simulink model "SIM_EXO_DAL_MN"  (R2021b)
settings: Solver=VariableStepAuto  StartTime=0.0  StopTime=60  FixedStep=0.0001  RelTol=1e-4
undefined symbols (not defined in the file): b, dq, q, X, Y, Z
libraries: sm_lib x47, nesl_utility x7
(part 8 of 24)

== matlab function SIM_EXO_DAL_MN/Exoesqueleto/Dinámica Directa/Cdq ==
  data: dq input; C_dq output; q input
function C_dq = Cdq(dq,q)
%#codegen
dq1 = dq(1);
dq2 = dq(2);
dq3 = dq(3);
dq4 = dq(4);
dq5 = dq(5);
dq6 = dq(6);

q1 = q(1);
q2 = q(2);
q3 = q(3);
q4 = q(4);
q5 = q(5);
q6 = q(6);
%    This function was generated by the Symbolic Math Toolbox version 9.0.
%    02-Dec-2021 21:04:08

t2 = cos(q2);
t3 = cos(q4);
t4 = cos(q5);
t5 = cos(q6);
t6 = sin(q2);
t7 = sin(q4);
t8 = sin(q5);
t9 = sin(q6);
t10 = q1+q2;
t11 = q4.*2.0;
t12 = q5.*2.0;
t13 = q6.*2.0;
t34 = 9.007199254740992e+15;
t14 = cos(t11);
t15 = cos(t12);
t16 = cos(t13);
t17 = t3.^2;
t18 = t4.^2;
t19 = t5.^2;
t20 = sin(t12);
t21 = sin(t13);
t22 = t7.^2;
t23 = t8.^2;
t24 = t9.^2;
t25 = cos(t10);
t26 = sin(t10);
t32 = t4.*5.110348748545983e-1;
t33 = t8.*5.110348748545983e-1;
t39 = t4.*t7.*8.595599785252598e-1;
t40 = t3.*t9.*8.595599785252598e-1;
t41 = t5.*t7.*8.595599785252598e-1;
t42 = t7.*t8.*8.595599785252598e-1;
t43 = t7.*t9.*8.595599785252598e-1;
t44 = t4.*1.33637579258949e-4;
t45 = t5.*1.33637579258949e-4;
t46 = t8.*1.33637579258949e-4;
t47 = t9.*1.33637579258949e-4;
t48 = t4.*t5.*(-5.110348748545983e-1);
t49 = t3.*t5.*8.595599785252598e-1;
t50 = t8.*6.185538795558e-5;
t53 = t4.*1.35652529206996e-4;
t54 = t8.*1.35652529206996e-4;
t55 = t4.*6.185538795558e-5;
t57 = t4.*7.26350610236655e-5;
t58 = t5.*7.26350610236655e-5;
t59 = t8.*7.26350610236655e-5;
t60 = t9.*7.26350610236655e-5;
t70 = t8.*2.257319918256733e-6;
t71 = t5.*1.744166498897461e-6;
t72 = t9.*4.00912737776847e-7;
t73 = t9.*8.01825475553694e-7;
t74 = t9.*1.744166498897461e-6;
t75 = t5.*1.246862701090643e-6;
t76 = t9.*1.246862701090643e-6;
t77 = t4.*4.20092050615074e-6;
t78 = t4.*5.878412210495409e-7;
t79 = t4.*t9.*(-1.33637579258949e-4);
t80 = t8.*4.20092050615074e-6;
t81 = t8.*5.878412210495409e-7;
t82 = t8.*t9.*(-1.33637579258949e-4);
t83 = t5.*3.383302988283333e-6;
t84 = t9.*3.383302988283333e-6;
t85 = t3.*t5.*t8.*(-8.595599785252598e-1);
t86 = t4.*7.291452964015446e-7;
t87 = t4.*2.257319918256733e-6;
t88 = t7.*t8.*t9.*(-8.595599785252598e-1);
t89 = t8.*7.291452964015446e-7;
t104 = t4.*t5.*4.36041e-5;
t106 = t4.*t9.*4.36041e-5;
t107 = t5.*t8.*4.36041e-5;
t109 = t8.*t9.*4.36041e-5;
t111 = t4.*1.758766830582798e-8;
t112 = t5.*2.179051830709965e-7;
t113 = t5.*4.35810366141993e-7;
t114 = t8.*1.758766830582798e-8;
t115 = t4.*t5.*4.00912737776847e-7;
t116 = t4.*t5.*8.01825475553694e-7;
t118 = t5.*t8.*8.01825475553694e-7;
t122 = t4.*t5.*(-1.246862701090643e-6);
t123 = t4.*t9.*(-1.246862701090643e-6);
t124 = t8.*t9.*(-3.383302988283333e-6);
t126 = t4.*2.524706033578261e-9;
t128 = t8.*2.524706033578261e-9;
t129 = t5.*t8.*(-1.744166498897461e-6);
t130 = t8.*t9.*(-8.01825475553694e-7);
t132 = t4.*t9.*2.179051830709965e-7;
t133 = t4.*t9.*4.35810366141993e-7;
t135 = t8.*t9.*4.35810366141993e-7;
t136 = t4.*t5.*t8.*1.603650951107388e-6;
t139 = t4.*3.146556677756745e-13;
t140 = t5.*3.146556677756745e-13;
t141 = t8.*3.146556677756745e-13;
t142 = t9.*3.146556677756745e-13;
t145 = t4.*t8.*t9.*8.71620732283986e-7;
t147 = t4.*t5.*t8.*t9.*2.493725402181286e-6;
t150 = t4.*4.126305279697715e-13;
t151 = t5.*4.126305279697715e-13;
t153 = t8.*4.126305279697715e-13;
t154 = t9.*4.126305279697715e-13;
t159 = t4.*t5.*1.40259855e-11;
t160 = t4.*t9.*1.40259855e-11;
t161 = t5.*t8.*1.40259855e-11;
t162 = t4.*t8.*5.902365793397849e-7;
t163 = t8.*t9.*1.40259855e-11;
t165 = t8.*t9.*(-3.146556677756745e-13);
t176 = t4.*t9.*(-4.126305279697715e-13);
t177 = t5.*t8.*(-4.126305279697715e-13);
t179 = t4.*t5.*8.4155913e-14;
t180 = t4.*t9.*8.4155913e-14;
t181 = t5.*t8.*8.4155913e-14;
t182 = t8.*t9.*8.4155913e-14;
t187 = (q3.*t34)./4.503599627370496e+15;
t189 = (q3.*t34)./9.007199254740992e+15;
t206 = t8.*6.829346359246847e-5;
t207 = t4.*6.829346359246847e-5;
t215 = t3.*5.316841594276996e-5;
t216 = t7.*5.316841594276996e-5;
t218 = t4.*6.932317328700695e-5;
t219 = t3.*1.166014850920627e-4;
t220 = t8.*6.932317328700695e-5;
t221 = t7.*1.166014850920627e-4;
t222 = t4.*3.161026044296245e-5;
t224 = t3.*t4.*1.148695147579899e-4;
t225 = t3.*t5.*1.148695147579899e-4;
t226 = t8.*3.161026044296245e-5;
t228 = t4.*t7.*1.148695147579899e-4;
t229 = t3.*t9.*1.148695147579899e-4;
t230 = t5.*t7.*1.148695147579899e-4;
t231 = t4.*3.711904932028501e-5;
t233 = t7.*t8.*1.148695147579899e-4;
t234 = t8.*3.711904932028501e-5;
t235 = t4.*2.146816885134859e-6;
t236 = t8.*2.146816885134859e-6;
t237 = t4.*3.004073648334264e-7;
t238 = t8.*3.004073648334264e-7;
t239 = t9.*2.048803907774054e-7;
t240 = t9.*4.097607815548108e-7;
t243 = t8.*t9.*(-6.829346359246847e-5);
t245 = t4.*3.726186752973823e-7;
t247 = t8.*3.726186752973823e-7;
t251 = t4.*3.60334715805357e-7;
t252 = t8.*3.60334715805357e-7;
t255 = t4.*1.153569201933121e-6;
t259 = t8.*1.153569201933121e-6;
t260 = t4.*8.987911871652987e-9;
t261 = t3.*2.28624364216682e-6;
t262 = t8.*8.987911871652987e-9;
t263 = t7.*1.14312182108341e-6;
t264 = t7.*2.28624364216682e-6;
t273 = t4.*t7.*6.243419149368285e-5;
t274 = t3.*t9.*6.243419149368285e-5;
t275 = t7.*t8.*6.243419149368285e-5;
t276 = t7.*t9.*6.243419149368285e-5;
t277 = t5.*1.11357147960855e-7;
t278 = t5.*2.227142959217101e-7;
t279 = t7.*t8.*(-5.316841594276996e-5);
t280 = t4.*t5.*8.913299084896471e-7;
t282 = t4.*t5.*2.048803907774054e-7;
t283 = t4.*t9.*8.913299084896471e-7;
t284 = t5.*t8.*8.913299084896471e-7;
t291 = t4.*t5.*(-3.711904932028501e-5);
t292 = t4.*t7.*t9.*(-1.148695147579899e-4);
t293 = t5.*t7.*t8.*(-1.148695147579899e-4);
t294 = t7.*t8.*t9.*(-1.148695147579899e-4);
t295 = t3.*t4.*6.243419149368285e-5;
t296 = t3.*t5.*6.243419149368285e-5;
t297 = t4.*t9.*1.728985819212562e-6;
t298 = t8.*t9.*1.728985819212562e-6;
t300 = t4.*t5.*t8.*8.195215631096216e-7;
t301 = t4.*t5.*6.371903244127231e-7;
t305 = t4.*t9.*6.371903244127231e-7;
t306 = t5.*t8.*6.371903244127231e-7;
t307 = t3.*t8.*1.940301860461398e-6;
t308 = t4.*t7.*1.940301860461398e-6;
t309 = t3.*t9.*3.446085442739697e-7;
t310 = t5.*t7.*3.446085442739697e-7;
t311 = t8.*t9.*6.371903244127231e-7;
t312 = t7.*t8.*1.940301860461398e-6;
t313 = t3.*t4.*3.610943140053254e-6;
t314 = t4.*t7.*3.610943140053254e-6;
t315 = t7.*t8.*3.610943140053254e-6;
t316 = t3.*t5.*2.908151843953269e-6;
t317 = t3.*t4.*5.052847873416058e-7;
t319 = t3.*t9.*2.908151843953269e-6;
t320 = t5.*t7.*2.908151843953269e-6;
t321 = t4.*t7.*5.052847873416058e-7;
t322 = t3.*t5.*1.07175327657342e-6;
t323 = t7.*t8.*5.052847873416058e-7;
t324 = t3.*t9.*1.07175327657342e-6;
t325 = t5.*t7.*1.07175327657342e-6;
t326 = t3.*t5.*1.49921571833678e-6;
t328 = t7.*t9.*1.07175327657342e-6;
t329 = t3.*t4.*6.267441153167058e-7;
t330 = t3.*t9.*1.49921571833678e-6;
t331 = t3.*t8.*6.267441153167058e-7;
t332 = t4.*t7.*6.267441153167058e-7;
t333 = t7.*t9.*1.49921571833678e-6;
t334 = t7.*t8.*6.267441153167058e-7;
t335 = t3.*1.511765579126689e-8;
t336 = t4.*t5.*1.728985819212562e-6;
t338 = t7.*1.511765579126689e-8;
t339 = t4.*t9.*1.11357147960855e-7;
t341 = t3.*t4.*6.060825118201251e-7;
t342 = t3.*t8.*6.060825118201251e-7;
t343 = t4.*t7.*6.060825118201251e-7;
t345 = t7.*t8.*6.060825118201251e-7;
t350 = t4.*1.608000198040319e-13;
t351 = t4.*1.290212831914316e-9;
t352 = t8.*1.608000198040319e-13;
t354 = t8.*1.290212831914316e-9;
t360 = t3.*2.170136264005124e-9;
t363 = t7.*2.170136264005124e-9;
t372 = t3.*t4.*t5.*3.446085442739697e-7;
t378 = t4.*t7.*t9.*6.892170885479394e-7;
t381 = t4.*t7.*t9.*2.908151843953269e-6;
t385 = t7.*t8.*t9.*2.908151843953269e-6;
t391 = t4.*t5.*t7.*1.49921571833678e-6;
t393 = t5.*t7.*t8.*1.49921571833678e-6;
t394 = t3.*t4.*7.558827895633446e-9;
t399 = t3.*t5.*1.873025744810486e-7;
t400 = t3.*t5.*t8.*(-6.243419149368285e-5);
t402 = t4.*t8.*t9.*4.454285918434201e-7;
t403 = t7.*t9.*1.873025744810486e-7;
t404 = t7.*t8.*t9.*(-6.243419149368285e-5);
t406 = t3.*t8.*t9.*(-3.446085442739697e-7);
t414 = t3.*t5.*t8.*(-1.07175327657342e-6);
t416 = t3.*t5.*t8.*(-1.49921571833678e-6);
t424 = t3.*t4.*(-1.511765579126689e-8);
t426 = t4.*t7.*(-1.511765579126689e-8);
t431 = t3.*t5.*t8.*t9.*7.044680628082447e-7;
t436 = t3.*t4.*t5.*t9.*2.143506553146841e-6;
t437 = t4.*t5.*(-1.608000198040319e-13);
t438 = t4.*t9.*(-1.608000198040319e-13);
t439 = t8.*t9.*(-1.608000198040319e-13);
t443 = t3.*t8.*(-2.170136264005124e-9);
t448 = t3.*t4.*t9.*1.873025744810486e-7;
t450 = t4.*t5.*t7.*3.746051489620971e-7;
t457 = t4.*t5.*t8.*t9.*1.274380648825446e-6;
t458 = t4.*t7.*t8.*t9.*(-6.892170885479394e-7);
t462 = t4.*t5.*7.16776774470491e-12;
t463 = t4.*2.10868590222219e-13;
t464 = t4.*t9.*7.16776774470491e-12;
t465 = t5.*t8.*7.16776774470491e-12;
t466 = t8.*2.10868590222219e-13;
t467 = t3.*t4.*2.7046541903611e-13;
t468 = t3.*t5.*2.7046541903611e-13;
t469 = t8.*t9.*7.16776774470491e-12;
t471 = t4.*t7.*2.7046541903611e-13;
t472 = t3.*t9.*2.7046541903611e-13;
t473 = t5.*t7.*1.35232709518055e-13;
t474 = t5.*t7.*2.7046541903611e-13;
t476 = t7.*t8.*2.7046541903611e-13;
t487 = t3.*t8.*5.347915701547076e-7;
t490 = t4.*t5.*t7.*t8.*t9.*1.408936125616489e-6;
t497 = t3.*t5.*1.205617579517561e-11;
t499 = t3.*t9.*1.205617579517561e-11;
t500 = t5.*t7.*1.205617579517561e-11;
t501 = t7.*t9.*1.205617579517561e-11;
t517 = t4.*t8.*3.016314764575132e-7;
t526 = t3.*t4.*3.546806877605634e-13;
t527 = t3.*t5.*3.546806877605634e-13;
t528 = t4.*t7.*3.546806877605634e-13;
t529 = t3.*t9.*3.546806877605634e-13;
t534 = t7.*t8.*3.546806877605634e-13;
t535 = t7.*t9.*1.773403438802817e-13;
t536 = t7.*t9.*3.546806877605634e-13;
t540 = t3.*t4.*t5.*1.35232709518055e-13;
t541 = t3.*t8.*t9.*1.35232709518055e-13;
t556 = t4.*t5.*(-2.10868590222219e-13);
t558 = t5.*t8.*(-2.10868590222219e-13);
t559 = t4.*t7.*t8.*t9.*5.4093083807222e-13;
t560 = t3.*t8.*t9.*(-2.7046541903611e-13);
t562 = t4.*t7.*t9.*(-2.7046541903611e-13);
t564 = t3.*t4.*t9.*1.773403438802817e-13;
t565 = t3.*t5.*t8.*1.773403438802817e-13;
t570 = t3.*t5.*t8.*(-1.205617579517561e-11);
t571 = t4.*t5.*t7.*(-1.205617579517561e-11);
t573 = t4.*t7.*t9.*(-1.205617579517561e-11);
t574 = t5.*t7.*t8.*(-1.205617579517561e-11);
t576 = t7.*t8.*t9.*(-1.205617579517561e-11);
t591 = t3.*t5.*t8.*(-3.546806877605634e-13);
t593 = t4.*t5.*t7.*(-3.546806877605634e-13);
t595 = t7.*t8.*t9.*(-3.546806877605634e-13);
t596 = t4.*t8.*t9.*(-2.10868590222219e-13);
t605 = t4.*t5.*t7.*t8.*7.093613755211269e-13;
t625 = t4.*t7.*t8.*1.253488085959302e-6;
t655 = t3.*2.625549359694895e-3;
t656 = t7.*2.625549359694895e-3;
t659 = t4.*1.560969940408669e-3;
t660 = t8.*1.560969940408669e-3;
t662 = t2.*t4.*1.324388487819695e-2;
t663 = t2.*t8.*1.324388487819695e-2;
t664 = t4.*t6.*1.324388487819695e-2;
t666 = t6.*t8.*1.324388487819695e-2;
t668 = t2.*t3.*2.227619671697157e-2;
t670 = t3.*t6.*2.227619671697157e-2;
t671 = t6.*t7.*2.227619671697157e-2;
t672 = t2.*t4.*5.463144604697158e-2;
t673 = t2.*t8.*5.463144604697158e-2;
t674 = t4.*t6.*5.463144604697158e-2;
t675 = t6.*t8.*5.463144604697158e-2;
t682 = t2.*t3.*9.189001945180305e-2;
t685 = t2.*t7.*9.189001945180305e-2;
t686 = t3.*t6.*9.189001945180305e-2;
t713 = t2.*t4.*t7.*2.227619671697157e-2;
t717 = t2.*t7.*t8.*2.227619671697157e-2;
t724 = t9.*2.094020497221851e-7;
t725 = t3.*5.363539617571206e-4;
t727 = t7.*5.363539617571206e-4;
t728 = t3.*t5.*(-2.625549359694895e-3);
t735 = t4.*t5.*(-1.560969940408669e-3);
t736 = t4.*t9.*(-1.560969940408669e-3);
t746 = t5.*t6.*t8.*(-1.324388487819695e-2);
t752 = t6.*t8.*t9.*(-1.324388487819695e-2);
t756 = t4.*t6.*t7.*9.189001945180305e-2;
t759 = t3.*t4.*t6.*(-2.227619671697157e-2);
t761 = t6.*t7.*t8.*9.189001945180305e-2;
t763 = t3.*t6.*t8.*(-2.227619671697157e-2);
t764 = t4.*t6.*t7.*(-2.227619671697157e-2);
t765 = t3.*t6.*t9.*(-2.227619671697157e-2);
t766 = t5.*t6.*t7.*(-2.227619671697157e-2);
t768 = t6.*t7.*t8.*(-2.227619671697157e-2);
t769 = t6.*t7.*t9.*(-2.227619671697157e-2);
t770 = t5.*t9.*4.280713835074992e-7;
t780 = t2.*t4.*t5.*(-5.463144604697158e-2);
t785 = t2.*t4.*t9.*(-5.463144604697158e-2);
t786 = t4.*t5.*t6.*(-5.463144604697158e-2);
t787 = t3.*3.050168925520967e-6;
t788 = t7.*3.050168925520967e-6;
t789 = t5.*1.138147723446811e-7;
t791 = t3.*6.689201101650821e-6;
t793 = t7.*6.689201101650821e-6;
t795 = t2.*t4.*t5.*(-1.324388487819695e-2);
t804 = t2.*t3.*t5.*(-9.189001945180305e-2);
t814 = t9.*5.924234258315089e-7;
t827 = t3.*t5.*3.294920660995711e-6;
t828 = t5.*t9.*1.211065105878372e-6;
t840 = t2.*t7.*t8.*t9.*(-2.227619671697157e-2);
t849 = t3.*t8.*(-5.363539617571206e-4);
t882 = t3.*t4.*7.725649335384969e-9;
t883 = t3.*t4.*7.725649335384969e-9;
t884 = t3.*t5.*t7.*4.188040994443703e-7;
t885 = t3.*t4.*t5.*3.522139685937468e-7;
t886 = t3.*t4.*t5.*3.522139685937468e-7;
t887 = t5.*3.219955937973119e-7;
t888 = t6.*t7.*t8.*t9.*(-9.189001945180305e-2);
t891 = t7.*t8.*7.725649335384969e-9;
t892 = t7.*t8.*7.725649335384969e-9;
t895 = t3.*t8.*t9.*3.522139685937468e-7;
t896 = t3.*t8.*t9.*3.522139685937468e-7;
t897 = t4.*t7.*t9.*3.522139685937468e-7;
t898 = t4.*t7.*t9.*3.522139685937468e-7;
t899 = t3.*t9.*1.79086425095906e-6;
t900 = t4.*t5.*t8.*7.660427522186475e-7;
t901 = t4.*t5.*t8.*7.660427522186475e-7;
t904 = t3.*t8.*(-3.050168925520967e-6);
t911 = t4.*t5.*t7.*3.294920660995711e-6;
t918 = t7.*t8.*t9.*3.294920660995711e-6;
t942 = t3.*t5.*t7.*t9.*1.302505910779267e-6;
t946 = t3.*t7.*t9.*2.276295446893622e-7;
t959 = t3.*t5.*t7.*1.184846851663018e-6;
t962 = t4.*t5.*t8.*t9.*1.191219491402018e-6;
t964 = t3.*t4.*t5.*t9.*2.190813206274814e-6;
t969 = t4.*t7.*t8.*t9.*7.044279371874937e-7;
t970 = t4.*t7.*t8.*t9.*7.044279371874937e-7;
t971 = t4.*t7.*t9.*1.79086425095906e-6;
t972 = t5.*t7.*t8.*1.79086425095906e-6;
t977 = t3.*t5.*t8.*t9.*7.200154966325453e-7;
t978 = t3.*t5.*t8.*t9.*7.200154966325453e-7;
t979 = t4.*t5.*t7.*t9.*7.200154966325453e-7;
t980 = t4.*t5.*t7.*t9.*7.200154966325453e-7;
t982 = t3.*t7.*t8.*4.593136418534343e-9;
t986 = t4.*t7.*1.075087193219284e-6;
t997 = t3.*t4.*3.476977846858022e-8;
t1001 = t3.*t8.*3.476977846858022e-8;
t1002 = t4.*t7.*3.476977846858022e-8;
t1005 = t7.*t8.*3.476977846858022e-8;
t1023 = t3.*t4.*t7.*t9.*2.094020497221851e-7;
t1024 = t3.*t5.*t7.*t8.*2.094020497221851e-7;
t1026 = t3.*t4.*t5.*t8.*7.044279371874937e-7;
t1027 = t3.*t4.*t5.*t8.*7.044279371874937e-7;
t1037 = t3.*t4.*t5.*t9.*2.190813206274814e-6;
t1044 = t3.*t4.*t5.*t7.*1.138147723446811e-7;
t1047 = t3.*t7.*t8.*t9.*1.138147723446811e-7;
t1050 = t3.*t7.*t8.*1.299453188729364e-8;
t1059 = t4.*t8.*t9.*4.163616429052617e-7;
t1060 = t4.*t8.*t9.*4.163616429052617e-7;
t1066 = t3.*t4.*t9.*1.914362954197335e-7;
t1067 = t3.*t4.*t9.*1.914362954197335e-7;
t1068 = t3.*t5.*t8.*1.914362954197335e-7;
t1069 = t3.*t5.*t8.*1.914362954197335e-7;
t1070 = t4.*t5.*t7.*1.914362954197335e-7;
t1071 = t4.*t5.*t7.*1.914362954197335e-7;
t1078 = t3.*t9.*1.38217261569615e-13;
t1079 = t3.*t9.*1.38217261569615e-13;
t1080 = t5.*t7.*1.38217261569615e-13;
t1081 = t5.*t7.*1.38217261569615e-13;
t1100 = t4.*t5.*t7.*t8.*t9.*1.440030993265091e-6;
t1101 = t4.*t5.*t7.*t8.*t9.*1.440030993265091e-6;
t1109 = t3.*t8.*5.465942862546103e-7;
t1110 = t3.*t8.*5.465942862546103e-7;
t1111 = t4.*t7.*5.465942862546103e-7;
t1112 = t4.*t7.*5.465942862546103e-7;
t1139 = t3.*t4.*t8.*t9.*3.828725908394669e-7;
t1140 = t3.*t4.*t8.*t9.*3.828725908394669e-7;
t1141 = t4.*t5.*t7.*t8.*3.828725908394669e-7;
t1142 = t4.*t5.*t7.*t8.*3.828725908394669e-7;
t1143 = t3.*t5.*t7.*t9.*3.684944893583304e-6;
t1154 = t3.*t4.*t7.*t9.*5.924234258315089e-7;
t1155 = t3.*t5.*t7.*t8.*5.924234258315089e-7;
t1158 = t4.*t7.*2.600171655979768e-6;
t1160 = t3.*t7.*t9.*6.439911875946239e-7;
t1167 = t3.*t4.*t5.*t7.*t9.*(-4.280713835074992e-7);
t1168 = t4.*t5.*t8.*t9.*1.191219491402018e-6;
t1169 = t3.*t4.*t5.*t8.*t9.*1.095406603137407e-6;
t1196 = t3.*t4.*t5.*t7.*t9.*(-1.211065105878372e-6);
t1204 = t3.*t4.*t5.*1.38217261569615e-13;
t1205 = t3.*t4.*t5.*1.38217261569615e-13;
t1229 = t3.*t4.*t5.*t8.*t9.*1.095406603137407e-6;
t1248 = t3.*t7.*1.035461175802946e-6;
t1250 = t3.*t4.*t5.*t7.*3.219955937973119e-7;
t1258 = t3.*t7.*t8.*t9.*3.219955937973119e-7;
t1259 = t3.*t8.*t9.*(-1.38217261569615e-13);
t1260 = t5.*t7.*t8.*(-1.38217261569615e-13);
t1261 = t5.*t7.*t8.*(-1.38217261569615e-13);
t1266 = t3.*t4.*t7.*3.249671339417237e-7;
t1272 = t4.*t8.*2.81948171692439e-7;
t1273 = t4.*t8.*2.81948171692439e-7;
t1282 = t7.*t8.*3.458197138188697e-13;
t1284 = t4.*t5.*t8.*1.503068317813338e-13;
t1285 = t4.*t5.*t8.*1.503068317813338e-13;
t1291 = t3.*t4.*t7.*9.193708611153409e-7;
t1302 = t4.*t7.*t8.*t9.*5.528690462784599e-13;
t1303 = t4.*t7.*t8.*t9.*5.528690462784599e-13;
t1304 = t3.*t5.*1.812542008830624e-13;
t1305 = t3.*t5.*1.812542008830624e-13;
t1307 = t3.*t4.*t7.*t9.*8.217441799717035e-14;
t1308 = t3.*t5.*t7.*t8.*8.217441799717035e-14;
t1313 = t7.*t9.*1.812542008830624e-13;
t1314 = t7.*t9.*1.812542008830624e-13;
t1332 = t3.*t7.*2.929443421869778e-6;
t1335 = t3.*t4.*t8.*2.592703454263624e-7;
t1336 = t3.*t4.*t8.*2.592703454263624e-7;
t1360 = t4.*t8.*t9.*1.97108120739817e-13;
t1361 = t4.*t8.*t9.*1.97108120739817e-13;
t1362 = t3.*t4.*t9.*1.812542008830624e-13;
t1363 = t3.*t4.*t9.*1.812542008830624e-13;
t1367 = t3.*t4.*t7.*t8.*t9.*1.643488359943407e-13;
t1371 = t3.*t4.*t5.*t7.*1.077612036149773e-13;
t1374 = t3.*t7.*t8.*t9.*1.077612036149773e-13;
t1380 = t3.*t4.*t7.*t9.*2.324812497785041e-13;
t1381 = t3.*t5.*t7.*t8.*2.324812497785041e-13;
t1389 = t4.*t5.*t7.*t8.*7.250168035322496e-13;
t1390 = t4.*t5.*t7.*t8.*7.250168035322496e-13;
t1393 = t3.*t5.*t8.*(-1.812542008830624e-13);
t1400 = t3.*t4.*t7.*t8.*t9.*4.649624995570082e-13;
t1409 = t3.*t4.*t5.*t7.*3.048693243547943e-13;
t1411 = t3.*t7.*t8.*t9.*3.048693243547943e-13;
t1416 = t3.*t4.*t5.*t7.*t8.*2.155224072299545e-13;
t1437 = t3.*t4.*t5.*t7.*t8.*6.097386487095885e-13;
t1449 = t7.*t8.*3.344600205005697e-6;
t1456 = t4.*t7.*t8.*1.281152254279884e-6;
t1457 = t4.*t7.*t8.*1.281152254279884e-6;
t1477 = t3.*t4.*t7.*t8.*3.808422322424164e-7;
t1485 = t3.*t4.*t7.*t8.*1.077448192248847e-6;
t1504 = t4.*2.086042441322004e-7;
t1505 = t8.*2.086042441322004e-7;
t1532 = t2.*t8.*1.769880715106441e-6;
t1533 = t4.*t6.*1.769880715106441e-6;
t1535 = t6.*t8.*1.769880715106441e-6;
t1547 = t4.*9.655440125097679e-8;
t1549 = t8.*9.655440125097679e-8;
t1552 = t4.*1.134411489642894e-5;
t1554 = t4.*1.133811468776912e-7;
t1558 = t8.*1.134411489642894e-5;
t1559 = t4.*2.117495204325297e-7;
t1560 = t8.*1.133811468776912e-7;
t1563 = t8.*2.117495204325297e-7;
t1596 = t2.*t4.*t9.*1.769880715106441e-6;
t1604 = t2.*t4.*7.30081420113316e-6;
t1606 = t4.*t5.*(-2.086042441322004e-7);
t1608 = t2.*t8.*7.30081420113316e-6;
t1610 = t6.*t8.*7.30081420113316e-6;
t1611 = t8.*t9.*(-2.086042441322004e-7);
t1612 = t8.*t9.*1.043021220661002e-7;
t1619 = t7.*4.911624408131596e-10;
t1631 = t3.*t4.*1.908078613917869e-5;
t1632 = t3.*t5.*1.908078613917869e-5;
t1637 = t4.*t7.*1.908078613917869e-5;
t1638 = t3.*t9.*1.908078613917869e-5;
t1639 = t5.*t7.*1.908078613917869e-5;
t1644 = t7.*t8.*1.908078613917869e-5;
t1645 = t7.*t9.*1.908078613917869e-5;
t1651 = t2.*t4.*t9.*8.849403575532204e-7;
t1652 = t3.*t4.*3.508720606545093e-7;
t1653 = t3.*t5.*3.508720606545093e-7;
t1654 = t3.*t5.*3.367638735295547e-6;
t1657 = t4.*t6.*t9.*(-1.769880715106441e-6);
t1658 = t4.*t7.*3.508720606545093e-7;
t1659 = t3.*t9.*1.754360303272547e-7;
C_dq = ft_1({dq1,dq2,dq3,dq4,dq5,dq6,t1001,t1002,t1005,t1023,t1024,t1026,t1027,t1037,t104,t1044,t1047,t1050,t1059,t106,t1060,t1066,t1067,t1068,t1069,t107,t1070,t1071,t1078,t1079,t1080,t1081,t109,t1100,t1101,t1109,t111,t1110,t1111,t1112,t112,t113,t1139,t114,t1140,t1141,t1142,t1143,t115,t1154,t1155,t1158,t116,t1160,t1167,t1168,t1169,t118,t1196,t1204,t1205,t122,t1229,t123,t124,t1248,t1250,t1258,t1259,t126,t1260,t1261,t1266,t1272,t1273,t128,t1282,t1284,t1285,t129,t1291,t130,t1302,t1303,t1304,t1305,t1307,t1308,t1313,t1314,t132,t133,t1332,t1335,t1336,t135,t136,t1360,t1361,t1362,t1363,t1367,t1371,t1374,t1380,t1381,t1389,t139,t1390,t1393,t14,t140,t1400,t1409,t141,t1411,t1416,t142,t1437,t1449,t145,t1456,t1457,t147,t1477,t1485,t15,t150,t1504,t1505,t151,t153,t1532,t1533,t1535,t154,t1547,t1549,t1552,t1554,t1558,t1559,t1560,t1563,t159,t1596,t16,t160,t1604,t1606,t1608,t161,t1610,t1611,t1612,t1619,t162,t163,t1631,t1632,t1637,t1638,t1639,t1644,t1645,t165,t1651,t1652,t1653,t1654,t1657,t1658,t1659,t17,t176,t177,t179,t18,t180,t181,t182,t187,t189,t19,t2,t20,t206,t207,t21,t215,t216,t218,t219,t22,t220,t221,t222,t224,t225,t226,t228,t229,t23,t230,t231,t233,t234,t235,t236,t237,t238,t239,t24,t240,t243,t245,t247,t25,t251,t252,t255,t259,t26,t260,t261,t262,t263,t264,t273,t274,t275,t276,t277,t278,t279,t280,t282,t283,t284,t291,t292,t293,t294,t295,t296,t297,t298,t3,t300,t301,t305,t306,t307,t308,t309,t310,t311,t312,t313,t314,t315,t316,t317,t319,t32,t320,t321,t322,t323,t324,t325,t326,t328,t329,t33,t330,t331,t332,t333,t334,t335,t336,t338,t339,t34,t341,t342,t343,t345,t350,t351,t352,t354,t360,t363,t372,t378,t381,t385,t39,t391,t393,t394,t399,t4,t40,t400,t402,t403,t404,t406,t41,t414,t416,t42,t424,t426,t43,t431,t436,t437,t438,t439,t44,t443,t448,t45,t450,t457,t458,t46,t462,t463,t464,t465,t466,t467,t468,t469,t47,t471,t472,t473,t474,t476,t48,t487,t49,t490,t497,t499,t5,t50,t500,t501,t517,t526,t527,t528,t529,t53,t534,t535,t536,t54,t540,t541,t55,t556,t558,t559,t560,t562,t564,t565,t57,t570,t571,t573,t574,t576,t58,t59,t591,t593,t595,t596,t6,t60,t605,t625,t655,t656,t659,t660,t662,t663,t664,t666,t668,t670,t671,t672,t673,t674,t675,t682,t685,t686,t7,t70,t71,t713,t717,t72,t724,t725,t727,t728,t73,t735,t736,t74,t746,t75,t752,t756,t759,t76,t761,t763,t764,t765,t766,t768,t769,t77,t770,t78,t780,t785,t786,t787,t788,t789,t79,t791,t793,t795,t8,t80,t804,t81,t814,t82,t827,t828,t83,t84,t840,t849,t85,t86,t87,t88,t882,t883,t884,t885,t886,t887,t888,t89,t891,t892,t895,t896,t897,t898,t899,t9,t900,t901,t904,t911,t918,t942,t946,t959,t962,t964,t969,t970,t971,t972,t977,t978,t979,t980,t982,t986,t997});
end
function C_dq = ft_1(ct)
dq1 = ct{1};
dq2 = ct{2};
dq3 = ct{3};
dq4 = ct{4};
dq5 = ct{5};
dq6 = ct{6};
t1001 = ct{7};
t1002 = ct{8};
t1005 = ct{9};
t1023 = ct{10};
t1024 = ct{11};
t1026 = ct{12};
t1027 = ct{13};
t1037 = ct{14};
t104 = ct{15};
t1044 = ct{16};
t1047 = ct{17};
t1050 = ct{18};
t1059 = ct{19};
t106 = ct{20};
t1060 = ct{21};
t1066 = ct{22};
t1067 = ct{23};
t1068 = ct{24};
t1069 = ct{25};
t107 = ct{26};
t1070 = ct{27};
t1071 = ct{28};
t1078 = ct{29};
t1079 = ct{30};
t1080 = ct{31};
t1081 = ct{32};
t109 = ct{33};
t1100 = ct{34};
t1101 = ct{35};
t1109 = ct{36};
t111 = ct{37};
t1110 = ct{38};
t1111 = ct{39};
t1112 = ct{40};
t112 = ct{41};
t113 = ct{42};
t1139 = ct{43};
t114 = ct{44};
t1140 = ct{45};
t1141 = ct{46};
t1142 = ct{47};
t1143 = ct{48};
t115 = ct{49};
t1154 = ct{50};
t1155 = ct{51};
t1158 = ct{52};
t116 = ct{53};
t1160 = ct{54};
t1167 = ct{55};
t1168 = ct{56};
t1169 = ct{57};
t118 = ct{58};
t1196 = ct{59};
t1204 = ct{60};
t1205 = ct{61};
t122 = ct{62};
t1229 = ct{63};
t123 = ct{64};
t124 = ct{65};
t1248 = ct{66};
t1250 = ct{67};
t1258 = ct{68};
t1259 = ct{69};
t126 = ct{70};
t1260 = ct{71};
t1261 = ct{72};
t1266 = ct{73};
t1272 = ct{74};
t1273 = ct{75};
t128 = ct{76};
t1282 = ct{77};
t1284 = ct{78};
t1285 = ct{79};
t129 = ct{80};
t1291 = ct{81};
t130 = ct{82};
t1302 = ct{83};
t1303 = ct{84};
t1304 = ct{85};
t1305 = ct{86};
t1307 = ct{87};
t1308 = ct{88};
t1313 = ct{89};
t1314 = ct{90};
t132 = ct{91};
t133 = ct{92};
t1332 = ct{93};
t1335 = ct{94};
t1336 = ct{95};
t135 = ct{96};
t136 = ct{97};
t1360 = ct{98};
t1361 = ct{99};
t1362 = ct{100};
t1363 = ct{101};
t1367 = ct{102};
t1371 = ct{103};
t1374 = ct{104};
t1380 = ct{105};
t1381 = ct{106};
t1389 = ct{107};
t139 = ct{108};
t1390 = ct{109};
t1393 = ct{110};
t14 = ct{111};
t140 = ct{112};
t1400 = ct{113};
t1409 = ct{114};
t141 = ct{115};
t1411 = ct{116};
t1416 = ct{117};
t142 = ct{118};
t1437 = ct{119};
t1449 = ct{120};
t145 = ct{121};
t1456 = ct{122};
t1457 = ct{123};
t147 = ct{124};
t1477 = ct{125};
t1485 = ct{126};
t15 = ct{127};
t150 = ct{128};
t1504 = ct{129};
t1505 = ct{130};
t151 = ct{131};
t153 = ct{132};
t1532 = ct{133};
t1533 = ct{134};
t1535 = ct{135};
t154 = ct{136};
t1547 = ct{137};
t1549 = ct{138};
t1552 = ct{139};
t1554 = ct{140};
t1558 = ct{141};
t1559 = ct{142};
t1560 = ct{143};
t1563 = ct{144};
t159 = ct{145};
t1596 = ct{146};
t16 = ct{147};
t160 = ct{148};
t1604 = ct{149};
t1606 = ct{150};
t1608 = ct{151};
t161 = ct{152};
t1610 = ct{153};
t1611 = ct{154};
t1612 = ct{155};
t1619 = ct{156};
t162 = ct{157};
t163 = ct{158};
t1631 = ct{159};
t1632 = ct{160};
t1637 = ct{161};
t1638 = ct{162};
t1639 = ct{163};
t1644 = ct{164};
t1645 = ct{165};
t165 = ct{166};
t1651 = ct{167};
t1652 = ct{168};
t1653 = ct{169};
t1654 = ct{170};
t1657 = ct{171};
t1658 = ct{172};
t1659 = ct{173};
t17 = ct{174};
t176 = ct{175};
t177 = ct{176};
t179 = ct{177};
t18 = ct{178};
t180 = ct{179};
t181 = ct{180};
t182 = ct{181};
t187 = ct{182};
t189 = ct{183};
t19 = ct{184};
t2 = ct{185};
t20 = ct{186};
t206 = ct{187};
t207 = ct{188};
t21 = ct{189};
t215 = ct{190};
t216 = ct{191};
t218 = ct{192};
t219 = ct{193};
t22 = ct{194};
t220 = ct{195};
t221 = ct{196};
t222 = ct{197};
t224 = ct{198};
t225 = ct{199};
t226 = ct{200};
t228 = ct{201};
t229 = ct{202};
t23 = ct{203};
t230 = ct{204};
t231 = ct{205};
t233 = ct{206};
t234 = ct{207};
t235 = ct{208};
t236 = ct{209};
t237 = ct{210};
t238 = ct{211};
t239 = ct{212};
t24 = ct{213};
t240 = ct{214};
t243 = ct{215};
t245 = ct{216};
t247 = ct{217};
t25 = ct{218};
t251 = ct{219};
t252 = ct{220};
t255 = ct{221};
t259 = ct{222};
t26 = ct{223};
t260 = ct{224};
t261 = ct{225};
t262 = ct{226};
t263 = ct{227};
t264 = ct{228};
t273 = ct{229};
t274 = ct{230};
t275 = ct{231};
t276 = ct{232};
t277 = ct{233};
t278 = ct{234};
t279 = ct{235};
t280 = ct{236};
t282 = ct{237};
t283 = ct{238};
t284 = ct{239};
t291 = ct{240};
t292 = ct{241};
t293 = ct{242};
t294 = ct{243};
t295 = ct{244};
t296 = ct{245};
t297 = ct{246};
t298 = ct{247};
t3 = ct{248};
t300 = ct{249};
t301 = ct{250};
t305 = ct{251};
t306 = ct{252};
t307 = ct{253};
t308 = ct{254};
t309 = ct{255};
t310 = ct{256};
t311 = ct{257};
t312 = ct{258};
t313 = ct{259};
t314 = ct{260};
t315 = ct{261};
t316 = ct{262};
t317 = ct{263};
t319 = ct{264};
t32 = ct{265};
t320 = ct{266};
t321 = ct{267};
t322 = ct{268};
t323 = ct{269};
t324 = ct{270};
t325 = ct{271};
t326 = ct{272};
t328 = ct{273};
t329 = ct{274};
t33 = ct{275};
t330 = ct{276};
t331 = ct{277};
t332 = ct{278};
t333 = ct{279};
t334 = ct{280};
t335 = ct{281};
t336 = ct{282};
t338 = ct{283};
t339 = ct{284};
t34 = ct{285};
t341 = ct{286};
t342 = ct{287};
t343 = ct{288};
t345 = ct{289};
t350 = ct{290};
t351 = ct{291};
t352 = ct{292};
t354 = ct{293};
t360 = ct{294};
t363 = ct{295};
t372 = ct{296};
t378 = ct{297};
t381 = ct{298};
t385 = ct{299};
t39 = ct{300};
t391 = ct{301};
t393 = ct{302};
t394 = ct{303};
t399 = ct{304};
t4 = ct{305};
t40 = ct{306};
t400 = ct{307};
t402 = ct{308};
t403 = ct{309};
t404 = ct{310};
t406 = ct{311};
t41 = ct{312};
t414 = ct{313};
t416 = ct{314};
t42 = ct{315};
t424 = ct{316};
t426 = ct{317};
t43 = ct{318};
t431 = ct{319};
t436 = ct{320};
t437 = ct{321};
t438 = ct{322};
t439 = ct{323};
t44 = ct{324};
t443 = ct{325};
t448 = ct{326};
t45 = ct{327};
t450 = ct{328};
t457 = ct{329};
t458 = ct{330};
t46 = ct{331};
t462 = ct{332};
t463 = ct{333};
t464 = ct{334};
t465 = ct{335};
t466 = ct{336};
t467 = ct{337};
t468 = ct{338};
t469 = ct{339};
t47 = ct{340};
t471 = ct{341};
t472 = ct{342};
t473 = ct{343};
t474 = ct{344};
t476 = ct{345};
t48 = ct{346};
t487 = ct{347};
t49 = ct{348};
t490 = ct{349};
t497 = ct{350};
t499 = ct{351};
t5 = ct{352};
t50 = ct{353};
t500 = ct{354};
t501 = ct{355};
t517 = ct{356};
t526 = ct{357};
t527 = ct{358};
t528 = ct{359};
t529 = ct{360};
t53 = ct{361};
t534 = ct{362};
t535 = ct{363};
t536 = ct{364};
t54 = ct{365};
t540 = ct{366};
t541 = ct{367};
t55 = ct{368};
t556 = ct{369};
t558 = ct{370};
t559 = ct{371};
t560 = ct{372};
t562 = ct{373};
t564 = ct{374};
t565 = ct{375};
t57 = ct{376};
t570 = ct{377};
t571 = ct{378};
t573 = ct{379};
t574 = ct{380};
t576 = ct{381};
t58 = ct{382};
t59 = ct{383};
t591 = ct{384};
t593 = ct{385};
t595 = ct{386};
t596 = ct{387};
t6 = ct{388};
t60 = ct{389};
t605 = ct{390};
t625 = ct{391};
t655 = ct{392};
t656 = ct{393};
t659 = ct{394};
t660 = ct{395};
t662 = ct{396};
t663 = ct{397};
t664 = ct{398};
t666 = ct{399};
t668 = ct{400};
t670 = ct{401};
t671 = ct{402};
t672 = ct{403};
t673 = ct{404};
t674 = ct{405};
t675 = ct{406};
t682 = ct{407};
t685 = ct{408};
t686 = ct{409};
t7 = ct{410};
t70 = ct{411};
t71 = ct{412};
t713 = ct{413};
t717 = ct{414};
t72 = ct{415};
t724 = ct{416};
t725 = ct{417};
t727 = ct{418};
t728 = ct{419};
t73 = ct{420};
t735 = ct{421};
t736 = ct{422};
t74 = ct{423};
t746 = ct{424};
t75 = ct{425};
t752 = ct{426};
t756 = ct{427};
t759 = ct{428};
t76 = ct{429};
t761 = ct{430};
t763 = ct{431};
t764 = ct{432};
t765 = ct{433};
t766 = ct{434};
t768 = ct{435};
t769 = ct{436};
t77 = ct{437};
t770 = ct{438};
t78 = ct{439};
t780 = ct{440};
t785 = ct{441};
t786 = ct{442};
t787 = ct{443};
t788 = ct{444};
t789 = ct{445};
t79 = ct{446};
t791 = ct{447};
t793 = ct{448};
t795 = ct{449};
t8 = ct{450};
t80 = ct{451};
t804 = ct{452};
t81 = ct{453};
t814 = ct{454};
t82 = ct{455};
t827 = ct{456};
t828 = ct{457};
t83 = ct{458};
t84 = ct{459};
t840 = ct{460};
t849 = ct{461};
t85 = ct{462};
t86 = ct{463};
t87 = ct{464};
t88 = ct{465};
t882 = ct{466};
t883 = ct{467};
t884 = ct{468};
t885 = ct{469};
t886 = ct{470};
t887 = ct{471};
t888 = ct{472};
t89 = ct{473};
t891 = ct{474};
t892 = ct{475};
t895 = ct{476};
t896 = ct{477};
t897 = ct{478};
t898 = ct{479};
t899 = ct{480};
t9 = ct{481};
t900 = ct{482};
t901 = ct{483};
t904 = ct{484};
t911 = ct{485};
t918 = ct{486};
t942 = ct{487};
t946 = ct{488};
t959 = ct{489};
t962 = ct{490};
t964 = ct{491};
t969 = ct{492};
t970 = ct{493};
t971 = ct{494};
t972 = ct{495};
t977 = ct{496};
t978 = ct{497};
t979 = ct{498};
t980 = ct{499};
t982 = ct{500};
t986 = ct{501};
t997 = ct{502};
t1660 = t3.*t9.*3.508720606545093e-7;
t1661 = t5.*t7.*1.754360303272547e-7;
t1662 = t5.*t7.*3.508720606545093e-7;
t1664 = t6.*t8.*t9.*8.849403575532204e-7;
t1666 = t7.*t8.*3.508720606545093e-7;
t1668 = t7.*t9.*3.367638735295547e-6;
t1676 = t4.*t6.*t7.*2.976937004352228e-6;
t1677 = t2.*t7.*t9.*2.976937004352228e-6;
t1678 = t3.*t6.*t9.*2.976937004352228e-6;
t1679 = t5.*t6.*t7.*1.488468502176114e-6;
t1680 = t5.*t6.*t7.*2.976937004352228e-6;
t1682 = t2.*t8.*9.619703863182361e-7;
t1683 = t4.*t6.*9.619703863182361e-7;
t1684 = t6.*t7.*t8.*2.976937004352228e-6;
t1685 = t6.*t7.*4.167215943261981e-9;
t1688 = t6.*t8.*9.619703863182361e-7;
t1689 = t3.*t4.*1.624043742404524e-7;
t1692 = t4.*t9.*5.664363865215817e-6;
t1693 = t5.*t8.*5.664363865215817e-6;
t1694 = t3.*t9.*1.830388176740875e-6;
t1695 = t5.*t7.*1.830388176740875e-6;
t1696 = t4.*t7.*1.624043742404524e-7;
t1698 = t7.*t8.*1.624043742404524e-7;
t1702 = t4.*t9.*6.045309697076603e-6;
t1703 = t5.*t8.*6.045309697076603e-6;
t1709 = t4.*t5.*(-1.134411489642894e-5);
t1712 = t4.*t5.*(-1.133811468776912e-7);
t1713 = t4.*t9.*(-1.134411489642894e-5);
t1714 = t2.*t4.*3.96815841743287e-6;
t1716 = t4.*t9.*(-1.133811468776912e-7);
t1717 = t5.*t8.*5.669057343884558e-8;
t1720 = t2.*t8.*3.96815841743287e-6;
t1722 = t6.*t8.*3.96815841743287e-6;
t1726 = t3.*t8.*3.561624112004214e-7;
t1727 = t4.*t7.*3.561624112004214e-7;
t1729 = t7.*t8.*3.561624112004214e-7;
t1734 = t2.*t8.*t9.*3.65040710056658e-6;
t1736 = t4.*t6.*t9.*3.65040710056658e-6;
t1737 = t4.*t6.*t9.*7.30081420113316e-6;
t1745 = t2.*t3.*t5.*1.488468502176114e-6;
t1746 = t2.*t3.*t5.*2.976937004352228e-6;
t1749 = t2.*t4.*t7.*2.976937004352228e-6;
t1750 = t3.*t4.*t6.*2.976937004352228e-6;
t1751 = t3.*t5.*t6.*2.976937004352228e-6;
t1752 = t2.*t3.*4.167215943261981e-9;
t1785 = t2.*t3.*t4.*1.22799597575967e-5;
t1786 = t2.*t3.*t5.*1.22799597575967e-5;
t1796 = t2.*t4.*t7.*1.22799597575967e-5;
t1797 = t2.*t3.*t9.*1.22799597575967e-5;
t1798 = t2.*t5.*t7.*6.139979878798348e-6;
t1799 = t2.*t5.*t7.*1.22799597575967e-5;
t1800 = t3.*t5.*t6.*6.139979878798348e-6;
t1801 = t3.*t5.*t6.*1.22799597575967e-5;
t1809 = t2.*t7.*t8.*1.22799597575967e-5;
t1810 = t4.*t6.*t7.*1.22799597575967e-5;
t1816 = t3.*t4.*t5.*1.754360303272547e-7;
t1819 = t6.*t7.*t9.*1.22799597575967e-5;
t1827 = t4.*t5.*t7.*3.367638735295547e-6;
t1829 = t2.*t4.*t5.*(-7.30081420113316e-6);
t1833 = t4.*t7.*t9.*1.754360303272547e-7;
t1838 = t3.*t5.*1.016820285479769e-5;
t1840 = t3.*t4.*1.907069379620846e-7;
t1841 = t3.*t5.*9.535346898104229e-8;
t1842 = t3.*t5.*1.907069379620846e-7;
t1849 = t2.*t8.*t9.*(-7.30081420113316e-6);
t1850 = t4.*t7.*1.907069379620846e-7;
t1851 = t3.*t9.*1.907069379620846e-7;
t1852 = t7.*t9.*1.016820285479769e-5;
t1857 = t7.*t8.*1.907069379620846e-7;
t1858 = t7.*t9.*9.535346898104229e-8;
t1859 = t7.*t9.*1.907069379620846e-7;
t1871 = t8.*t9.*3.285763190182237e-6;
t1873 = t4.*t7.*t9.*1.830388176740875e-6;
t1876 = t4.*t5.*3.078710474192051e-6;
t1881 = t2.*t8.*1.396693317797299e-6;
t1882 = t4.*t6.*1.396693317797299e-6;
t1883 = t8.*t9.*3.078710474192051e-6;
t1889 = t3.*t5.*t8.*(-1.908078613917869e-5);
t1895 = t2.*t5.*t8.*1.984079208716435e-6;
t1897 = t4.*t5.*t6.*1.984079208716435e-6;
t1898 = t4.*t5.*t6.*3.96815841743287e-6;
t1907 = t7.*t8.*t9.*(-1.908078613917869e-5);
t1911 = t2.*t4.*t7.*1.618032907912407e-6;
t1912 = t3.*t4.*t6.*1.618032907912407e-6;
t1913 = t2.*t3.*t9.*8.090164539562037e-7;
t1914 = t2.*t3.*t9.*1.618032907912407e-6;
t1915 = t2.*t5.*t7.*1.618032907912407e-6;
t1916 = t3.*t5.*t6.*1.618032907912407e-6;
t1923 = t4.*t6.*t7.*1.618032907912407e-6;
t1924 = t3.*t6.*t9.*1.618032907912407e-6;
t1925 = t2.*t7.*1.718989821069714e-8;
t1926 = t3.*t6.*1.718989821069714e-8;
t1931 = t6.*t7.*t8.*1.618032907912407e-6;
t1932 = t6.*t7.*t9.*8.090164539562037e-7;
t1933 = t6.*t7.*t9.*1.618032907912407e-6;
t1935 = t4.*t7.*t9.*(-3.508720606545093e-7);
t1939 = t7.*t8.*t9.*(-3.508720606545093e-7);
t1948 = t2.*t4.*t5.*4.809851931591181e-7;
t1949 = t2.*t4.*t5.*9.619703863182361e-7;
t1956 = t2.*t7.*t8.*t9.*1.488468502176114e-6;
t1958 = t3.*t6.*t8.*t9.*1.488468502176114e-6;
t1960 = t4.*t6.*t7.*t9.*1.488468502176114e-6;
t1963 = t4.*t5.*3.285763190182237e-6;
t1968 = t5.*t6.*t8.*4.809851931591181e-7;
t1977 = t5.*t7.*t8.*(-1.830388176740875e-6);
t1978 = t3.*t9.*5.526649307438591e-6;
t1979 = t5.*t7.*5.526649307438591e-6;
t1994 = t2.*t4.*t5.*(-3.96815841743287e-6);
t1995 = t2.*t3.*t8.*t9.*6.139979878798348e-6;
t1997 = t2.*t4.*t7.*t9.*6.139979878798348e-6;
t2003 = t2.*t4.*t9.*(-3.96815841743287e-6);
t2012 = t6.*t7.*t8.*t9.*6.139979878798348e-6;
t2022 = t3.*4.452917654948397e-7;
t2024 = t4.*t5.*t7.*1.016820285479769e-5;
t2025 = t8.*4.470006985551917e-6;
t2028 = t3.*t4.*t9.*9.535346898104229e-8;
t2032 = t4.*t5.*t7.*9.535346898104229e-8;
t2046 = t2.*t4.*5.761404326386517e-6;
t2056 = t3.*t4.*t5.*t6.*(-2.976937004352228e-6);
t2058 = t6.*t8.*5.761404326386517e-6;
t2063 = t2.*t3.*t4.*6.674437170347525e-6;
t2064 = t2.*t3.*t5.*6.674437170347525e-6;
t2065 = t2.*t7.*t8.*t9.*(-2.976937004352228e-6);
t2067 = t3.*t6.*t8.*t9.*(-2.976937004352228e-6);
t2070 = t5.*t6.*t7.*t8.*(-2.976937004352228e-6);
t2072 = t2.*t4.*t7.*6.674437170347525e-6;
t2073 = t2.*t3.*t9.*6.674437170347525e-6;
t2079 = t5.*t6.*t8.*(-9.619703863182361e-7);
t2081 = t2.*t7.*t8.*6.674437170347525e-6;
t2082 = t4.*t6.*t7.*6.674437170347525e-6;
t2083 = t2.*t7.*t9.*3.337218585173762e-6;
t2084 = t2.*t7.*t9.*6.674437170347525e-6;
t2085 = t3.*t6.*t9.*3.337218585173762e-6;
t2086 = t3.*t6.*t9.*6.674437170347525e-6;
t2087 = t5.*t6.*t7.*6.674437170347525e-6;
t2093 = t8.*4.770628656414461e-6;
t2094 = t3.*t4.*2.768890910755245e-7;
t2098 = t7.*t8.*2.768890910755245e-7;
t2100 = t2.*t4.*t7.*t9.*(-1.22799597575967e-5);
t2103 = t7.*1.422428293644824e-6;
t2104 = t2.*t7.*t8.*t9.*(-1.22799597575967e-5);
t2105 = t2.*t7.*3.778031034908185e-6;
t2106 = t3.*t6.*3.778031034908185e-6;
t2110 = t2.*t5.*t7.*t8.*8.090164539562037e-7;
t2113 = t3.*t5.*t6.*t8.*8.090164539562037e-7;
t2115 = t4.*t5.*t6.*t7.*8.090164539562037e-7;
t2117 = t6.*t7.*t8.*t9.*(-1.22799597575967e-5);
t2131 = t3.*t5.*t8.*(-1.907069379620846e-7);
t2132 = t3.*t5.*t8.*(-9.535346898104229e-8);
t2144 = t7.*t8.*t9.*(-1.016820285479769e-5);
t2156 = t7.*1.005302486347477e-5;
t2171 = t2.*t3.*t8.*2.349236299369594e-6;
t2172 = t2.*t4.*t7.*2.349236299369594e-6;
t2173 = t3.*t4.*t6.*2.349236299369594e-6;
t2175 = t3.*t4.*t6.*t9.*(-1.618032907912407e-6);
t2176 = t4.*t5.*t6.*t7.*(-1.618032907912407e-6);
t2179 = t3.*t8.*2.657556793628188e-6;
t2180 = t4.*t7.*2.657556793628188e-6;
t2182 = t5.*t6.*t7.*t8.*(-1.618032907912407e-6);
t2183 = t2.*t3.*1.558449809444963e-5;
t2188 = t6.*t7.*t8.*2.349236299369594e-6;
t2189 = t6.*t7.*t8.*t9.*(-1.618032907912407e-6);
t2194 = t6.*t7.*1.558449809444963e-5;
t2205 = t2.*t3.*t5.*t8.*3.337218585173762e-6;
t2207 = t2.*t4.*t5.*t7.*3.337218585173762e-6;
t2220 = t5.*t6.*t7.*t8.*3.337218585173762e-6;
t2223 = t3.*t4.*1.956869039552983e-7;
t2228 = t4.*t7.*t9.*5.526649307438591e-6;
t2265 = t2.*t3.*t5.*t8.*(-6.674437170347525e-6);
t2277 = t4.*t5.*2.189414175010785e-14;
t2279 = t4.*t9.*2.189414175010785e-14;
t2280 = t5.*t8.*2.189414175010785e-14;
t2281 = t3.*t8.*8.02419104298182e-6;
t2282 = t4.*t7.*8.02419104298182e-6;
t2285 = t8.*t9.*2.189414175010785e-14;
t2294 = t3.*3.237047710821912e-7;
t2302 = t2.*t3.*t4.*9.690674399615435e-6;
t2304 = t2.*t7.*t8.*9.690674399615435e-6;
t2305 = t3.*t6.*t8.*9.690674399615435e-6;
t2306 = t4.*t6.*t7.*9.690674399615435e-6;
t2321 = t2.*t4.*t5.*1.857585372652597e-13;
t2322 = t2.*t4.*t9.*1.857585372652597e-13;
t2323 = t4.*t5.*t6.*1.857585372652597e-13;
t2324 = t4.*t6.*t9.*1.857585372652597e-13;
t2325 = t5.*t6.*t8.*1.857585372652597e-13;
t2329 = t6.*t8.*t9.*1.857585372652597e-13;
t2336 = t3.*t5.*3.682591724861488e-14;
t2339 = t3.*t9.*3.682591724861488e-14;
t2340 = t5.*t7.*3.682591724861488e-14;
t2344 = t7.*t9.*3.682591724861488e-14;
t2348 = t2.*t3.*t5.*3.124456121473909e-13;
t2349 = t2.*t3.*t9.*3.124456121473909e-13;
t2350 = t3.*t5.*t6.*3.124456121473909e-13;
t2352 = t3.*t6.*t9.*3.124456121473909e-13;
t2353 = t5.*t6.*t7.*3.124456121473909e-13;
t2356 = t6.*t7.*t9.*3.124456121473909e-13;
t2360 = t2.*t4.*t5.*7.662598700988556e-13;
t2361 = t2.*t4.*t9.*7.662598700988556e-13;
t2362 = t2.*t5.*t8.*7.662598700988556e-13;
t2363 = t4.*t5.*t6.*7.662598700988556e-13;
t2364 = t2.*t8.*t9.*7.662598700988556e-13;
t2365 = t4.*t6.*t9.*7.662598700988556e-13;
t2373 = t3.*3.332244280922431e-7;
t2375 = t2.*t3.*t5.*1.288848080425708e-12;
t2376 = t2.*t3.*t9.*1.288848080425708e-12;
t2377 = t2.*t5.*t7.*1.288848080425708e-12;
t2378 = t3.*t5.*t6.*1.288848080425708e-12;
t2379 = t2.*t7.*t9.*1.288848080425708e-12;
t2380 = t3.*t6.*t9.*1.288848080425708e-12;
t2409 = t2.*t5.*t7.*t8.*3.124456121473909e-13;
t2412 = t2.*t7.*t8.*t9.*3.124456121473909e-13;
t2428 = t3.*t5.*t8.*(-3.682591724861488e-14);
t2429 = t5.*t7.*t8.*(-3.682591724861488e-14);
t2430 = t7.*t8.*t9.*(-3.682591724861488e-14);
t2432 = t5.*t6.*t7.*t8.*1.288848080425708e-12;
t2433 = t6.*t7.*t8.*t9.*1.288848080425708e-12;
t2435 = t4.*t5.*t6.*t7.*(-3.124456121473909e-13);
t2436 = t2.*t4.*1.796566294495167e-6;
t2438 = t3.*t6.*t8.*t9.*(-3.124456121473909e-13);
t2439 = t4.*t6.*t7.*t9.*(-3.124456121473909e-13);
t2440 = t5.*t6.*t7.*t8.*(-3.124456121473909e-13);
t2441 = t6.*t7.*t8.*t9.*(-3.124456121473909e-13);
t2443 = t6.*t8.*1.796566294495167e-6;
t2456 = t2.*t7.*t8.*t9.*(-1.288848080425708e-12);
t2470 = t2.*t3.*t5.*t8.*(-1.288848080425708e-12);
t2474 = t4.*5.749768960780553e-6;
t2475 = t2.*t8.*7.410893064247368e-6;
t2476 = t4.*t6.*7.410893064247368e-6;
t2481 = t7.*t8.*3.4184146944075e-6;
t2486 = t3.*t8.*1.780811871872521e-7;
t2487 = t3.*t8.*3.561623743745041e-7;
t2488 = t4.*t7.*3.561623743745041e-7;
t2489 = t4.*6.136458547094482e-6;
t2491 = t3.*t4.*3.4184146944075e-6;
t2493 = t2.*t3.*t4.*3.021822113324163e-6;
t2495 = t2.*t7.*t8.*3.021822113324163e-6;
t2496 = t3.*t6.*t8.*3.021822113324163e-6;
t2497 = t4.*t6.*t7.*3.021822113324163e-6;
t2516 = t3.*t4.*1.032151509906725e-5;
t2521 = t7.*t8.*1.032151509906725e-5;
t2527 = t2.*t3.*t8.*1.246511225866906e-5;
t2528 = t2.*t4.*t7.*1.246511225866906e-5;
t2529 = t3.*t4.*t6.*1.246511225866906e-5;
t2533 = t6.*t7.*t8.*1.246511225866906e-5;
t2886 = t6.*1.410504133294943e-4;
t2953 = t2.*4.897880306001738e-4;
t27 = t26.*7.742227997977903e+15;
t28 = t25.*4.602992943936994e+15;
t29 = t26.*4.602992943936994e+15;
t30 = t25.*7.742227997977903e+15;
t35 = t9.*t33;
t36 = t5.*t32;
t37 = t9.*t32;
t38 = t5.*t33;
t51 = -t42;
t52 = -t47;
t56 = -t50;
t61 = t5.*t44;
t62 = t9.*t44;
t63 = t9.*t46;
t64 = t8.*t49;
t65 = t5.*t39;
t66 = t8.*t40;
t67 = t9.*t39;
t68 = t8.*t41;
t69 = t9.*t42;
t90 = -t73;
t92 = -t76;
t93 = -t81;
t94 = -t84;
t95 = t5.*t57;
t96 = t9.*t57;
t97 = t8.*t58;
t98 = -t89;
t99 = t4.*t75;
t100 = t4.*t76;
t101 = t8.*t75;
t102 = t8.*t76;
t105 = t4.*t83;
t108 = t4.*t84;
t110 = t8.*t84;
t117 = t4.*t71;
t119 = t4.*t74;
t120 = t8.*t71;
t121 = t8.*t73;
t125 = -t112;
t127 = -t115;
t131 = t18.*t73;
t134 = t8.*t113;
t137 = -t128;
t138 = -t132;
t143 = t4.*t8.*t19.*1.639136489385872e-6;
t144 = t5.*t9.*t18.*1.639136489385872e-6;
t146 = t18.*t19.*1.246862701090643e-6;
t148 = t18.*t24.*1.246862701090643e-6;
t149 = t18.*t113;
t152 = t5.*t139;
t155 = t9.*t139;
t157 = t9.*t141;
t158 = t5.*t18.*(-4.35810366141993e-7);
t164 = -t154;
t166 = t18.*t142;
t167 = t23.*t142;
t168 = t5.*t150;
t169 = t9.*t150;
t170 = t8.*t151;
t172 = -t161;
t173 = -t162;
t174 = -t163;
t175 = t9.*t23.*(-3.146556677756745e-13);
t183 = t18.*t151;
t184 = t23.*t151;
t185 = t8.*t176;
t186 = t5.*t23.*(-4.126305279697715e-13);
t188 = cos(t187);
t190 = cos(t189);
t191 = sin(t189);
t192 = t15.*7.291452122456316e-7;
t223 = t5.*t207;
t227 = t9.*t207;
t232 = t9.*t206;
t241 = -t218;
t242 = -t229;
t244 = -t233;
t246 = t4.*t215;
t248 = t4.*t216;
t249 = -t236;
t250 = t8.*t216;
t253 = t8.*t219;
t254 = t4.*t221;
t256 = t8.*t221;
t257 = -t240;
t258 = -t239;
t265 = t5.*t231;
t266 = t8.*t229;
t267 = t9.*t228;
t268 = t8.*t230;
t269 = t9.*t231;
t270 = t5.*t234;
t271 = t9.*t233;
t272 = -t245;
t281 = -t251;
t285 = -t252;
t286 = -t255;
t287 = t21.*2.094139776807286e-7;
t288 = -t260;
t289 = -t262;
t290 = -t263;
t299 = -t275;
t302 = -t282;
t303 = -t283;
t304 = -t284;
t318 = t33+t39;
t327 = t16.*3.185951622063616e-7;
t337 = -t295;
t340 = -t298;
t344 = -t301;
t346 = -t305;
t347 = -t314;
t348 = -t315;
t353 = -t322;
t355 = -t323;
t356 = t15.*t239;
t357 = t5.*t20.*4.097607815548108e-7;
t358 = t18.*t240;
t359 = -t326;
t362 = -t330;
t364 = t8.*t296;
t365 = t5.*t273;
t366 = -t334;
t367 = -t335;
t368 = t5.*t275;
t369 = -t336;
t370 = t9.*t275;
t371 = -t339;
t373 = t4.*t8.*t19.*8.376559107229145e-7;
t374 = t5.*t9.*t18.*8.376559107229145e-7;
t375 = -t342;
t376 = -t343;
t377 = t8.*t309;
t379 = t8.*t310;
t380 = t8.*t319;
t382 = t8.*t320;
t383 = t8.*t322;
t384 = t4.*t325;
t386 = t8.*t324;
t387 = t4.*t328;
t388 = t8.*t325;
t389 = -t351;
t390 = t8.*t326;
t392 = t8.*t328;
t395 = t4.*t335;
t396 = t8.*t333;
t397 = t4.*t338;
t398 = -t363;
t401 = t8.*t338;
t405 = -t372;
t407 = t15.*t277;
t408 = t18.*t278;
t409 = t5.*t350;
t410 = t9.*t350;
t411 = t9.*t20.*2.227142959217101e-7;
t412 = -t381;
t413 = t9.*t352;
t415 = -t385;
t417 = -t391;
t418 = t8.*t360;
t419 = t4.*t363;
t420 = -t393;
t421 = t8.*t363;
t423 = t16.*t20.*2.094139776807286e-7;
t425 = -t394;
t427 = -t399;
t428 = t18.*t24.*6.371903244127231e-7;
t429 = t20.*t21.*3.185951622063616e-7;
t430 = t8.*t378;
t433 = t5.*t15.*(-1.11357147960855e-7);
t434 = t5.*t18.*(-2.227142959217101e-7);
t440 = t5.*t7.*t15.*6.892170885479394e-7;
t441 = t5.*t7.*t18.*6.892170885479394e-7;
t442 = t5.*t7.*t23.*6.892170885479394e-7;
t444 = t3.*t4.*t16.*7.044680628082447e-7;
t445 = t3.*t4.*t19.*7.044680628082447e-7;
t446 = t7.*t9.*t20.*3.446085442739697e-7;
t447 = t3.*t4.*t24.*7.044680628082447e-7;
t449 = t8.*t399;
t451 = t3.*t8.*t21.*3.522340314041224e-7;
t452 = t8.*t403;
t453 = t3.*t4.*t21.*1.07175327657342e-6;
t454 = t3.*t8.*t19.*1.07175327657342e-6;
t456 = t18.*t19.*6.371903244127231e-7;
t459 = -t431;
t478 = -t448;
t480 = t9.*t15.*1.608000198040319e-13;
t481 = t9.*t18.*1.608000198040319e-13;
t482 = t9.*t23.*1.608000198040319e-13;
t483 = t3.*t8.*t16.*5.358766382867102e-7;
t484 = t54+t55;
t485 = t15.*t16.*(-3.185951622063616e-7);
t488 = t7.*t15.*t16.*3.522340314041224e-7;
t489 = t7.*t18.*t19.*7.044680628082447e-7;
t491 = t7.*t19.*t23.*7.044680628082447e-7;
t492 = t7.*t9.*t15.*3.746051489620971e-7;
t493 = t5.*t7.*t20.*1.873025744810486e-7;
t494 = t7.*t9.*t18.*3.746051489620971e-7;
t495 = t7.*t20.*t21.*3.522340314041224e-7;
t496 = t7.*t9.*t23.*3.746051489620971e-7;
t498 = t43+t85;
t502 = -t462;
t503 = -t464;
t504 = -t465;
t505 = -t467;
t506 = -t468;
t507 = -t469;
t508 = t8.*t450;
t509 = -t474;
t510 = -t473;
t511 = -t476;
t512 = t4.*t7.*t8.*t19.*1.07175327657342e-6;
t513 = t9.*t18.*t325;
t514 = t5.*t20.*8.040000990201593e-14;
t515 = t4.*t7.*t8.*t24.*1.07175327657342e-6;
t516 = t9.*t23.*t325;
t521 = -t487;
t522 = -t490;
t530 = -t497;
t531 = t5.*t463;
t532 = t7.*t15.*t21.*5.358766382867102e-7;
t533 = t7.*t16.*t20.*5.358766382867102e-7;
t537 = -t499;
t538 = t9.*t463;
t539 = t5.*t466;
t542 = t8.*t472;
t543 = t9.*t471;
t544 = t8.*t474;
t545 = t20.*5.859823945197205e-8;
t546 = t9.*t476;
t548 = t5.*t7.*t9.*t23.*(-1.07175327657342e-6);
t549 = -t517;
t550 = t8.*t497;
t551 = t4.*t500;
t552 = t8.*t499;
t553 = t4.*t501;
t554 = t8.*t500;
t555 = t8.*t501;
t557 = -t534;
t561 = -t541;
t563 = t7.*t18.*2.536718707310641e-7;
t566 = t8.*t527;
t567 = t5.*t528;
t568 = t7.*t23.*2.536718707310641e-7;
t569 = t5.*t534;
t572 = t9.*t534;
t577 = t70+t86;
t578 = -t559;
t580 = t7.*t15.*9.856216067305823e-8;
t581 = t5.*t15.*2.10868590222219e-13;
t582 = t5.*t18.*2.10868590222219e-13;
t583 = t78+t89;
t584 = t5.*t23.*2.10868590222219e-13;
C_dq = ft_2({dq1,dq2,dq3,dq4,dq5,dq6,t100,t1001,t1002,t1005,t101,t102,t1023,t1024,t1026,t1027,t1037,t104,t1044,t1047,t105,t1050,t1059,t106,t1060,t1066,t1067,t1068,t1069,t107,t1070,t1071,t1078,t1079,t108,t1080,t1081,t109,t110,t1100,t1101,t1109,t111,t1110,t1111,t1112,t112,t113,t1139,t114,t1140,t1141,t1142,t1143,t115,t1154,t1155,t1158,t116,t1160,t1167,t1168,t1169,t117,t118,t119,t1196,t120,t1204,t1205,t121,t122,t1229,t123,t124,t1248,t125,t1250,t1258,t1259,t126,t1260,t1261,t1266,t1272,t1273,t128,t1282,t1284,t1285,t129,t1291,t130,t1302,t1303,t1304,t1305,t1307,t1308,t131,t1313,t1314,t132,t133,t1332,t1335,t1336,t134,t135,t136,t1360,t1361,t1362,t1363,t1367,t137,t1371,t1374,t1380,t1381,t1389,t139,t1390,t1393,t14,t140,t1400,t1409,t141,t1411,t1416,t142,t143,t1437,t144,t1449,t145,t1456,t1457,t146,t147,t1477,t148,t1485,t15,t150,t1504,t1505,t151,t152,t153,t1532,t1533,t1535,t154,t1547,t1549,t155,t1552,t1554,t1558,t1559,t1560,t1563,t157,t158,t159,t1596,t16,t160,t1604,t1606,t1608,t161,t1610,t1611,t1612,t1619,t162,t163,t1631,t1632,t1637,t1638,t1639,t164,t1644,t1645,t165,t1651,t1652,t1653,t1654,t1657,t1658,t1659,t166,t1660,t1661,t1662,t1664,t1666,t1668,t1676,t1677,t1678,t1679,t168,t1680,t1682,t1683,t1684,t1685,t1688,t1689,t169,t1692,t1693,t1694,t1695,t1696,t1698,t17,t170,t1702,t1703,t1709,t1712,t1713,t1714,t1716,t1717,t172,t1720,t1722,t1726,t1727,t1729,t173,t1734,t1736,t1737,t174,t1745,t1746,t1749,t175,t1750,t1751,t1752,t176,t177,t1785,t1786,t179,t1796,t1797,t1798,t1799,t18,t180,t1800,t1801,t1809,t181,t1810,t1816,t1819,t182,t1827,t1829,t183,t1833,t1838,t1840,t1841,t1842,t1849,t185,t1850,t1851,t1852,t1857,t1858,t1859,t186,t1871,t1873,t1876,t188,t1881,t1882,t1883,t1889,t1895,t1897,t1898,t19,t190,t1907,t191,t1911,t1912,t1913,t1914,t1915,t1916,t192,t1923,t1924,t1925,t1926,t1931,t1932,t1933,t1935,t1939,t1948,t1949,t1956,t1958,t1960,t1963,t1968,t1977,t1978,t1979,t1994,t1995,t1997,t2,t20,t2003,t2012,t2022,t2024,t2025,t2028,t2032,t2046,t2056,t2058,t206,t2063,t2064,t2065,t2067,t207,t2070,t2072,t2073,t2079,t2081,t2082,t2083,t2084,t2085,t2086,t2087,t2093,t2094,t2098,t21,t2100,t2103,t2104,t2105,t2106,t2110,t2113,t2115,t2117,t2131,t2132,t2144,t215,t2156,t216,t2171,t2172,t2173,t2175,t2176,t2179,t2180,t2182,t2183,t2188,t2189,t219,t2194,t22,t220,t2205,t2207,t221,t222,t2220,t2223,t2228,t223,t224,t225,t226,t2265,t227,t2277,t2279,t228,t2280,t2281,t2282,t2285,t2294,t23,t230,t2302,t2304,t2305,t2306,t231,t2321,t2322,t2323,t2324,t2325,t2329,t233,t2336,t2339,t234,t2340,t2344,t2348,t2349,t235,t2350,t2352,t2353,t2356,t236,t2360,t2361,t2362,t2363,t2364,t2365,t237,t2373,t2375,t2376,t2377,t2378,t2379,t238,t2380,t239,t24,t240,t2409,t241,t2412,t242,t2428,t2429,t243,t2430,t2432,t2433,t2435,t2436,t2438,t2439,t244,t2440,t2441,t2443,t245,t2456,t246,t247,t2470,t2474,t2475,t2476,t248,t2481,t2486,t2487,t2488,t2489,t249,t2491,t2493,t2495,t2496,t2497,t25,t2516,t252,t2521,t2527,t2528,t2529,t253,t2533,t254,t256,t257,t258,t259,t26,t260,t261,t263,t264,t266,t269,t27,t270,t272,t273,t274,t275,t276,t277,t278,t279,t28,t280,t281,t284,t285,t286,t287,t288,t2886,t289,t29,t290,t291,t292,t293,t294,t2953,t296,t297,t299,t3,t30,t300,t302,t303,t304,t305,t306,t307,t308,t309,t310,t311,t312,t313,t314,t315,t316,t317,t318,t319,t32,t320,t321,t322,t324,t325,t327,t328,t329,t33,t331,t332,t333,t334,t336,t337,t338,t34,t340,t341,t343,t344,t345,t346,t347,t348,t35,t350,t352,t353,t354,t355,t356,t357,t358,t359,t360,t362,t365,t366,t367,t368,t369,t37,t371,t372,t373,t374,t375,t376,t377,t378,t379,t38,t380,t382,t384,t386,t387,t388,t389,t391,t392,t395,t396,t398,t4,t40,t400,t401,t402,t403,t404,t406,t409,t41,t410,t411,t412,t413,t414,t415,t416,t417,t418,t419,t420,t421,t423,t424,t425,t426,t427,t428,t429,t431,t433,t434,t436,t437,t438,t439,t44,t440,t441,t442,t443,t444,t445,t446,t447,t448,t449,t45,t450,t451,t452,t453,t454,t456,t457,t458,t459,t46,t462,t463,t464,t465,t466,t468,t469,t47,t471,t472,t473,t474,t48,t480,t481,t482,t483,t484,t485,t488,t489,t49,t491,t492,t493,t494,t495,t496,t497,t498,t499,t5,t50,t500,t501,t502,t503,t504,t505,t506,t507,t508,t509,t51,t510,t511,t512,t513,t514,t515,t516,t517,t52,t521,t522,t526,t527,t528,t529,t53,t530,t531,t532,t533,t534,t535,t536,t537,t538,t539,t540,t543,t544,t545,t546,t548,t549,t551,t552,t553,t554,t555,t556,t557,t558,t559,t56,t560,t561,t562,t563,t564,t565,t567,t568,t569,t57,t570,t571,t572,t573,t574,t576,t577,t578,t58,t580,t581,t582,t583,t584,t59,t591,t593,t595,t596,t6,t60,t605,t61,t625,t63,t65,t655,t656,t659,t66,t660,t662,t663,t664,t666,t668,t67,t670,t671,t672,t673,t674,t675,t68,t682,t685,t686,t7,t71,t713,t717,t72,t724,t725,t727,t728,t73,t735,t736,t74,t746,t75,t752,t756,t759,t76,t761,t763,t764,t765,t766,t768,t769,t77,t770,t780,t785,t786,t787,t788,t789,t79,t791,t793,t795,t8,t80,t804,t81,t814,t82,t827,t828,t83,t84,t840,t849,t86,t87,t88,t882,t883,t884,t885,t886,t887,t888,t891,t892,t895,t896,t897,t898,t899,t9,t90,t900,t901,t904,t911,t918,t92,t93,t94,t942,t946,t95,t959,t96,t962,t964,t969,t97,t970,t971,t972,t977,t978,t979,t98,t980,t982,t986,t99,t997});
end
function C_dq = ft_2(ct)
dq1 = ct{1};
dq2 = ct{2};
dq3 = ct{3};
dq4 = ct{4};
dq5 = ct{5};
dq6 = ct{6};
t100 = ct{7};
t1001 = ct{8};
t1002 = ct{9};
t1005 = ct{10};
t101 = ct{11};
t102 = ct{12};
t1023 = ct{13};
t1024 = ct{14};
t1026 = ct{15};
t1027 = ct{16};
t1037 = ct{17};
t104 = ct{18};
t1044 = ct{19};
t1047 = ct{20};
t105 = ct{21};
t1050 = ct{22};
t1059 = ct{23};
t106 = ct{24};
t1060 = ct{25};
t1066 = ct{26};
t1067 = ct{27};
t1068 = ct{28};
t1069 = ct{29};
t107 = ct{30};
t1070 = ct{31};
t1071 = ct{32};
t1078 = ct{33};
t1079 = ct{34};
t108 = ct{35};
t1080 = ct{36};
t1081 = ct{37};
t109 = ct{38};
t110 = ct{39};
t1100 = ct{40};
t1101 = ct{41};
t1109 = ct{42};
t111 = ct{43};
t1110 = ct{44};
t1111 = ct{45};
t1112 = ct{46};
t112 = ct{47};
t113 = ct{48};
t1139 = ct{49};
t114 = ct{50};
t1140 = ct{51};
t1141 = ct{52};
t1142 = ct{53};
t1143 = ct{54};
t115 = ct{55};
t1154 = ct{56};
t1155 = ct{57};
t1158 = ct{58};
t116 = ct{59};
t1160 = ct{60};
t1167 = ct{61};
t1168 = ct{62};
t1169 = ct{63};
t117 = ct{64};
t118 = ct{65};
t119 = ct{66};
t1196 = ct{67};
t120 = ct{68};
t1204 = ct{69};
t1205 = ct{70};
t121 = ct{71};
t122 = ct{72};
t1229 = ct{73};
t123 = ct{74};
t124 = ct{75};
t1248 = ct{76};
t125 = ct{77};
t1250 = ct{78};
t1258 = ct{79};
t1259 = ct{80};
t126 = ct{81};
t1260 = ct{82};
t1261 = ct{83};
t1266 = ct{84};
t1272 = ct{85};
t1273 = ct{86};
t128 = ct{87};
t1282 = ct{88};
t1284 = ct{89};
t1285 = ct{90};
t129 = ct{91};
t1291 = ct{92};
t130 = ct{93};
t1302 = ct{94};
t1303 = ct{95};
t1304 = ct{96};
t1305 = ct{97};
t1307 = ct{98};
t1308 = ct{99};
t131 = ct{100};
t1313 = ct{101};
t1314 = ct{102};
t132 = ct{103};
t133 = ct{104};
t1332 = ct{105};
t1335 = ct{106};
t1336 = ct{107};
t134 = ct{108};
t135 = ct{109};
t136 = ct{110};
t1360 = ct{111};
t1361 = ct{112};
t1362 = ct{113};
t1363 = ct{114};
t1367 = ct{115};
t137 = ct{116};
t1371 = ct{117};
t1374 = ct{118};
t1380 = ct{119};
t1381 = ct{120};
t1389 = ct{121};
t139 = ct{122};
t1390 = ct{123};
t1393 = ct{124};
t14 = ct{125};
t140 = ct{126};
t1400 = ct{127};
t1409 = ct{128};
t141 = ct{129};
t1411 = ct{130};
t1416 = ct{131};
t142 = ct{132};
t143 = ct{133};
t1437 = ct{134};
t144 = ct{135};
t1449 = ct{136};
t145 = ct{137};
t1456 = ct{138};
t1457 = ct{139};
t146 = ct{140};
t147 = ct{141};
t1477 = ct{142};
t148 = ct{143};
t1485 = ct{144};
t15 = ct{145};
t150 = ct{146};
t1504 = ct{147};
t1505 = ct{148};
t151 = ct{149};
t152 = ct{150};
t153 = ct{151};
t1532 = ct{152};
t1533 = ct{153};
t1535 = ct{154};
t154 = ct{155};
t1547 = ct{156};
t1549 = ct{157};
t155 = ct{158};
t1552 = ct{159};
t1554 = ct{160};
t1558 = ct{161};
t1559 = ct{162};
t1560 = ct{163};
t1563 = ct{164};
t157 = ct{165};
t158 = ct{166};
t159 = ct{167};
t1596 = ct{168};
t16 = ct{169};
t160 = ct{170};
t1604 = ct{171};
t1606 = ct{172};
t1608 = ct{173};
t161 = ct{174};
t1610 = ct{175};
t1611 = ct{176};
t1612 = ct{177};
t1619 = ct{178};
t162 = ct{179};
t163 = ct{180};
t1631 = ct{181};
t1632 = ct{182};
t1637 = ct{183};
t1638 = ct{184};
t1639 = ct{185};
t164 = ct{186};
t1644 = ct{187};
t1645 = ct{188};
t165 = ct{189};
t1651 = ct{190};
t1652 = ct{191};
t1653 = ct{192};
t1654 = ct{193};
t1657 = ct{194};
t1658 = ct{195};
t1659 = ct{196};
t166 = ct{197};
t1660 = ct{198};
t1661 = ct{199};
t1662 = ct{200};
t1664 = ct{201};
t1666 = ct{202};
t1668 = ct{203};
t1676 = ct{204};
t1677 = ct{205};
t1678 = ct{206};
t1679 = ct{207};
t168 = ct{208};
t1680 = ct{209};
t1682 = ct{210};
t1683 = ct{211};
t1684 = ct{212};
t1685 = ct{213};
t1688 = ct{214};
t1689 = ct{215};
t169 = ct{216};
t1692 = ct{217};
t1693 = ct{218};
t1694 = ct{219};
t1695 = ct{220};
t1696 = ct{221};
t1698 = ct{222};
t17 = ct{223};
t170 = ct{224};
t1702 = ct{225};
t1703 = ct{226};
t1709 = ct{227};
t1712 = ct{228};
t1713 = ct{229};
t1714 = ct{230};
t1716 = ct{231};
t1717 = ct{232};
t172 = ct{233};
t1720 = ct{234};
t1722 = ct{235};
t1726 = ct{236};
t1727 = ct{237};
t1729 = ct{238};
t173 = ct{239};
t1734 = ct{240};
t1736 = ct{241};
t1737 = ct{242};
t174 = ct{243};
t1745 = ct{244};
t1746 = ct{245};
t1749 = ct{246};
t175 = ct{247};
t1750 = ct{248};
t1751 = ct{249};
t1752 = ct{250};
t176 = ct{251};
t177 = ct{252};
t1785 = ct{253};
t1786 = ct{254};
t179 = ct{255};
t1796 = ct{256};
t1797 = ct{257};
t1798 = ct{258};
t1799 = ct{259};
t18 = ct{260};
t180 = ct{261};
t1800 = ct{262};
t1801 = ct{263};
t1809 = ct{264};
t181 = ct{265};
t1810 = ct{266};
t1816 = ct{267};
t1819 = ct{268};
t182 = ct{269};
t1827 = ct{270};
t1829 = ct{271};
t183 = ct{272};
t1833 = ct{273};
t1838 = ct{274};
t1840 = ct{275};
t1841 = ct{276};
t1842 = ct{277};
t1849 = ct{278};
t185 = ct{279};
t1850 = ct{280};
t1851 = ct{281};
t1852 = ct{282};
t1857 = ct{283};
t1858 = ct{284};
t1859 = ct{285};
t186 = ct{286};
t1871 = ct{287};
t1873 = ct{288};
t1876 = ct{289};
t188 = ct{290};
t1881 = ct{291};
t1882 = ct{292};
t1883 = ct{293};
t1889 = ct{294};
t1895 = ct{295};
t1897 = ct{296};
t1898 = ct{297};
t19 = ct{298};
t190 = ct{299};
t1907 = ct{300};
t191 = ct{301};
t1911 = ct{302};
t1912 = ct{303};
t1913 = ct{304};
t1914 = ct{305};
t1915 = ct{306};
t1916 = ct{307};
t192 = ct{308};
t1923 = ct{309};
t1924 = ct{310};
t1925 = ct{311};
t1926 = ct{312};
t1931 = ct{313};
t1932 = ct{314};
t1933 = ct{315};
t1935 = ct{316};
t1939 = ct{317};
t1948 = ct{318};
t1949 = ct{319};
t1956 = ct{320};
t1958 = ct{321};
t1960 = ct{322};
t1963 = ct{323};
t1968 = ct{324};
t1977 = ct{325};
t1978 = ct{326};
t1979 = ct{327};
t1994 = ct{328};
t1995 = ct{329};
t1997 = ct{330};
t2 = ct{331};
t20 = ct{332};
t2003 = ct{333};
t2012 = ct{334};
t2022 = ct{335};
t2024 = ct{336};
t2025 = ct{337};
t2028 = ct{338};
t2032 = ct{339};
t2046 = ct{340};
t2056 = ct{341};
t2058 = ct{342};
t206 = ct{343};
t2063 = ct{344};
t2064 = ct{345};
t2065 = ct{346};
t2067 = ct{347};
t207 = ct{348};
t2070 = ct{349};
t2072 = ct{350};
t2073 = ct{351};
t2079 = ct{352};
t2081 = ct{353};
t2082 = ct{354};
t2083 = ct{355};
t2084 = ct{356};
t2085 = ct{357};
t2086 = ct{358};
t2087 = ct{359};
t2093 = ct{360};
t2094 = ct{361};
t2098 = ct{362};
t21 = ct{363};
t2100 = ct{364};
t2103 = ct{365};
t2104 = ct{366};
t2105 = ct{367};
t2106 = ct{368};
t2110 = ct{369};
t2113 = ct{370};
t2115 = ct{371};
t2117 = ct{372};
t2131 = ct{373};
t2132 = ct{374};
t2144 = ct{375};
t215 = ct{376};
t2156 = ct{377};
t216 = ct{378};
t2171 = ct{379};
t2172 = ct{380};
t2173 = ct{381};
t2175 = ct{382};
t2176 = ct{383};
t2179 = ct{384};
t2180 = ct{385};
t2182 = ct{386};
t2183 = ct{387};
t2188 = ct{388};
t2189 = ct{389};
t219 = ct{390};
t2194 = ct{391};
t22 = ct{392};
t220 = ct{393};
t2205 = ct{394};
t2207 = ct{395};
t221 = ct{396};
t222 = ct{397};
t2220 = ct{398};
t2223 = ct{399};
t2228 = ct{400};
t223 = ct{401};
t224 = ct{402};
t225 = ct{403};
t226 = ct{404};
t2265 = ct{405};
t227 = ct{406};
t2277 = ct{407};
t2279 = ct{408};
t228 = ct{409};
t2280 = ct{410};
t2281 = ct{411};
t2282 = ct{412};
t2285 = ct{413};
t2294 = ct{414};
t23 = ct{415};
t230 = ct{416};
t2302 = ct{417};
t2304 = ct{418};
t2305 = ct{419};
t2306 = ct{420};
t231 = ct{421};
t2321 = ct{422};
t2322 = ct{423};
t2323 = ct{424};
t2324 = ct{425};
t2325 = ct{426};
t2329 = ct{427};
t233 = ct{428};
t2336 = ct{429};
t2339 = ct{430};
t234 = ct{431};
t2340 = ct{432};
t2344 = ct{433};
t2348 = ct{434};
t2349 = ct{435};
t235 = ct{436};
t2350 = ct{437};
t2352 = ct{438};
t2353 = ct{439};
t2356 = ct{440};
t236 = ct{441};
t2360 = ct{442};
t2361 = ct{443};
t2362 = ct{444};
t2363 = ct{445};
t2364 = ct{446};
t2365 = ct{447};
t237 = ct{448};
t2373 = ct{449};
t2375 = ct{450};
t2376 = ct{451};
t2377 = ct{452};
t2378 = ct{453};
t2379 = ct{454};
t238 = ct{455};
t2380 = ct{456};
t239 = ct{457};
t24 = ct{458};
t240 = ct{459};
t2409 = ct{460};
t241 = ct{461};
t2412 = ct{462};
t242 = ct{463};
t2428 = ct{464};
t2429 = ct{465};
t243 = ct{466};
t2430 = ct{467};
t2432 = ct{468};
t2433 = ct{469};
t2435 = ct{470};
t2436 = ct{471};
t2438 = ct{472};
t2439 = ct{473};
t244 = ct{474};
t2440 = ct{475};
t2441 = ct{476};
t2443 = ct{477};
t245 = ct{478};
t2456 = ct{479};
t246 = ct{480};
t247 = ct{481};
t2470 = ct{482};
t2474 = ct{483};
t2475 = ct{484};
t2476 = ct{485};
t248 = ct{486};
t2481 = ct{487};
t2486 = ct{488};
t2487 = ct{489};
t2488 = ct{490};
t2489 = ct{491};
t249 = ct{492};
t2491 = ct{493};
t2493 = ct{494};
t2495 = ct{495};
t2496 = ct{496};
t2497 = ct{497};
t25 = ct{498};
t2516 = ct{499};
t252 = ct{500};
t2521 = ct{501};
t2527 = ct{502};
t2528 = ct{503};
t2529 = ct{504};
t253 = ct{505};
t2533 = ct{506};
t254 = ct{507};
t256 = ct{508};
t257 = ct{509};
t258 = ct{510};
t259 = ct{511};
t26 = ct{512};
t260 = ct{513};
t261 = ct{514};
t263 = ct{515};
t264 = ct{516};
t266 = ct{517};
t269 = ct{518};
t27 = ct{519};
t270 = ct{520};
t272 = ct{521};
t273 = ct{522};
t274 = ct{523};
t275 = ct{524};
t276 = ct{525};
t277 = ct{526};
t278 = ct{527};
t279 = ct{528};
t28 = ct{529};
t280 = ct{530};
t281 = ct{531};
t284 = ct{532};
t285 = ct{533};
t286 = ct{534};
t287 = ct{535};
t288 = ct{536};
t2886 = ct{537};
t289 = ct{538};
t29 = ct{539};
t290 = ct{540};
t291 = ct{541};
t292 = ct{542};
t293 = ct{543};
t294 = ct{544};
t2953 = ct{545};
t296 = ct{546};
t297 = ct{547};
t299 = ct{548};
t3 = ct{549};
t30 = ct{550};
t300 = ct{551};
t302 = ct{552};
t303 = ct{553};
t304 = ct{554};
t305 = ct{555};
t306 = ct{556};
t307 = ct{557};
t308 = ct{558};
t309 = ct{559};
t310 = ct{560};
t311 = ct{561};
t312 = ct{562};
t313 = ct{563};
t314 = ct{564};
t315 = ct{565};
t316 = ct{566};
t317 = ct{567};
t318 = ct{568};
t319 = ct{569};
t32 = ct{570};
t320 = ct{571};
t321 = ct{572};
t322 = ct{573};
t324 = ct{574};
t325 = ct{575};
t327 = ct{576};
t328 = ct{577};
t329 = ct{578};
t33 = ct{579};
t331 = ct{580};
t332 = ct{581};
t333 = ct{582};
t334 = ct{583};
t336 = ct{584};
t337 = ct{585};
t338 = ct{586};
t34 = ct{587};
t340 = ct{588};
t341 = ct{589};
t343 = ct{590};
t344 = ct{591};
t345 = ct{592};
t346 = ct{593};
t347 = ct{594};
t348 = ct{595};
t35 = ct{596};
t350 = ct{597};
t352 = ct{598};
t353 = ct{599};
t354 = ct{600};
t355 = ct{601};
t356 = ct{602};
t357 = ct{603};
t358 = ct{604};
t359 = ct{605};
t360 = ct{606};
t362 = ct{607};
t365 = ct{608};
t366 = ct{609};
t367 = ct{610};
t368 = ct{611};
t369 = ct{612};
t37 = ct{613};
t371 = ct{614};
t372 = ct{615};
t373 = ct{616};
t374 = ct{617};
t375 = ct{618};
t376 = ct{619};
t377 = ct{620};
t378 = ct{621};
t379 = ct{622};
t38 = ct{623};
t380 = ct{624};
t382 = ct{625};
t384 = ct{626};
t386 = ct{627};
t387 = ct{628};
t388 = ct{629};
t389 = ct{630};
t391 = ct{631};
t392 = ct{632};
t395 = ct{633};
t396 = ct{634};
t398 = ct{635};
t4 = ct{636};
t40 = ct{637};
t400 = ct{638};
t401 = ct{639};
t402 = ct{640};
t403 = ct{641};
t404 = ct{642};
t406 = ct{643};
t409 = ct{644};
t41 = ct{645};
t410 = ct{646};
t411 = ct{647};
t412 = ct{648};
t413 = ct{649};
t414 = ct{650};
t415 = ct{651};
t416 = ct{652};
t417 = ct{653};
t418 = ct{654};
t419 = ct{655};
t420 = ct{656};
t421 = ct{657};
t423 = ct{658};
t424 = ct{659};
t425 = ct{660};
t426 = ct{661};
t427 = ct{662};
t428 = ct{663};
t429 = ct{664};
t431 = ct{665};
t433 = ct{666};
t434 = ct{667};
t436 = ct{668};
t437 = ct{669};
t438 = ct{670};
t439 = ct{671};
t44 = ct{672};
t440 = ct{673};
t441 = ct{674};
t442 = ct{675};
t443 = ct{676};
t444 = ct{677};
t445 = ct{678};
t446 = ct{679};
t447 = ct{680};
t448 = ct{681};
t449 = ct{682};
t45 = ct{683};
t450 = ct{684};
t451 = ct{685};
t452 = ct{686};
t453 = ct{687};
t454 = ct{688};
t456 = ct{689};
t457 = ct{690};
t458 = ct{691};
t459 = ct{692};
t46 = ct{693};
t462 = ct{694};
t463 = ct{695};
t464 = ct{696};
t465 = ct{697};
t466 = ct{698};
t468 = ct{699};
t469 = ct{700};
t47 = ct{701};
t471 = ct{702};
t472 = ct{703};
t473 = ct{704};
t474 = ct{705};
t48 = ct{706};
t480 = ct{707};
t481 = ct{708};
t482 = ct{709};
t483 = ct{710};
t484 = ct{711};
t485 = ct{712};
t488 = ct{713};
t489 = ct{714};
t49 = ct{715};
t491 = ct{716};
t492 = ct{717};
t493 = ct{718};
t494 = ct{719};
t495 = ct{720};
t496 = ct{721};
t497 = ct{722};
t498 = ct{723};
t499 = ct{724};
t5 = ct{725};
t50 = ct{726};
t500 = ct{727};
t501 = ct{728};
t502 = ct{729};
t503 = ct{730};
t504 = ct{731};
t505 = ct{732};
t506 = ct{733};
t507 = ct{734};
t508 = ct{735};
t509 = ct{736};
t51 = ct{737};
t510 = ct{738};
t511 = ct{739};
t512 = ct{740};
t513 = ct{741};
t514 = ct{742};
t515 = ct{743};
t516 = ct{744};
t517 = ct{745};
t52 = ct{746};
t521 = ct{747};
t522 = ct{748};
t526 = ct{749};
t527 = ct{750};
t528 = ct{751};
t529 = ct{752};
t53 = ct{753};
t530 = ct{754};
t531 = ct{755};
t532 = ct{756};
t533 = ct{757};
t534 = ct{758};
t535 = ct{759};
t536 = ct{760};
t537 = ct{761};
t538 = ct{762};
t539 = ct{763};
t540 = ct{764};
t543 = ct{765};
t544 = ct{766};
t545 = ct{767};
t546 = ct{768};
t548 = ct{769};
t549 = ct{770};
t551 = ct{771};
t552 = ct{772};
t553 = ct{773};
t554 = ct{774};
t555 = ct{775};
t556 = ct{776};
t557 = ct{777};
t558 = ct{778};
t559 = ct{779};
t56 = ct{780};
t560 = ct{781};
t561 = ct{782};
t562 = ct{783};
t563 = ct{784};
t564 = ct{785};
t565 = ct{786};
t567 = ct{787};
t568 = ct{788};
t569 = ct{789};
t57 = ct{790};
t570 = ct{791};
t571 = ct{792};
t572 = ct{793};
t573 = ct{794};
t574 = ct{795};
t576 = ct{796};
t577 = ct{797};
t578 = ct{798};
t58 = ct{799};
t580 = ct{800};
t581 = ct{801};
t582 = ct{802};
t583 = ct{803};
t584 = ct{804};
t59 = ct{805};
t591 = ct{806};
t593 = ct{807};
t595 = ct{808};
t596 = ct{809};
t6 = ct{810};
t60 = ct{811};
t605 = ct{812};
t61 = ct{813};
t625 = ct{814};
t63 = ct{815};
t65 = ct{816};
t655 = ct{817};
t656 = ct{818};
t659 = ct{819};
t66 = ct{820};
t660 = ct{821};
t662 = ct{822};
t663 = ct{823};
t664 = ct{824};
t666 = ct{825};
t668 = ct{826};
t67 = ct{827};
t670 = ct{828};
t671 = ct{829};
t672 = ct{830};
t673 = ct{831};
t674 = ct{832};
t675 = ct{833};
t68 = ct{834};
t682 = ct{835};
t685 = ct{836};
t686 = ct{837};
t7 = ct{838};
t71 = ct{839};
t713 = ct{840};
t717 = ct{841};
t72 = ct{842};
t724 = ct{843};
t725 = ct{844};
t727 = ct{845};
t728 = ct{846};
t73 = ct{847};
t735 = ct{848};
t736 = ct{849};
t74 = ct{850};
t746 = ct{851};
t75 = ct{852};
t752 = ct{853};
t756 = ct{854};
t759 = ct{855};
t76 = ct{856};
t761 = ct{857};
t763 = ct{858};
t764 = ct{859};
t765 = ct{860};
t766 = ct{861};
t768 = ct{862};
t769 = ct{863};
t77 = ct{864};
t770 = ct{865};
t780 = ct{866};
t785 = ct{867};
t786 = ct{868};
t787 = ct{869};
t788 = ct{870};
t789 = ct{871};
t79 = ct{872};
t791 = ct{873};
t793 = ct{874};
t795 = ct{875};
t8 = ct{876};
t80 = ct{877};
t804 = ct{878};
t81 = ct{879};
t814 = ct{880};
t82 = ct{881};
t827 = ct{882};
t828 = ct{883};
t83 = ct{884};
t84 = ct{885};
t840 = ct{886};
t849 = ct{887};
t86 = ct{888};
t87 = ct{889};
t88 = ct{890};
t882 = ct{891};
t883 = ct{892};
t884 = ct{893};
t885 = ct{894};
t886 = ct{895};
t887 = ct{896};
t888 = ct{897};
t891 = ct{898};
t892 = ct{899};
t895 = ct{900};
t896 = ct{901};
t897 = ct{902};
t898 = ct{903};
t899 = ct{904};
t9 = ct{905};
t90 = ct{906};
t900 = ct{907};
t901 = ct{908};
t904 = ct{909};
t911 = ct{910};
t918 = ct{911};
t92 = ct{912};
t93 = ct{913};
t94 = ct{914};
t942 = ct{915};
t946 = ct{916};
t95 = ct{917};
t959 = ct{918};
t96 = ct{919};
t962 = ct{920};
t964 = ct{921};
t969 = ct{922};
t97 = ct{923};
t970 = ct{924};
t971 = ct{925};
t972 = ct{926};
t977 = ct{927};
t978 = ct{928};
t979 = ct{929};
t98 = ct{930};
t980 = ct{931};
t982 = ct{932};
t986 = ct{933};
t99 = ct{934};
t997 = ct{935};
t585 = t9.*t20.*1.054342951111095e-13;
t586 = t15.*t473;
t587 = t18.*t474;
t588 = t7.*t9.*t20.*2.7046541903611e-13;
t590 = -t564;
t592 = -t565;
t606 = t15.*t535;
t607 = t5.*t7.*t20.*3.546806877605634e-13;
t608 = t18.*t536;
t609 = -t605;
t610 = t7.*t9.*t15.*(-1.773403438802817e-13);
t612 = t7.*t9.*t18.*(-3.546806877605634e-13);
t613 = t114+t126;
t614 = t15.*3.726186322907759e-7;
t623 = t7.*t20.*6.267440429796511e-7;
t626 = t107+t159;
t629 = t109+t160;
t638 = t142+t151;
t676 = -t659;
t683 = -t666;
t687 = -t670;
t688 = -t671;
t689 = t4.*t655;
t690 = t5.*t655;
t693 = t8.*t655;
t694 = t4.*t656;
t695 = t9.*t655;
t696 = t5.*t656;
t697 = t8.*t656;
t698 = t9.*t656;
t699 = t5.*t659;
t700 = -t672;
t701 = t9.*t659;
t702 = t5.*t660;
t703 = t9.*t660;
t704 = t9.*t662;
t705 = t5.*t664;
t706 = t9.*t664;
t707 = t5.*t666;
t709 = t9.*t666;
t711 = t5.*t668;
t714 = t4.*t670;
t715 = t9.*t668;
t716 = t5.*t670;
t718 = t8.*t670;
t719 = t4.*t671;
t720 = t9.*t670;
t721 = t5.*t671;
t722 = t8.*t671;
t723 = t9.*t671;
t726 = t5.*t672;
t730 = t9.*t672;
t731 = t5.*t673;
t732 = t5.*t674;
t733 = t9.*t673;
t734 = t9.*t674;
t737 = t5.*t662;
t744 = t4.*t682;
t745 = t5.*t682;
t747 = t8.*t682;
t748 = t4.*t685;
t749 = t9.*t682;
t750 = t5.*t685;
t751 = t5.*t686;
t755 = t8.*t685;
t757 = t9.*t685;
t758 = t9.*t686;
t762 = -t717;
t805 = t5.*t717;
t808 = t16.*3.256264776948168e-7;
t809 = t9.*t717;
t815 = -t761;
t816 = t4.*t725;
t818 = t8.*t725;
t819 = t4.*t727;
t820 = -t770;
t821 = t8.*t727;
t822 = t8.*t728;
t825 = -t789;
t837 = t5.*t761;
t838 = t5.*t764;
t839 = t9.*t761;
t841 = t9.*t763;
t842 = t9.*t764;
t843 = t8.*t766;
t846 = t9.*t768;
t851 = t4.*t787;
t854 = t8.*t787;
t855 = t4.*t788;
t857 = t4.*t791;
t862 = t8.*t791;
t864 = t8.*t793;
t873 = -t827;
t874 = -t828;
t903 = t16.*9.212362233958261e-7;
t906 = t9.*t17.*2.094020497221851e-7;
t921 = t8.*t804;
t922 = -t883;
t923 = -t882;
t924 = t14.*4.420145378913349e-10;
t926 = -t886;
t927 = -t887;
t934 = -t896;
t935 = -t895;
t936 = -t898;
t937 = -t897;
t939 = -t899;
t940 = -t901;
t941 = -t900;
t949 = t3.*t7.*t19.*8.561427670149984e-7;
t950 = t5.*t9.*t17.*8.561427670149984e-7;
t956 = t9.*t18.*3.830213761093238e-7;
t957 = t9.*t18.*3.830213761093238e-7;
t958 = -t918;
t960 = t5.*t17.*1.138147723446811e-7;
t961 = t18.*t19.*5.956097457010092e-7;
t966 = t18.*t24.*5.956097457010092e-7;
t967 = t3.*t7.*t19.*2.422130211756745e-6;
t968 = t5.*t9.*t17.*2.422130211756745e-6;
t981 = t17.*t19.*6.512529553896337e-7;
t983 = t17.*t24.*6.512529553896337e-7;
t984 = t9.*t17.*5.924234258315089e-7;
t988 = t5.*t7.*t18.*7.044279371874937e-7;
t989 = t5.*t7.*t18.*7.044279371874937e-7;
t992 = t8.*t9.*t22.*2.094020497221851e-7;
t993 = t3.*t8.*t19.*1.095406603137407e-6;
t994 = t4.*t7.*t19.*1.095406603137407e-6;
t995 = t5.*t7.*t23.*7.044279371874937e-7;
t996 = t5.*t7.*t23.*7.044279371874937e-7;
t999 = t3.*t4.*t19.*7.200154966325453e-7;
t1000 = t3.*t4.*t19.*7.200154966325453e-7;
t1003 = t3.*t4.*t24.*7.200154966325453e-7;
t1004 = t3.*t4.*t24.*7.200154966325453e-7;
t1006 = t4.*t17.*4.593136418534343e-9;
t1007 = t4.*t22.*4.593136418534343e-9;
t1012 = -t959;
t1013 = t4.*t8.*t19.*7.829937223708732e-7;
t1014 = t4.*t8.*t19.*7.829937223708732e-7;
t1015 = t5.*t9.*t18.*7.829937223708732e-7;
t1016 = t5.*t9.*t18.*7.829937223708732e-7;
t1028 = t5.*t18.*2.081808214526309e-7;
t1029 = t5.*t18.*2.081808214526309e-7;
t1030 = -t962;
t1034 = -t969;
t1035 = -t972;
t1038 = t8.*t942;
t1039 = -t978;
t1040 = -t977;
t1041 = -t980;
t1042 = -t979;
t1045 = -t982;
t1048 = t3.*t7.*t8.*t19.*4.280713835074992e-7;
t1049 = t8.*t17.*t770;
t1052 = t3.*t7.*t8.*t24.*4.280713835074992e-7;
t1053 = t8.*t22.*t770;
t1058 = -t997;
t1062 = -t1001;
t1063 = -t1002;
t1064 = t14.*1.250511956078399e-9;
t1086 = t4.*t17.*1.299453188729364e-8;
t1091 = t5.*t8.*t22.*1.138147723446811e-7;
t1092 = t3.*t4.*t7.*t770;
t1093 = -t1023;
t1094 = t4.*t22.*1.299453188729364e-8;
t1096 = t3.*t7.*t8.*t24.*1.211065105878372e-6;
t1097 = t8.*t22.*t828;
t1098 = t7.*t18.*t19.*7.200154966325453e-7;
t1099 = t7.*t18.*t19.*7.200154966325453e-7;
t1102 = t7.*t19.*t23.*7.200154966325453e-7;
t1103 = t7.*t19.*t23.*7.200154966325453e-7;
t1105 = t7.*t9.*t18.*3.828725908394669e-7;
t1106 = t7.*t9.*t18.*3.828725908394669e-7;
t1108 = -t1037;
t1113 = t8.*t19.*t22.*6.512529553896337e-7;
t1114 = t18.*t884;
t1115 = t4.*t5.*t8.*t17.*4.188040994443703e-7;
t1116 = t7.*t9.*t23.*3.828725908394669e-7;
t1117 = t7.*t9.*t23.*3.828725908394669e-7;
t1118 = t5.*t17.*3.219955937973119e-7;
t1119 = -t1044;
t1123 = t8.*t9.*t22.*5.924234258315089e-7;
t1124 = t3.*t4.*t7.*t828;
t1126 = t5.*t7.*t9.*t18.*1.095406603137407e-6;
t1128 = t5.*t8.*t9.*t22.*(-4.280713835074992e-7);
t1129 = t4.*t7.*t8.*t24.*1.095406603137407e-6;
t1130 = t5.*t7.*t9.*t23.*1.095406603137407e-6;
t1133 = -t1060;
t1134 = -t1059;
t1137 = t17.*t19.*1.842472446791652e-6;
t1138 = t3.*t4.*t7.*t19.*6.512529553896337e-7;
t1144 = t17.*t24.*1.842472446791652e-6;
t1150 = t3.*t8.*t19.*1.095406603137407e-6;
t1151 = t4.*t7.*t19.*1.095406603137407e-6;
t1152 = -t1067;
t1153 = -t1068;
t1159 = t5.*t8.*t17.*(-1.138147723446811e-7);
t1161 = -t1079;
t1162 = -t1078;
t1163 = -t1080;
t1164 = t18.*t19.*5.956097457010092e-7;
t1170 = t18.*t24.*5.956097457010092e-7;
t1171 = t3.*t7.*t8.*t19.*1.211065105878372e-6;
t1172 = t8.*t17.*t828;
t1176 = t18.*t959;
t1177 = t4.*t5.*t8.*t17.*1.184846851663018e-6;
t1178 = -t1100;
t1182 = t8.*t17.*t19.*(-6.512529553896337e-7);
t1185 = -t1110;
t1186 = -t1109;
t1187 = -t1112;
t1188 = -t1111;
t1189 = t3.*t5.*t7.*t18.*(-4.188040994443703e-7);
t1195 = t8.*t9.*t17.*(-5.924234258315089e-7);
t1207 = -t1142;
t1208 = -t1143;
t1209 = t18.*t946;
t1210 = t4.*t8.*t9.*t17.*2.276295446893622e-7;
t1214 = t8.*t1078;
t1215 = t8.*t1079;
t1216 = t8.*t1080;
t1217 = t8.*t1081;
t1218 = t3.*t7.*t18.*t19.*4.280713835074992e-7;
t1219 = t4.*t8.*t17.*t19.*4.280713835074992e-7;
t1220 = t17.*t18.*t770;
t1221 = -t1154;
t1222 = t9.*t17.*t18.*(-2.094020497221851e-7);
t1223 = -t1160;
t1225 = -t1168;
t1226 = t5.*t8.*t9.*t17.*(-1.211065105878372e-6);
t1231 = t5.*t8.*t22.*3.219955937973119e-7;
t1232 = t3.*t7.*t18.*t19.*1.211065105878372e-6;
t1233 = t4.*t8.*t17.*t19.*1.211065105878372e-6;
t1234 = t17.*t18.*t828;
t1236 = t8.*t17.*3.249671339417237e-7;
t1238 = t8.*t22.*3.249671339417237e-7;
t1240 = t17.*t18.*t19.*3.256264776948168e-7;
t1243 = t3.*t5.*t7.*t9.*t18.*6.512529553896337e-7;
t1244 = t4.*t5.*t8.*t9.*t17.*6.512529553896337e-7;
t1245 = t8.*t1143;
t1246 = t17.*t18.*t24.*3.256264776948168e-7;
t1247 = t8.*t19.*t22.*1.842472446791652e-6;
t1251 = -t1204;
t1253 = t5.*t7.*t9.*t18.*1.095406603137407e-6;
t1254 = t4.*t7.*t8.*t24.*1.095406603137407e-6;
t1255 = t5.*t7.*t9.*t23.*1.095406603137407e-6;
t1256 = t3.*t7.*t9.*t18.*(-2.276295446893622e-7);
t1264 = t5.*t9.*t17.*t18.*(-4.280713835074992e-7);
t1274 = t3.*t4.*t7.*t19.*1.842472446791652e-6;
t1275 = t8.*t17.*9.193708611153409e-7;
t1276 = t8.*t22.*9.193708611153409e-7;
t1278 = t3.*t9.*t18.*2.764345231392299e-13;
t1279 = t3.*t9.*t18.*2.764345231392299e-13;
t1280 = t5.*t7.*t18.*2.764345231392299e-13;
t1281 = t5.*t7.*t18.*2.764345231392299e-13;
t1283 = t4.*t5.*t17.*8.217441799717035e-14;
t1286 = t4.*t5.*t22.*8.217441799717035e-14;
t1288 = t5.*t9.*t17.*t18.*(-1.211065105878372e-6);
t1298 = -t1248;
t1300 = t9.*t17.*t18.*(-5.924234258315089e-7);
t1301 = t4.*t7.*t8.*t19.*(-1.095406603137407e-6);
t1309 = t9.*t18.*1.503068317813338e-13;
t1310 = t9.*t18.*1.503068317813338e-13;
t1312 = -t1266;
t1315 = t9.*t23.*1.503068317813338e-13;
t1316 = t9.*t23.*1.503068317813338e-13;
t1319 = -t1272;
t1321 = t18.*t1160;
t1322 = t4.*t8.*t9.*t17.*6.439911875946239e-7;
t1324 = -t1282;
t1326 = t7.*t18.*2.592703454263624e-7;
t1327 = t7.*t18.*2.592703454263624e-7;
t1328 = -t1284;
t1329 = t7.*t23.*2.592703454263624e-7;
t1330 = t7.*t23.*2.592703454263624e-7;
t1331 = -t1291;
t1337 = -t1303;
t1338 = -t1302;
t1339 = -t1305;
t1340 = -t1304;
t1341 = -t1308;
t1344 = t17.*t18.*t19.*9.212362233958261e-7;
t1345 = -t1314;
t1347 = t3.*t5.*t7.*t9.*t18.*1.842472446791652e-6;
t1348 = t4.*t5.*t8.*t9.*t17.*1.842472446791652e-6;
t1349 = t17.*t18.*t24.*9.212362233958261e-7;
t1351 = t3.*t7.*t18.*1.54144203823673e-7;
t1352 = t4.*t8.*t17.*1.54144203823673e-7;
t1356 = t4.*t9.*t17.*1.077612036149773e-13;
t1357 = t4.*t9.*t22.*1.077612036149773e-13;
t1358 = t4.*t5.*t17.*2.324812497785041e-13;
t1359 = t4.*t5.*t22.*2.324812497785041e-13;
t1364 = t8.*t1304;
t1365 = t8.*t1305;
t1366 = t9.*t17.*t18.*8.217441799717035e-14;
t1368 = -t1336;
t1369 = -t1335;
t1370 = t9.*t17.*t23.*8.217441799717035e-14;
t1372 = t8.*t1313;
t1373 = t8.*t1314;
t1375 = t5.*t18.*1.97108120739817e-13;
t1376 = t5.*t18.*1.97108120739817e-13;
t1378 = t5.*t23.*1.97108120739817e-13;
t1379 = t5.*t23.*1.97108120739817e-13;
t1382 = t7.*t9.*t18.*3.625084017661248e-13;
t1383 = t7.*t9.*t18.*3.625084017661248e-13;
t1384 = t4.*t5.*t8.*t17.*(-8.217441799717035e-14);
t1388 = -t1361;
t1391 = -t1363;
t1392 = -t1362;
t1395 = t3.*t7.*t18.*4.360923755161119e-7;
t1396 = t4.*t8.*t17.*4.360923755161119e-7;
t1401 = -t1374;
t1404 = t3.*t5.*t18.*3.625084017661248e-13;
t1405 = t3.*t5.*t18.*3.625084017661248e-13;
t1407 = -t1381;
t1413 = -t1390;
t1414 = -t1389;
t1415 = t5.*t17.*t18.*1.077612036149773e-13;
t1417 = t5.*t17.*t23.*1.077612036149773e-13;
t1420 = t4.*t9.*t17.*3.048693243547943e-13;
t1421 = t4.*t9.*t22.*3.048693243547943e-13;
t1423 = t9.*t17.*t18.*2.324812497785041e-13;
t1424 = -t1400;
t1425 = t9.*t17.*t23.*2.324812497785041e-13;
t1426 = t45+t60+4.36041e-5;
t1428 = t4.*t5.*t8.*t17.*(-2.324812497785041e-13);
t1438 = t5.*t17.*t23.*3.048693243547943e-13;
t1443 = t5.*t17.*t18.*3.048693243547943e-13;
t1444 = -t1437;
t1453 = t15.*3.483029800032151e-7;
t1454 = t15.*3.483029800032151e-7;
t1460 = t76+t83+8.01825475553694e-7;
t1461 = t3.*t18.*6.405761271399419e-7;
t1462 = t3.*t18.*6.405761271399419e-7;
t1464 = -t1456;
t1471 = t74+t75+4.35810366141993e-7;
t1476 = t17.*t18.*1.904211161212082e-7;
t1478 = t17.*t23.*1.904211161212082e-7;
t1482 = -t1477;
t1484 = t17.*t18.*5.387240961244234e-7;
t1486 = t17.*t23.*5.387240961244234e-7;
t1521 = -t1504;
t1522 = -t1505;
t1565 = t5.*t1504;
t1566 = t9.*t1504;
t1568 = t9.*t1505;
t1580 = -t1547;
t1589 = -t1552;
t1591 = -t1554;
t1595 = -t1559;
t1597 = t5.*t1532;
t1598 = t5.*t1533;
t1599 = -t1563;
t1603 = t9.*t1533;
t1605 = t9.*t1535;
t1629 = t5.*t1552;
t1634 = t5.*t1554;
t1635 = t9.*t1552;
t1636 = t5.*t1558;
t1640 = t9.*t1554;
t1641 = t5.*t1560;
t1643 = t9.*t1558;
t1663 = -t1604;
t1669 = -t1608;
t1711 = -t1632;
t1725 = t5.*t1604;
t1728 = t9.*t1604;
t1731 = -t1654;
t1733 = -t1658;
t1735 = t9.*t1608;
t1738 = t5.*t1610;
t1740 = -t1664;
t1744 = -t1668;
t1755 = -t1677;
t1756 = -t1678;
t1757 = -t1680;
t1758 = -t1679;
t1760 = -t1684;
t1761 = -t1685;
t1764 = -t1688;
t1767 = -t1693;
t1769 = -t1694;
t1774 = -t1703;
t1778 = t8.*t1632;
t1779 = t5.*t1637;
t1787 = t8.*t1638;
t1788 = t9.*t1637;
t1789 = t8.*t1639;
t1804 = t9.*t1644;
t1807 = -t1714;
t1814 = -t1717;
t1817 = t5.*t1652;
t1826 = t8.*t1654;
t1830 = -t1727;
t1831 = t8.*t1659;
t1832 = t8.*t1660;
t1834 = t9.*t1658;
t1835 = t8.*t1661;
t1836 = t8.*t1662;
t1843 = t9.*t1666;
t1847 = t8.*t1668;
t1866 = -t1750;
t1867 = -t1751;
t1872 = t8.*t1694;
t1874 = t8.*t1695;
t1890 = t5.*t1714;
t1894 = t9.*t1714;
t1896 = t5.*t1720;
t1903 = -t1796;
t1910 = t9.*t1722;
t1920 = -t1819;
t1936 = -t1840;
t1937 = -t1842;
t1938 = -t1841;
t1943 = t8.*t1746;
t1944 = t5.*t1749;
t1945 = t5.*t1750;
t1950 = -t1852;
t1955 = t5.*t1683;
t1957 = t8.*t1677;
t1959 = t8.*t1678;
t1961 = t9.*t1676;
t1962 = t8.*t1680;
t1966 = t9.*t1682;
t1967 = t9.*t1683;
t1969 = t5.*t1688;
t1970 = t9.*t1684;
t1976 = -t1871;
t1981 = -t1876;
t1988 = t5.*t1785;
t1992 = -t1883;
t1996 = t8.*t1797;
t1998 = t9.*t1796;
t1999 = t8.*t1799;
t2000 = t8.*t1801;
t2001 = t5.*t1810;
t2004 = -t1895;
t2005 = -t1898;
t2006 = -t1897;
t2007 = t9.*t1809;
t2013 = t8.*t1819;
t2019 = -t1923;
t2020 = -t1924;
t2023 = t8.*t1838;
t2029 = t9.*t1840;
t2030 = t8.*t1841;
t2031 = t8.*t1842;
t2033 = t5.*t1850;
t2036 = -t1931;
t2037 = -t1933;
t2038 = -t1932;
t2042 = t5.*t1857;
t2048 = t8.*t1852;
t2052 = t8.*t1858;
t2053 = t9.*t1857;
t2059 = -t1949;
t2060 = -t1948;
t2066 = -t1956;
t2068 = -t1958;
t2069 = -t1960;
t2074 = -t1963;
t2108 = t8.*t1914;
t2109 = t9.*t1911;
t2111 = t8.*t1915;
t2112 = t9.*t1912;
t2114 = t8.*t1916;
t2116 = t5.*t1923;
t2118 = -t2012;
t2120 = t5.*t1931;
t2124 = t9.*t1931;
t2128 = -t2022;
t2129 = -t2024;
t2130 = -t2025;
t2133 = -t2032;
t2142 = -t2046;
t2148 = -t2063;
t2149 = -t2064;
t2157 = -t2093;
t2204 = t9.*t2063;
t2206 = t8.*t2064;
t2208 = t5.*t2072;
t2212 = t5.*t2081;
t2217 = t9.*t2081;
t2218 = t8.*t2086;
t2219 = t9.*t2082;
t2221 = t8.*t2087;
t2227 = t8.*t1978;
t2229 = t8.*t1979;
t2251 = -t2173;
t2256 = -t2183;
t2257 = -t2188;
t2266 = -t2205;
t2267 = -t2207;
t2274 = -t2228;
t2316 = -t2277;
t2317 = -t2279;
t2318 = -t2282;
t2357 = -t2324;
t2358 = -t2325;
t2359 = -t2329;
C_dq = ft_3({dq1,dq2,dq3,dq4,dq5,dq6,t100,t1000,t1003,t1004,t1005,t1006,t1007,t101,t1012,t1013,t1014,t1015,t1016,t102,t1023,t1024,t1026,t1027,t1028,t1029,t1030,t1034,t1038,t1039,t104,t1040,t1041,t1042,t1044,t1045,t1047,t1048,t1049,t105,t1050,t1052,t1058,t1059,t106,t1062,t1063,t1064,t1066,t1068,t1069,t107,t1070,t1071,t1078,t108,t1080,t1081,t1086,t109,t1091,t1092,t1093,t1094,t1096,t1097,t1098,t1099,t110,t1100,t1101,t1102,t1103,t1105,t1106,t1108,t1109,t111,t1111,t1113,t1115,t1116,t1117,t1118,t1119,t112,t1123,t1126,t1128,t1129,t113,t1130,t1133,t1134,t1137,t1138,t1139,t114,t1140,t1141,t1144,t115,t1150,t1151,t1152,t1153,t1155,t1158,t1159,t116,t1161,t1162,t1163,t1164,t1167,t1169,t117,t1170,t1171,t1176,t1177,t1178,t118,t1182,t1185,t1186,t1187,t1188,t1189,t119,t1195,t1196,t120,t1204,t1205,t1207,t1208,t121,t1210,t1214,t1215,t1216,t1218,t1219,t122,t1221,t1222,t1223,t1225,t1226,t1229,t123,t1231,t1232,t1233,t1236,t1238,t124,t1240,t1243,t1244,t1245,t1246,t1247,t125,t1250,t1251,t1253,t1254,t1255,t1256,t1258,t1259,t126,t1260,t1261,t1264,t1266,t1272,t1273,t1274,t1275,t1276,t1278,t1279,t128,t1280,t1281,t1282,t1283,t1284,t1285,t1286,t1288,t129,t1298,t130,t1300,t1301,t1302,t1304,t1307,t1308,t1309,t131,t1310,t1312,t1313,t1315,t1316,t1319,t132,t1321,t1322,t1324,t1326,t1327,t1328,t1329,t133,t1330,t1331,t1332,t1335,t1337,t1338,t1339,t134,t1340,t1341,t1344,t1345,t1347,t1348,t1349,t135,t1351,t1352,t1356,t1357,t1358,t1359,t136,t1360,t1362,t1364,t1365,t1366,t1367,t1368,t1369,t137,t1370,t1371,t1372,t1373,t1374,t1375,t1376,t1378,t1379,t1380,t1382,t1383,t1384,t1388,t1389,t139,t1391,t1392,t1393,t1395,t1396,t140,t1401,t1404,t1405,t1407,t1409,t141,t1411,t1413,t1414,t1415,t1416,t1417,t142,t1420,t1421,t1423,t1424,t1425,t1426,t1428,t143,t1438,t144,t1443,t1444,t1449,t145,t1453,t1454,t1456,t1457,t146,t1460,t1461,t1462,t1464,t147,t1471,t1476,t1478,t148,t1482,t1484,t1485,t1486,t15,t150,t1505,t151,t152,t1521,t1522,t153,t1532,t1533,t1535,t154,t1549,t155,t1558,t1560,t1566,t1568,t157,t158,t1580,t1589,t1591,t1595,t1596,t1597,t1598,t1599,t16,t1605,t1606,t161,t1610,t1611,t1612,t1619,t162,t163,t1631,t1632,t1635,t1636,t1637,t1638,t1639,t164,t1641,t1643,t1644,t1645,t165,t1651,t1652,t1653,t1657,t1658,t1659,t166,t1660,t1661,t1662,t1663,t1666,t1669,t1676,t168,t1682,t1683,t1689,t169,t1692,t1695,t1696,t1698,t17,t170,t1702,t1703,t1709,t1711,t1712,t1713,t1716,t172,t1720,t1722,t1726,t1728,t1729,t173,t1731,t1733,t1734,t1735,t1736,t1737,t1738,t174,t1740,t1744,t1745,t1746,t1749,t175,t1752,t1755,t1756,t1757,t1758,t176,t1760,t1761,t1764,t1767,t1769,t177,t1774,t1779,t1785,t1786,t1787,t1788,t1789,t179,t1797,t1798,t1799,t18,t180,t1800,t1801,t1804,t1807,t1809,t181,t1810,t1814,t1816,t1817,t182,t1826,t1827,t1829,t183,t1830,t1831,t1832,t1833,t1834,t1835,t1836,t1838,t1847,t1849,t185,t1850,t1851,t1857,t1858,t1859,t186,t1866,t1867,t1871,t1872,t1873,t188,t1881,t1882,t1889,t1896,t19,t190,t1903,t1907,t191,t1910,t1911,t1912,t1913,t1914,t1915,t1916,t192,t1920,t1925,t1926,t1935,t1936,t1937,t1938,t1939,t1943,t1944,t1950,t1955,t1961,t1966,t1967,t1968,t1969,t1970,t1976,t1977,t1978,t1979,t1981,t1988,t1992,t1994,t1995,t1996,t1997,t1998,t1999,t2,t20,t2000,t2001,t2003,t2004,t2005,t2006,t2019,t2020,t2023,t2024,t2028,t2029,t2033,t2036,t2037,t2038,t2042,t2052,t2053,t2056,t2058,t2059,t206,t2060,t2065,t2066,t2067,t2068,t2069,t207,t2070,t2072,t2073,t2074,t2079,t2081,t2082,t2083,t2084,t2085,t2086,t2087,t2093,t2094,t2098,t21,t2100,t2103,t2104,t2105,t2106,t2108,t2109,t2110,t2111,t2113,t2114,t2115,t2116,t2117,t2118,t2128,t2129,t2130,t2131,t2132,t2133,t2142,t2144,t2148,t2149,t215,t2156,t2157,t216,t2171,t2172,t2175,t2176,t2179,t2180,t2182,t2189,t219,t2194,t22,t220,t2204,t2208,t221,t2212,t2217,t2218,t2219,t222,t2220,t2221,t2223,t2227,t2228,t2229,t223,t224,t225,t2251,t2256,t2257,t226,t2265,t2266,t2267,t227,t2274,t2277,t2279,t228,t2280,t2281,t2282,t2285,t2294,t23,t230,t2302,t2304,t2305,t2306,t231,t2316,t2317,t2318,t2321,t2322,t2323,t2324,t233,t2336,t2339,t234,t2340,t2344,t2348,t2349,t235,t2350,t2352,t2353,t2356,t2357,t2358,t2359,t236,t2360,t2361,t2362,t2363,t2364,t2365,t237,t2373,t2375,t2376,t2377,t2378,t2379,t238,t2380,t239,t24,t240,t2409,t241,t2412,t242,t2428,t2429,t243,t2430,t2432,t2433,t2435,t2436,t2438,t2439,t244,t2440,t2441,t2443,t245,t2456,t246,t247,t2470,t2474,t2475,t2476,t248,t2481,t2486,t2487,t2488,t2489,t249,t2491,t2493,t2495,t2496,t2497,t25,t2516,t252,t2521,t2527,t2528,t2529,t253,t2533,t254,t256,t257,t258,t259,t26,t260,t261,t263,t264,t266,t269,t27,t270,t272,t273,t274,t275,t276,t277,t278,t279,t28,t280,t281,t284,t285,t286,t287,t288,t2886,t289,t29,t290,t291,t292,t293,t294,t2953,t296,t297,t299,t3,t30,t300,t302,t303,t304,t305,t306,t307,t308,t309,t310,t311,t312,t313,t314,t315,t316,t317,t318,t319,t32,t320,t321,t322,t324,t325,t327,t328,t329,t33,t331,t332,t333,t334,t336,t337,t338,t34,t340,t341,t343,t344,t345,t346,t347,t348,t35,t350,t352,t353,t354,t355,t356,t357,t358,t359,t360,t362,t365,t366,t367,t368,t369,t37,t371,t372,t373,t374,t375,t376,t377,t378,t379,t38,t380,t382,t384,t386,t387,t388,t389,t391,t392,t395,t396,t398,t4,t40,t400,t401,t402,t403,t404,t406,t409,t41,t410,t411,t412,t413,t414,t415,t416,t417,t418,t419,t420,t421,t423,t424,t425,t426,t427,t428,t429,t431,t433,t434,t436,t437,t438,t439,t44,t440,t441,t442,t443,t444,t445,t446,t447,t448,t449,t45,t450,t451,t452,t453,t454,t456,t457,t458,t459,t46,t462,t463,t464,t465,t466,t468,t469,t47,t471,t472,t48,t480,t481,t482,t483,t484,t485,t488,t489,t49,t491,t492,t493,t494,t495,t496,t497,t498,t499,t5,t50,t500,t501,t502,t503,t504,t505,t506,t507,t508,t509,t51,t510,t511,t512,t513,t514,t515,t516,t517,t52,t521,t522,t526,t527,t528,t529,t53,t530,t531,t532,t533,t534,t535,t536,t537,t538,t539,t540,t543,t544,t545,t546,t548,t549,t551,t552,t553,t554,t555,t556,t557,t558,t559,t56,t560,t561,t562,t563,t564,t567,t568,t569,t57,t570,t571,t572,t573,t574,t576,t577,t578,t58,t580,t581,t582,t583,t584,t585,t586,t587,t588,t59,t590,t591,t592,t593,t595,t596,t6,t60,t605,t607,t609,t61,t610,t612,t613,t614,t623,t625,t626,t629,t63,t638,t65,t655,t656,t66,t660,t662,t663,t664,t668,t67,t673,t674,t675,t676,t68,t682,t683,t685,t686,t687,t688,t689,t690,t693,t694,t695,t696,t697,t698,t7,t700,t702,t703,t704,t705,t706,t71,t711,t713,t715,t716,t718,t719,t72,t721,t722,t724,t725,t727,t728,t73,t731,t733,t734,t735,t736,t74,t744,t745,t746,t747,t748,t749,t75,t750,t751,t752,t755,t756,t757,t758,t759,t76,t762,t763,t764,t765,t766,t768,t769,t77,t780,t785,t786,t787,t788,t79,t791,t793,t795,t8,t80,t804,t805,t808,t81,t814,t815,t816,t818,t819,t82,t820,t821,t822,t825,t827,t83,t837,t838,t84,t840,t841,t842,t843,t846,t849,t851,t855,t857,t86,t862,t864,t87,t874,t88,t882,t884,t885,t888,t891,t892,t895,t897,t899,t9,t90,t900,t903,t904,t906,t911,t92,t921,t922,t923,t924,t926,t927,t93,t934,t935,t936,t937,t94,t940,t941,t942,t946,t949,t95,t950,t956,t957,t958,t96,t960,t961,t962,t964,t966,t967,t968,t969,t97,t970,t971,t972,t977,t979,t98,t981,t982,t983,t984,t986,t988,t989,t99,t992,t993,t994,t995,t996,t997,t999});
end
function C_dq = ft_3(ct)
dq1 = ct{1};
dq2 = ct{2};
dq3 = ct{3};
dq4 = ct{4};
dq5 = ct{5};
dq6 = ct{6};
t100 = ct{7};
t1000 = ct{8};
t1003 = ct{9};
t1004 = ct{10};
t1005 = ct{11};
t1006 = ct{12};
t1007 = ct{13};
t101 = ct{14};
t1012 = ct{15};
t1013 = ct{16};
t1014 = ct{17};
t1015 = ct{18};
t1016 = ct{19};
t102 = ct{20};
t1023 = ct{21};
t1024 = ct{22};
t1026 = ct{23};
t1027 = ct{24};
t1028 = ct{25};
t1029 = ct{26};
t1030 = ct{27};
t1034 = ct{28};
t1038 = ct{29};
t1039 = ct{30};
t104 = ct{31};
t1040 = ct{32};
t1041 = ct{33};
t1042 = ct{34};
t1044 = ct{35};
t1045 = ct{36};
t1047 = ct{37};
t1048 = ct{38};
t1049 = ct{39};
t105 = ct{40};
t1050 = ct{41};
t1052 = ct{42};
t1058 = ct{43};
t1059 = ct{44};
t106 = ct{45};
t1062 = ct{46};
t1063 = ct{47};
t1064 = ct{48};
t1066 = ct{49};
t1068 = ct{50};
t1069 = ct{51};
t107 = ct{52};
t1070 = ct{53};
t1071 = ct{54};
t1078 = ct{55};
t108 = ct{56};
t1080 = ct{57};
t1081 = ct{58};
t1086 = ct{59};
t109 = ct{60};
t1091 = ct{61};
t1092 = ct{62};
t1093 = ct{63};
t1094 = ct{64};
t1096 = ct{65};
t1097 = ct{66};
t1098 = ct{67};
t1099 = ct{68};
t110 = ct{69};
t1100 = ct{70};
t1101 = ct{71};
t1102 = ct{72};
t1103 = ct{73};
t1105 = ct{74};
t1106 = ct{75};
t1108 = ct{76};
t1109 = ct{77};
t111 = ct{78};
t1111 = ct{79};
t1113 = ct{80};
t1115 = ct{81};
t1116 = ct{82};
t1117 = ct{83};
t1118 = ct{84};
t1119 = ct{85};
t112 = ct{86};
t1123 = ct{87};
t1126 = ct{88};
t1128 = ct{89};
t1129 = ct{90};
t113 = ct{91};
t1130 = ct{92};
t1133 = ct{93};
t1134 = ct{94};
t1137 = ct{95};
t1138 = ct{96};
t1139 = ct{97};
t114 = ct{98};
t1140 = ct{99};
t1141 = ct{100};
t1144 = ct{101};
t115 = ct{102};
t1150 = ct{103};
t1151 = ct{104};
t1152 = ct{105};
t1153 = ct{106};
t1155 = ct{107};
t1158 = ct{108};
t1159 = ct{109};
t116 = ct{110};
t1161 = ct{111};
t1162 = ct{112};
t1163 = ct{113};
t1164 = ct{114};
t1167 = ct{115};
t1169 = ct{116};
t117 = ct{117};
t1170 = ct{118};
t1171 = ct{119};
t1176 = ct{120};
t1177 = ct{121};
t1178 = ct{122};
t118 = ct{123};
t1182 = ct{124};
t1185 = ct{125};
t1186 = ct{126};
t1187 = ct{127};
t1188 = ct{128};
t1189 = ct{129};
t119 = ct{130};
t1195 = ct{131};
t1196 = ct{132};
t120 = ct{133};
t1204 = ct{134};
t1205 = ct{135};
t1207 = ct{136};
t1208 = ct{137};
t121 = ct{138};
t1210 = ct{139};
t1214 = ct{140};
t1215 = ct{141};
t1216 = ct{142};
t1218 = ct{143};
t1219 = ct{144};
t122 = ct{145};
t1221 = ct{146};
t1222 = ct{147};
t1223 = ct{148};
t1225 = ct{149};
t1226 = ct{150};
t1229 = ct{151};
t123 = ct{152};
t1231 = ct{153};
t1232 = ct{154};
t1233 = ct{155};
t1236 = ct{156};
t1238 = ct{157};
t124 = ct{158};
t1240 = ct{159};
t1243 = ct{160};
t1244 = ct{161};
t1245 = ct{162};
t1246 = ct{163};
t1247 = ct{164};
t125 = ct{165};
t1250 = ct{166};
t1251 = ct{167};
t1253 = ct{168};
t1254 = ct{169};
t1255 = ct{170};
t1256 = ct{171};
t1258 = ct{172};
t1259 = ct{173};
t126 = ct{174};
t1260 = ct{175};
t1261 = ct{176};
t1264 = ct{177};
t1266 = ct{178};
t1272 = ct{179};
t1273 = ct{180};
t1274 = ct{181};
t1275 = ct{182};
t1276 = ct{183};
t1278 = ct{184};
t1279 = ct{185};
t128 = ct{186};
t1280 = ct{187};
t1281 = ct{188};
t1282 = ct{189};
t1283 = ct{190};
t1284 = ct{191};
t1285 = ct{192};
t1286 = ct{193};
t1288 = ct{194};
t129 = ct{195};
t1298 = ct{196};
t130 = ct{197};
t1300 = ct{198};
t1301 = ct{199};
t1302 = ct{200};
t1304 = ct{201};
t1307 = ct{202};
t1308 = ct{203};
t1309 = ct{204};
t131 = ct{205};
t1310 = ct{206};
t1312 = ct{207};
t1313 = ct{208};
t1315 = ct{209};
t1316 = ct{210};
t1319 = ct{211};
t132 = ct{212};
t1321 = ct{213};
t1322 = ct{214};
t1324 = ct{215};
t1326 = ct{216};
t1327 = ct{217};
t1328 = ct{218};
t1329 = ct{219};
t133 = ct{220};
t1330 = ct{221};
t1331 = ct{222};
t1332 = ct{223};
t1335 = ct{224};
t1337 = ct{225};
t1338 = ct{226};
t1339 = ct{227};
t134 = ct{228};
t1340 = ct{229};
t1341 = ct{230};
t1344 = ct{231};
t1345 = ct{232};
t1347 = ct{233};
t1348 = ct{234};
t1349 = ct{235};
t135 = ct{236};
t1351 = ct{237};
t1352 = ct{238};
t1356 = ct{239};
t1357 = ct{240};
t1358 = ct{241};
t1359 = ct{242};
t136 = ct{243};
t1360 = ct{244};
t1362 = ct{245};
t1364 = ct{246};
t1365 = ct{247};
t1366 = ct{248};
t1367 = ct{249};
t1368 = ct{250};
t1369 = ct{251};
t137 = ct{252};
t1370 = ct{253};
t1371 = ct{254};
t1372 = ct{255};
t1373 = ct{256};
t1374 = ct{257};
t1375 = ct{258};
t1376 = ct{259};
t1378 = ct{260};
t1379 = ct{261};
t1380 = ct{262};
t1382 = ct{263};
t1383 = ct{264};
t1384 = ct{265};
t1388 = ct{266};
t1389 = ct{267};
t139 = ct{268};
t1391 = ct{269};
t1392 = ct{270};
t1393 = ct{271};
t1395 = ct{272};
t1396 = ct{273};
t140 = ct{274};
t1401 = ct{275};
t1404 = ct{276};
t1405 = ct{277};
t1407 = ct{278};
t1409 = ct{279};
t141 = ct{280};
t1411 = ct{281};
t1413 = ct{282};
t1414 = ct{283};
t1415 = ct{284};
t1416 = ct{285};
t1417 = ct{286};
t142 = ct{287};
t1420 = ct{288};
t1421 = ct{289};
t1423 = ct{290};
t1424 = ct{291};
t1425 = ct{292};
t1426 = ct{293};
t1428 = ct{294};
t143 = ct{295};
t1438 = ct{296};
t144 = ct{297};
t1443 = ct{298};
t1444 = ct{299};
t1449 = ct{300};
t145 = ct{301};
t1453 = ct{302};
t1454 = ct{303};
t1456 = ct{304};
t1457 = ct{305};
t146 = ct{306};
t1460 = ct{307};
t1461 = ct{308};
t1462 = ct{309};
t1464 = ct{310};
t147 = ct{311};
t1471 = ct{312};
t1476 = ct{313};
t1478 = ct{314};
t148 = ct{315};
t1482 = ct{316};
t1484 = ct{317};
t1485 = ct{318};
t1486 = ct{319};
t15 = ct{320};
t150 = ct{321};
t1505 = ct{322};
t151 = ct{323};
t152 = ct{324};
t1521 = ct{325};
t1522 = ct{326};
t153 = ct{327};
t1532 = ct{328};
t1533 = ct{329};
t1535 = ct{330};
t154 = ct{331};
t1549 = ct{332};
t155 = ct{333};
t1558 = ct{334};
t1560 = ct{335};
t1566 = ct{336};
t1568 = ct{337};
t157 = ct{338};
t158 = ct{339};
t1580 = ct{340};
t1589 = ct{341};
t1591 = ct{342};
t1595 = ct{343};
t1596 = ct{344};
t1597 = ct{345};
t1598 = ct{346};
t1599 = ct{347};
t16 = ct{348};
t1605 = ct{349};
t1606 = ct{350};
t161 = ct{351};
t1610 = ct{352};
t1611 = ct{353};
t1612 = ct{354};
t1619 = ct{355};
t162 = ct{356};
t163 = ct{357};
t1631 = ct{358};
t1632 = ct{359};
t1635 = ct{360};
t1636 = ct{361};
t1637 = ct{362};
t1638 = ct{363};
t1639 = ct{364};
t164 = ct{365};
t1641 = ct{366};
t1643 = ct{367};
t1644 = ct{368};
t1645 = ct{369};
t165 = ct{370};
t1651 = ct{371};
t1652 = ct{372};
t1653 = ct{373};
t1657 = ct{374};
t1658 = ct{375};
t1659 = ct{376};
t166 = ct{377};
t1660 = ct{378};
t1661 = ct{379};
t1662 = ct{380};
t1663 = ct{381};
t1666 = ct{382};
t1669 = ct{383};
t1676 = ct{384};
t168 = ct{385};
t1682 = ct{386};
t1683 = ct{387};
t1689 = ct{388};
t169 = ct{389};
t1692 = ct{390};
t1695 = ct{391};
t1696 = ct{392};
t1698 = ct{393};
t17 = ct{394};
t170 = ct{395};
t1702 = ct{396};
t1703 = ct{397};
t1709 = ct{398};
t1711 = ct{399};
t1712 = ct{400};
t1713 = ct{401};
t1716 = ct{402};
t172 = ct{403};
t1720 = ct{404};
t1722 = ct{405};
t1726 = ct{406};
t1728 = ct{407};
t1729 = ct{408};
t173 = ct{409};
t1731 = ct{410};
t1733 = ct{411};
t1734 = ct{412};
t1735 = ct{413};
t1736 = ct{414};
t1737 = ct{415};
t1738 = ct{416};
t174 = ct{417};
t1740 = ct{418};
t1744 = ct{419};
t1745 = ct{420};
t1746 = ct{421};
t1749 = ct{422};
t175 = ct{423};
t1752 = ct{424};
t1755 = ct{425};
t1756 = ct{426};
t1757 = ct{427};
t1758 = ct{428};
t176 = ct{429};
t1760 = ct{430};
t1761 = ct{431};
t1764 = ct{432};
t1767 = ct{433};
t1769 = ct{434};
t177 = ct{435};
t1774 = ct{436};
t1779 = ct{437};
t1785 = ct{438};
t1786 = ct{439};
t1787 = ct{440};
t1788 = ct{441};
t1789 = ct{442};
t179 = ct{443};
t1797 = ct{444};
t1798 = ct{445};
t1799 = ct{446};
t18 = ct{447};
t180 = ct{448};
t1800 = ct{449};
t1801 = ct{450};
t1804 = ct{451};
t1807 = ct{452};
t1809 = ct{453};
t181 = ct{454};
t1810 = ct{455};
t1814 = ct{456};
t1816 = ct{457};
t1817 = ct{458};
t182 = ct{459};
t1826 = ct{460};
t1827 = ct{461};
t1829 = ct{462};
t183 = ct{463};
t1830 = ct{464};
t1831 = ct{465};
t1832 = ct{466};
t1833 = ct{467};
t1834 = ct{468};
t1835 = ct{469};
t1836 = ct{470};
t1838 = ct{471};
t1847 = ct{472};
t1849 = ct{473};
t185 = ct{474};
t1850 = ct{475};
t1851 = ct{476};
t1857 = ct{477};
t1858 = ct{478};
t1859 = ct{479};
t186 = ct{480};
t1866 = ct{481};
t1867 = ct{482};
t1871 = ct{483};
t1872 = ct{484};
t1873 = ct{485};
t188 = ct{486};
t1881 = ct{487};
t1882 = ct{488};
t1889 = ct{489};
t1896 = ct{490};
t19 = ct{491};
t190 = ct{492};
t1903 = ct{493};
t1907 = ct{494};
t191 = ct{495};
t1910 = ct{496};
t1911 = ct{497};
t1912 = ct{498};
t1913 = ct{499};
t1914 = ct{500};
t1915 = ct{501};
t1916 = ct{502};
t192 = ct{503};
t1920 = ct{504};
t1925 = ct{505};
t1926 = ct{506};
t1935 = ct{507};
t1936 = ct{508};
t1937 = ct{509};
t1938 = ct{510};
t1939 = ct{511};
t1943 = ct{512};
t1944 = ct{513};
t1950 = ct{514};
t1955 = ct{515};
t1961 = ct{516};
t1966 = ct{517};
t1967 = ct{518};
t1968 = ct{519};
t1969 = ct{520};
t1970 = ct{521};
t1976 = ct{522};
t1977 = ct{523};
t1978 = ct{524};
t1979 = ct{525};
t1981 = ct{526};
t1988 = ct{527};
t1992 = ct{528};
t1994 = ct{529};
t1995 = ct{530};
t1996 = ct{531};
t1997 = ct{532};
t1998 = ct{533};
t1999 = ct{534};
t2 = ct{535};
t20 = ct{536};
t2000 = ct{537};
t2001 = ct{538};
t2003 = ct{539};
t2004 = ct{540};
t2005 = ct{541};
t2006 = ct{542};
t2019 = ct{543};
t2020 = ct{544};
t2023 = ct{545};
t2024 = ct{546};
t2028 = ct{547};
t2029 = ct{548};
t2033 = ct{549};
t2036 = ct{550};
t2037 = ct{551};
t2038 = ct{552};
t2042 = ct{553};
t2052 = ct{554};
t2053 = ct{555};
t2056 = ct{556};
t2058 = ct{557};
t2059 = ct{558};
t206 = ct{559};
t2060 = ct{560};
t2065 = ct{561};
t2066 = ct{562};
t2067 = ct{563};
t2068 = ct{564};
t2069 = ct{565};
t207 = ct{566};
t2070 = ct{567};
t2072 = ct{568};
t2073 = ct{569};
t2074 = ct{570};
t2079 = ct{571};
t2081 = ct{572};
t2082 = ct{573};
t2083 = ct{574};
t2084 = ct{575};
t2085 = ct{576};
t2086 = ct{577};
t2087 = ct{578};
t2093 = ct{579};
t2094 = ct{580};
t2098 = ct{581};
t21 = ct{582};
t2100 = ct{583};
t2103 = ct{584};
t2104 = ct{585};
t2105 = ct{586};
t2106 = ct{587};
t2108 = ct{588};
t2109 = ct{589};
t2110 = ct{590};
t2111 = ct{591};
t2113 = ct{592};
t2114 = ct{593};
t2115 = ct{594};
t2116 = ct{595};
t2117 = ct{596};
t2118 = ct{597};
t2128 = ct{598};
t2129 = ct{599};
t2130 = ct{600};
t2131 = ct{601};
t2132 = ct{602};
t2133 = ct{603};
t2142 = ct{604};
t2144 = ct{605};
t2148 = ct{606};
t2149 = ct{607};
t215 = ct{608};
t2156 = ct{609};
t2157 = ct{610};
t216 = ct{611};
t2171 = ct{612};
t2172 = ct{613};
t2175 = ct{614};
t2176 = ct{615};
t2179 = ct{616};
t2180 = ct{617};
t2182 = ct{618};
t2189 = ct{619};
t219 = ct{620};
t2194 = ct{621};
t22 = ct{622};
t220 = ct{623};
t2204 = ct{624};
t2208 = ct{625};
t221 = ct{626};
t2212 = ct{627};
t2217 = ct{628};
t2218 = ct{629};
t2219 = ct{630};
t222 = ct{631};
t2220 = ct{632};
t2221 = ct{633};
t2223 = ct{634};
t2227 = ct{635};
t2228 = ct{636};
t2229 = ct{637};
t223 = ct{638};
t224 = ct{639};
t225 = ct{640};
t2251 = ct{641};
t2256 = ct{642};
t2257 = ct{643};
t226 = ct{644};
t2265 = ct{645};
t2266 = ct{646};
t2267 = ct{647};
t227 = ct{648};
t2274 = ct{649};
t2277 = ct{650};
t2279 = ct{651};
t228 = ct{652};
t2280 = ct{653};
t2281 = ct{654};
t2282 = ct{655};
t2285 = ct{656};
t2294 = ct{657};
t23 = ct{658};
t230 = ct{659};
t2302 = ct{660};
t2304 = ct{661};
t2305 = ct{662};
t2306 = ct{663};
t231 = ct{664};
t2316 = ct{665};
t2317 = ct{666};
t2318 = ct{667};
t2321 = ct{668};
t2322 = ct{669};
t2323 = ct{670};
t2324 = ct{671};
t233 = ct{672};
t2336 = ct{673};
t2339 = ct{674};
t234 = ct{675};
t2340 = ct{676};
t2344 = ct{677};
t2348 = ct{678};
t2349 = ct{679};
t235 = ct{680};
t2350 = ct{681};
t2352 = ct{682};
t2353 = ct{683};
t2356 = ct{684};
t2357 = ct{685};
t2358 = ct{686};
t2359 = ct{687};
t236 = ct{688};
t2360 = ct{689};
t2361 = ct{690};
t2362 = ct{691};
t2363 = ct{692};
t2364 = ct{693};
t2365 = ct{694};
t237 = ct{695};
t2373 = ct{696};
t2375 = ct{697};
t2376 = ct{698};
t2377 = ct{699};
t2378 = ct{700};
t2379 = ct{701};
t238 = ct{702};
t2380 = ct{703};
t239 = ct{704};
t24 = ct{705};
t240 = ct{706};
t2409 = ct{707};
t241 = ct{708};
t2412 = ct{709};
t242 = ct{710};
t2428 = ct{711};
t2429 = ct{712};
t243 = ct{713};
t2430 = ct{714};
t2432 = ct{715};
t2433 = ct{716};
t2435 = ct{717};
t2436 = ct{718};
t2438 = ct{719};
t2439 = ct{720};
t244 = ct{721};
t2440 = ct{722};
t2441 = ct{723};
t2443 = ct{724};
t245 = ct{725};
t2456 = ct{726};
t246 = ct{727};
t247 = ct{728};
t2470 = ct{729};
t2474 = ct{730};
t2475 = ct{731};
t2476 = ct{732};
t248 = ct{733};
t2481 = ct{734};
t2486 = ct{735};
t2487 = ct{736};
t2488 = ct{737};
t2489 = ct{738};
t249 = ct{739};
t2491 = ct{740};
t2493 = ct{741};
t2495 = ct{742};
t2496 = ct{743};
t2497 = ct{744};
t25 = ct{745};
t2516 = ct{746};
t252 = ct{747};
t2521 = ct{748};
t2527 = ct{749};
t2528 = ct{750};
t2529 = ct{751};
t253 = ct{752};
t2533 = ct{753};
t254 = ct{754};
t256 = ct{755};
t257 = ct{756};
t258 = ct{757};
t259 = ct{758};
t26 = ct{759};
t260 = ct{760};
t261 = ct{761};
t263 = ct{762};
t264 = ct{763};
t266 = ct{764};
t269 = ct{765};
t27 = ct{766};
t270 = ct{767};
t272 = ct{768};
t273 = ct{769};
t274 = ct{770};
t275 = ct{771};
t276 = ct{772};
t277 = ct{773};
t278 = ct{774};
t279 = ct{775};
t28 = ct{776};
t280 = ct{777};
t281 = ct{778};
t284 = ct{779};
t285 = ct{780};
t286 = ct{781};
t287 = ct{782};
t288 = ct{783};
t2886 = ct{784};
t289 = ct{785};
t29 = ct{786};
t290 = ct{787};
t291 = ct{788};
t292 = ct{789};
t293 = ct{790};
t294 = ct{791};
t2953 = ct{792};
t296 = ct{793};
t297 = ct{794};
t299 = ct{795};
t3 = ct{796};
t30 = ct{797};
t300 = ct{798};
t302 = ct{799};
t303 = ct{800};
t304 = ct{801};
t305 = ct{802};
t306 = ct{803};
t307 = ct{804};
t308 = ct{805};
t309 = ct{806};
t310 = ct{807};
t311 = ct{808};
t312 = ct{809};
t313 = ct{810};
t314 = ct{811};
t315 = ct{812};
t316 = ct{813};
t317 = ct{814};
t318 = ct{815};
t319 = ct{816};
t32 = ct{817};
t320 = ct{818};
t321 = ct{819};
t322 = ct{820};
t324 = ct{821};
t325 = ct{822};
t327 = ct{823};
t328 = ct{824};
t329 = ct{825};
t33 = ct{826};
t331 = ct{827};
t332 = ct{828};
t333 = ct{829};
t334 = ct{830};
t336 = ct{831};
t337 = ct{832};
t338 = ct{833};
t34 = ct{834};
t340 = ct{835};
t341 = ct{836};
t343 = ct{837};
t344 = ct{838};
t345 = ct{839};
t346 = ct{840};
t347 = ct{841};
t348 = ct{842};
t35 = ct{843};
t350 = ct{844};
t352 = ct{845};
t353 = ct{846};
t354 = ct{847};
t355 = ct{848};
t356 = ct{849};
t357 = ct{850};
t358 = ct{851};
t359 = ct{852};
t360 = ct{853};
t362 = ct{854};
t365 = ct{855};
t366 = ct{856};
t367 = ct{857};
t368 = ct{858};
t369 = ct{859};
t37 = ct{860};
t371 = ct{861};
t372 = ct{862};
t373 = ct{863};
t374 = ct{864};
t375 = ct{865};
t376 = ct{866};
t377 = ct{867};
t378 = ct{868};
t379 = ct{869};
t38 = ct{870};
t380 = ct{871};
t382 = ct{872};
t384 = ct{873};
t386 = ct{874};
t387 = ct{875};
t388 = ct{876};
t389 = ct{877};
t391 = ct{878};
t392 = ct{879};
t395 = ct{880};
t396 = ct{881};
t398 = ct{882};
t4 = ct{883};
t40 = ct{884};
t400 = ct{885};
t401 = ct{886};
t402 = ct{887};
t403 = ct{888};
t404 = ct{889};
t406 = ct{890};
t409 = ct{891};
t41 = ct{892};
t410 = ct{893};
t411 = ct{894};
t412 = ct{895};
t413 = ct{896};
t414 = ct{897};
t415 = ct{898};
t416 = ct{899};
t417 = ct{900};
t418 = ct{901};
t419 = ct{902};
t420 = ct{903};
t421 = ct{904};
t423 = ct{905};
t424 = ct{906};
t425 = ct{907};
t426 = ct{908};
t427 = ct{909};
t428 = ct{910};
t429 = ct{911};
t431 = ct{912};
t433 = ct{913};
t434 = ct{914};
t436 = ct{915};
t437 = ct{916};
t438 = ct{917};
t439 = ct{918};
t44 = ct{919};
t440 = ct{920};
t441 = ct{921};
t442 = ct{922};
t443 = ct{923};
t444 = ct{924};
t445 = ct{925};
t446 = ct{926};
t447 = ct{927};
t448 = ct{928};
t449 = ct{929};
t45 = ct{930};
t450 = ct{931};
t451 = ct{932};
t452 = ct{933};
t453 = ct{934};
t454 = ct{935};
t456 = ct{936};
t457 = ct{937};
t458 = ct{938};
t459 = ct{939};
t46 = ct{940};
t462 = ct{941};
t463 = ct{942};
t464 = ct{943};
t465 = ct{944};
t466 = ct{945};
t468 = ct{946};
t469 = ct{947};
t47 = ct{948};
t471 = ct{949};
t472 = ct{950};
t48 = ct{951};
t480 = ct{952};
t481 = ct{953};
t482 = ct{954};
t483 = ct{955};
t484 = ct{956};
t485 = ct{957};
t488 = ct{958};
t489 = ct{959};
t49 = ct{960};
t491 = ct{961};
t492 = ct{962};
t493 = ct{963};
t494 = ct{964};
t495 = ct{965};
t496 = ct{966};
t497 = ct{967};
t498 = ct{968};
t499 = ct{969};
t5 = ct{970};
t50 = ct{971};
t500 = ct{972};
t501 = ct{973};
t502 = ct{974};
t503 = ct{975};
t504 = ct{976};
t505 = ct{977};
t506 = ct{978};
t507 = ct{979};
t508 = ct{980};
t509 = ct{981};
t51 = ct{982};
t510 = ct{983};
t511 = ct{984};
t512 = ct{985};
t513 = ct{986};
t514 = ct{987};
t515 = ct{988};
t516 = ct{989};
t517 = ct{990};
t52 = ct{991};
t521 = ct{992};
t522 = ct{993};
t526 = ct{994};
t527 = ct{995};
t528 = ct{996};
t529 = ct{997};
t53 = ct{998};
t530 = ct{999};
t531 = ct{1000};
t532 = ct{1001};
t533 = ct{1002};
t534 = ct{1003};
t535 = ct{1004};
t536 = ct{1005};
t537 = ct{1006};
t538 = ct{1007};
t539 = ct{1008};
t540 = ct{1009};
t543 = ct{1010};
t544 = ct{1011};
t545 = ct{1012};
t546 = ct{1013};
t548 = ct{1014};
t549 = ct{1015};
t551 = ct{1016};
t552 = ct{1017};
t553 = ct{1018};
t554 = ct{1019};
t555 = ct{1020};
t556 = ct{1021};
t557 = ct{1022};
t558 = ct{1023};
t559 = ct{1024};
t56 = ct{1025};
t560 = ct{1026};
t561 = ct{1027};
t562 = ct{1028};
t563 = ct{1029};
t564 = ct{1030};
t567 = ct{1031};
t568 = ct{1032};
t569 = ct{1033};
t57 = ct{1034};
t570 = ct{1035};
t571 = ct{1036};
t572 = ct{1037};
t573 = ct{1038};
t574 = ct{1039};
t576 = ct{1040};
t577 = ct{1041};
t578 = ct{1042};
t58 = ct{1043};
t580 = ct{1044};
t581 = ct{1045};
t582 = ct{1046};
t583 = ct{1047};
t584 = ct{1048};
t585 = ct{1049};
t586 = ct{1050};
t587 = ct{1051};
t588 = ct{1052};
t59 = ct{1053};
t590 = ct{1054};
t591 = ct{1055};
t592 = ct{1056};
t593 = ct{1057};
t595 = ct{1058};
t596 = ct{1059};
t6 = ct{1060};
t60 = ct{1061};
t605 = ct{1062};
t607 = ct{1063};
t609 = ct{1064};
t61 = ct{1065};
t610 = ct{1066};
t612 = ct{1067};
t613 = ct{1068};
t614 = ct{1069};
t623 = ct{1070};
t625 = ct{1071};
t626 = ct{1072};
t629 = ct{1073};
t63 = ct{1074};
t638 = ct{1075};
t65 = ct{1076};
t655 = ct{1077};
t656 = ct{1078};
t66 = ct{1079};
t660 = ct{1080};
t662 = ct{1081};
t663 = ct{1082};
t664 = ct{1083};
t668 = ct{1084};
t67 = ct{1085};
t673 = ct{1086};
t674 = ct{1087};
t675 = ct{1088};
t676 = ct{1089};
t68 = ct{1090};
t682 = ct{1091};
t683 = ct{1092};
t685 = ct{1093};
t686 = ct{1094};
t687 = ct{1095};
t688 = ct{1096};
t689 = ct{1097};
t690 = ct{1098};
t693 = ct{1099};
t694 = ct{1100};
t695 = ct{1101};
t696 = ct{1102};
t697 = ct{1103};
t698 = ct{1104};
t7 = ct{1105};
t700 = ct{1106};
t702 = ct{1107};
t703 = ct{1108};
t704 = ct{1109};
t705 = ct{1110};
t706 = ct{1111};
t71 = ct{1112};
t711 = ct{1113};
t713 = ct{1114};
t715 = ct{1115};
t716 = ct{1116};
t718 = ct{1117};
t719 = ct{1118};
t72 = ct{1119};
t721 = ct{1120};
t722 = ct{1121};
t724 = ct{1122};
t725 = ct{1123};
t727 = ct{1124};
t728 = ct{1125};
t73 = ct{1126};
t731 = ct{1127};
t733 = ct{1128};
t734 = ct{1129};
t735 = ct{1130};
t736 = ct{1131};
t74 = ct{1132};
t744 = ct{1133};
t745 = ct{1134};
t746 = ct{1135};
t747 = ct{1136};
t748 = ct{1137};
t749 = ct{1138};
t75 = ct{1139};
t750 = ct{1140};
t751 = ct{1141};
t752 = ct{1142};
t755 = ct{1143};
t756 = ct{1144};
t757 = ct{1145};
t758 = ct{1146};
t759 = ct{1147};
t76 = ct{1148};
t762 = ct{1149};
t763 = ct{1150};
t764 = ct{1151};
t765 = ct{1152};
t766 = ct{1153};
t768 = ct{1154};
t769 = ct{1155};
t77 = ct{1156};
t780 = ct{1157};
t785 = ct{1158};
t786 = ct{1159};
t787 = ct{1160};
t788 = ct{1161};
t79 = ct{1162};
t791 = ct{1163};
t793 = ct{1164};
t795 = ct{1165};
t8 = ct{1166};
t80 = ct{1167};
t804 = ct{1168};
t805 = ct{1169};
t808 = ct{1170};
t81 = ct{1171};
t814 = ct{1172};
t815 = ct{1173};
t816 = ct{1174};
t818 = ct{1175};
t819 = ct{1176};
t82 = ct{1177};
t820 = ct{1178};
t821 = ct{1179};
t822 = ct{1180};
t825 = ct{1181};
t827 = ct{1182};
t83 = ct{1183};
t837 = ct{1184};
t838 = ct{1185};
t84 = ct{1186};
t840 = ct{1187};
t841 = ct{1188};
t842 = ct{1189};
t843 = ct{1190};
t846 = ct{1191};
t849 = ct{1192};
t851 = ct{1193};
t855 = ct{1194};
t857 = ct{1195};
t86 = ct{1196};
t862 = ct{1197};
t864 = ct{1198};
t87 = ct{1199};
t874 = ct{1200};
t88 = ct{1201};
t882 = ct{1202};
t884 = ct{1203};
t885 = ct{1204};
t888 = ct{1205};
t891 = ct{1206};
t892 = ct{1207};
t895 = ct{1208};
t897 = ct{1209};
t899 = ct{1210};
t9 = ct{1211};
t90 = ct{1212};
t900 = ct{1213};
t903 = ct{1214};
t904 = ct{1215};
t906 = ct{1216};
t911 = ct{1217};
t92 = ct{1218};
t921 = ct{1219};
t922 = ct{1220};
t923 = ct{1221};
t924 = ct{1222};
t926 = ct{1223};
t927 = ct{1224};
t93 = ct{1225};
t934 = ct{1226};
t935 = ct{1227};
t936 = ct{1228};
t937 = ct{1229};
t94 = ct{1230};
t940 = ct{1231};
t941 = ct{1232};
t942 = ct{1233};
t946 = ct{1234};
t949 = ct{1235};
t95 = ct{1236};
t950 = ct{1237};
t956 = ct{1238};
t957 = ct{1239};
t958 = ct{1240};
t96 = ct{1241};
t960 = ct{1242};
t961 = ct{1243};
t962 = ct{1244};
t964 = ct{1245};
t966 = ct{1246};
t967 = ct{1247};
t968 = ct{1248};
t969 = ct{1249};
t97 = ct{1250};
t970 = ct{1251};
t971 = ct{1252};
t972 = ct{1253};
t977 = ct{1254};
t979 = ct{1255};
t98 = ct{1256};
t981 = ct{1257};
t982 = ct{1258};
t983 = ct{1259};
t984 = ct{1260};
t986 = ct{1261};
t988 = ct{1262};
t989 = ct{1263};
t99 = ct{1264};
t992 = ct{1265};
t993 = ct{1266};
t994 = ct{1267};
t995 = ct{1268};
t996 = ct{1269};
t997 = ct{1270};
t999 = ct{1271};
t2369 = -t2336;
t2372 = -t2339;
t2384 = -t2349;
t2385 = -t2350;
t2387 = -t2352;
t2388 = -t2353;
t2389 = -t2356;
t2391 = -t2360;
t2394 = -t2361;
t2399 = t8.*t2336;
t2400 = t4.*t2340;
t2401 = t8.*t2339;
t2402 = t4.*t2344;
t2403 = t8.*t2340;
t2405 = t8.*t2344;
t2406 = -t2375;
t2407 = -t2380;
t2410 = t8.*t2350;
t2411 = t4.*t2353;
t2413 = t8.*t2352;
t2414 = t4.*t2356;
t2415 = t8.*t2353;
t2417 = t8.*t2356;
t2431 = t8.*t2379;
t2434 = -t2409;
t2437 = -t2412;
t2451 = t8.*t2375;
t2452 = t4.*t2377;
t2453 = t8.*t2376;
t2454 = t4.*t2379;
t2455 = t8.*t2377;
t2457 = -t2432;
t2458 = -t2433;
t2460 = -t2436;
t2483 = -t2475;
t2484 = -t2476;
t2502 = -t2488;
t2505 = -t2489;
t2506 = -t2491;
t2513 = -t2493;
t2518 = -t2496;
t2537 = -t2516;
t2540 = -t2521;
t2544 = -t2528;
t2545 = -t2529;
t2997 = -t2953;
t4763 = t77+t116+t133+t165+t177;
t5361 = t252+t343+t849;
t5777 = t317+t331+t338+t787+t1005;
t31 = -t29;
t91 = t27+t28;
t156 = -t146;
t171 = t8.*t152;
t178 = t8.*t169;
t193 = -t192;
t194 = t190.^2;
t195 = t191.^2;
t196 = t3.*t190;
t197 = t7.*t190;
t198 = t190-1.0;
t349 = t32+t51;
t361 = -t327;
t422 = t15.*t287;
t432 = t38+t65;
t435 = t35+t67;
t455 = t15.*t327;
t460 = t8.*t409;
t461 = t41+t66;
t470 = -t442;
t475 = -t446;
t477 = -t447;
t479 = -t451;
t486 = -t456;
t518 = -t482;
t519 = t53+t56;
t520 = t52+t58;
t523 = -t491;
t524 = -t495;
t525 = -t496;
t547 = -t515;
t575 = t8.*t538;
t579 = t61+t96;
t589 = -t563;
t594 = t75+t94;
t597 = t87+t98;
t598 = t79+t95;
t599 = t86+t93;
t600 = t71+t92;
t601 = t82+t97;
t602 = -t584;
t603 = -t585;
t604 = -t588;
t611 = -t607;
t615 = t111+t137;
t617 = t190.*2.118754404193375e+31;
t618 = -t614;
t633 = t4.*t190.*8.595599785252598e-1;
t634 = t8.*t190.*8.595599785252598e-1;
t640 = t140+t164;
t643 = t4.*t190.*5.157359871151559e-3;
t644 = t8.*t190.*5.157359871151559e-3;
t665 = t5.*t8.*t190.*(-5.157359871151559e-3);
t667 = t8.*t9.*t190.*(-5.157359871151559e-3);
t681 = (t8.*t638)./2.0;
t771 = t8.*t690;
t772 = t5.*t694;
t774 = t9.*t693;
t775 = t9.*t694;
t776 = t8.*t696;
t782 = t9.*t697;
t806 = t8.*t716;
t807 = t5.*t719;
t810 = t9.*t718;
t811 = t9.*t719;
t812 = t8.*t721;
t813 = t9.*t722;
t833 = t9.*t747;
t834 = t9.*t748;
t835 = t8.*t750;
t836 = t9.*t755;
t879 = t8.*t745;
t880 = t5.*t748;
t965 = -t924;
t987 = t8.*t906;
t1008 = -t956;
t1025 = -t960;
t1032 = -t966;
t1033 = -t967;
t1043 = -t981;
t1051 = -t988;
t1054 = -t992;
t1055 = -t993;
t1056 = -t996;
t1057 = -t995;
t1061 = -t1000;
t1065 = -t1003;
t1073 = -t1007;
t1074 = t8.*t960;
t1083 = -t1014;
t1084 = -t1013;
t1085 = -t1015;
t1095 = -t1029;
t1104 = t8.*t981;
t1121 = t8.*t984;
t1125 = t8.*t994;
t1127 = -t1052;
t1131 = t8.*t999;
t1132 = t8.*t1000;
t1157 = t18.*t906;
t1166 = -t1086;
t1173 = t4.*t190.*7.537489895992698e+48;
t1174 = -t1096;
t1175 = -t1098;
t1179 = -t1103;
t1180 = -t1102;
t1181 = t18.*t960;
t1183 = -t1105;
t1190 = -t1115;
t1191 = -t1117;
t1192 = -t1116;
t1193 = -t1118;
t1197 = -t1126;
t1198 = -t1129;
t1199 = -t1130;
t1203 = -t1137;
t1206 = -t1138;
t1224 = -t1164;
t1230 = t8.*t1118;
t1242 = t8.*t1137;
t1249 = t18.*t984;
t1252 = t8.*t1151;
t1257 = -t1210;
t1262 = -t1218;
t1263 = -t1219;
t1287 = -t1231;
t1290 = -t1238;
t1293 = t3.*t34.*t191.*4.602992943936994e+15;
t1294 = -t1243;
t1295 = -t1244;
t1296 = -t1246;
t1297 = -t1247;
t1299 = t7.*t34.*t191.*4.602992943936994e+15;
t1306 = -t1255;
t1320 = -t1275;
t1323 = -t1281;
t1325 = -t1283;
t1333 = t18.*t1118;
t1342 = -t1310;
t1343 = -t1309;
t1346 = -t1315;
t1350 = t8.*t1283;
t1353 = -t1327;
t1354 = -t1326;
t1355 = -t1329;
t1377 = -t1349;
t1385 = -t1352;
t1386 = -t1357;
t1387 = -t1359;
t1394 = -t1366;
t1397 = -t1370;
t1398 = (t3.*t34.*t191)./9.007199254740992e+15;
t1399 = (t7.*t34.*t191)./9.007199254740992e+15;
t1402 = -t1376;
t1403 = -t1375;
t1406 = -t1378;
t1408 = -t1382;
t1410 = t8.*t1356;
t1412 = t8.*t1358;
t1418 = -t1395;
t1419 = -t1396;
t1427 = t40+t48+t68;
t1429 = t37+t49+t88;
t1431 = -t1415;
t1433 = -t1417;
t1434 = -t1420;
t1435 = t7.*t34.*t191.*6.661338147750939e-19;
t1436 = -t1425;
t1440 = t8.*t1420;
t1445 = -t1438;
t1447 = t3.*t4.*t34.*t191.*6.661338147750939e-19;
t1448 = t3.*t8.*t34.*t191.*6.661338147750939e-19;
t1451 = t7.*t8.*t34.*t191.*(-6.661338147750939e-19);
t1463 = -t1453;
t1469 = -t1462;
t1470 = -t1461;
t1472 = t190.*7.38843356682345e-1;
t1473 = t190.*2.61156643317655e-1;
t1475 = t190.*4.392651260556773e-1;
t1479 = t190.*4.931128922368695e-2;
t1481 = -t1476;
t1483 = -t1478;
t1487 = -t1484;
t1488 = t8.*t190.*1.148695147579899e-4;
t1489 = (t9.*t1460)./2.0;
t1494 = t190.*1.76134094882956e-6;
t1496 = (t5.*t1471)./2.0;
t1497 = t8.*t190.*6.243419149368285e-5;
t1501 = t34.*t191.*8.001214128951626e+33;
t1503 = (t4.*t5.*t1460)./2.0;
t1513 = t4.*t34.*t191.*8.368294830410569e+32;
t1514 = t5.*t190.*6.892170885479394e-7;
t1515 = t8.*t34.*t191.*8.368294830410569e+32;
t1517 = t17.*t190.*1.284980501238441e-6;
t1518 = t8.*t190.*1.805471570026627e-6;
t1519 = t8.*t190.*3.610943140053254e-6;
t1520 = t22.*t190.*1.284980501238441e-6;
t1523 = (t4.*t9.*t1471)./2.0;
t1527 = t3.*t8.*t34.*t191.*4.97520895370488e+32;
t1528 = t4.*t7.*t34.*t191.*4.97520895370488e+32;
t1529 = t7.*t8.*t34.*t191.*4.97520895370488e+32;
t1531 = t46+t626;
t1541 = t8.*t190.*7.558827895633446e-9;
t1542 = t8.*t190.*1.511765579126689e-8;
t1545 = t9.*t190.*3.746051489620971e-7;
t1548 = t17.*t190.*1.11200961038573e-6;
t1550 = t22.*t190.*1.11200961038573e-6;
t1555 = t4.*t9.*t190.*3.446085442739697e-7;
t1556 = t5.*t8.*t190.*3.446085442739697e-7;
t1561 = t44+t104+t172;
t1562 = t3.*t8.*t34.*t191.*9.735556609752802e+32;
t1567 = t5.*t8.*t190.*3.748033925961328e-5;
t1569 = t8.*t9.*t190.*3.748033925961328e-5;
t1570 = t4.*t190.*1.085068132002562e-9;
t1571 = t4.*t190.*2.170136264005124e-9;
t1587 = t59+t629;
t1593 = t5.*t8.*t190.*(-6.892170885479394e-7);
t1620 = t4.*t5.*t190.*1.873025744810486e-7;
t1621 = t8.*t19.*t190.*7.044680628082447e-7;
t1622 = t8.*t24.*t190.*7.044680628082447e-7;
t1623 = t8.*t9.*t190.*1.873025744810486e-7;
t1625 = t4.*t19.*t190.*1.07175327657342e-6;
t1633 = t57+t106+t174;
t1650 = t4.*t5.*t9.*t190.*7.044680628082447e-7;
t1672 = t5.*t8.*t9.*t190.*2.143506553146841e-6;
t1681 = t5.*t22.*t190.*(-6.892170885479394e-7);
t1687 = t8.*t190.*2.7046541903611e-13;
t1704 = t8.*t9.*t190.*(-3.746051489620971e-7);
t1771 = t5.*t9.*t17.*t190.*2.143506553146841e-6;
t1772 = t5.*t9.*t18.*t190.*1.07175327657342e-6;
t1776 = t5.*t9.*t22.*t190.*2.143506553146841e-6;
t1784 = t4.*t8.*t17.*t190.*6.267441153167058e-7;
t1793 = t4.*t8.*t22.*t190.*6.267441153167058e-7;
t1795 = t17.*t18.*t190.*7.175085365598963e-7;
t1803 = t4.*t190.*5.347915701547076e-7;
t1808 = t18.*t22.*t190.*7.175085365598963e-7;
t1811 = t17.*t19.*t190.*1.408936125616489e-6;
t1812 = t18.*t19.*t190.*7.044680628082447e-7;
t1820 = t19.*t22.*t190.*1.408936125616489e-6;
t1855 = t4.*t9.*t17.*t190.*6.892170885479394e-7;
t1888 = t190.*3.93189593030583e-6;
t1908 = t8.*t17.*t190.*(-1.511765579126689e-8);
t1930 = t9.*t22.*t190.*(-3.746051489620971e-7);
t1946 = t8.*t190.*3.546806877605634e-13;
t1964 = t4.*t9.*t190.*1.35232709518055e-13;
t1965 = t5.*t8.*t190.*1.35232709518055e-13;
t1972 = t188.*8.645493468585888e-10;
t1984 = t5.*t8.*t9.*t17.*t190.*4.287013106293682e-6;
t2002 = t4.*t5.*t17.*t190.*3.746051489620971e-7;
t2014 = t8.*t17.*t24.*t190.*1.408936125616489e-6;
t2017 = t4.*t17.*t19.*t190.*2.143506553146841e-6;
t2062 = t4.*t5.*t9.*t17.*t190.*1.408936125616489e-6;
t2096 = t99+t119+t182;
t2097 = t5.*t17.*t18.*t190.*(-6.892170885479394e-7);
t2121 = t100+t105+t181;
t2122 = t18.*t190.*2.536718707310641e-7;
t2126 = t4.*t5.*t190.*1.773403438802817e-13;
t2136 = t8.*t9.*t190.*1.773403438802817e-13;
t2153 = -t7.*t34.*t191.*(t29-t30);
t2154 = t17.*t190.*1.704036655415135e-6;
t2158 = t22.*t190.*1.704036655415135e-6;
t2196 = t4.*t17.*t190.*1.069583140309415e-6;
t2214 = t4.*t8.*t9.*t190.*(-2.7046541903611e-13);
t2225 = -t3.*t34.*t191.*(t29-t30);
t2236 = t4.*t9.*t17.*t190.*2.7046541903611e-13;
t2239 = t5.*t8.*t190.*7.233705477105363e-14;
t2244 = t8.*t9.*t190.*7.233705477105363e-14;
t2254 = t5.*t9.*t17.*t18.*t190.*(-1.07175327657342e-6);
t2264 = t17.*t18.*t19.*t190.*(-7.044680628082447e-7);
t2269 = t9.*t17.*t18.*t190.*(-3.746051489620971e-7);
t2270 = t190.*7.206852993931618e+49;
t2276 = t7.*t34.*t191.*(t29-t30);
t2291 = t4.*t5.*t8.*t190.*(-3.546806877605634e-13);
t2333 = t4.*t5.*t17.*t190.*3.546806877605634e-13;
t2366 = t18.*t22.*t190.*(-2.536718707310641e-7);
t2371 = t8.*t9.*t17.*t190.*(-3.546806877605634e-13);
t2418 = t3.*t34.*t191.*5.673626844500105e-17;
t2419 = t7.*t34.*t191.*5.673626844500105e-17;
t2421 = t4.*t34.*t191.*9.543032792050485e-17;
t2422 = t8.*t34.*t191.*9.543032792050485e-17;
t2442 = t25.*t34.*t191.*2.352289923061441e+15;
t2444 = t26.*t34.*t191.*2.352289923061441e+15;
t2447 = t7.*t34.*t191.*9.007199254740992e+15;
t2449 = t25.*t34.*t191.*3.956548516042405e+15;
t2450 = t26.*t34.*t191.*3.956548516042405e+15;
t2466 = t4.*t8.*t190.*6.267440429796511e-7;
t2467 = t3.*t34.*t191.*3.404176106700063e-19;
t2468 = t7.*t34.*t191.*3.404176106700063e-19;
t2472 = t4.*t7.*t34.*t191.*(-5.673626844500105e-17);
t2477 = t4.*t34.*t191.*5.725819675230291e-19;
t2485 = t7.*t8.*t34.*t191.*3.404176106700063e-19;
t2492 = t7.*t34.*t191.*4.841027578805779e-21;
t2498 = t7.*t34.*t191.*2.952953132824215e-22;
t2499 = t4.*t5.*t34.*t191.*5.725819675230291e-19;
t2500 = t4.*t9.*t34.*t191.*5.725819675230291e-19;
t2501 = t5.*t8.*t34.*t191.*5.725819675230291e-19;
t2503 = t8.*t9.*t34.*t191.*5.725819675230291e-19;
t2504 = t7.*t34.*t191.*8.902051046907267e-23;
t2535 = t4.*t7.*t9.*t34.*t191.*(-3.404176106700063e-19);
t2536 = t5.*t7.*t8.*t34.*t191.*(-3.404176106700063e-19);
t2538 = t7.*t34.*t191.*4.838467028611604e-23;
t2543 = t4.*t8.*t17.*t190.*(-6.267440429796511e-7);
t2546 = t3.*t4.*t34.*t191.*2.331979335274259e-22;
t2549 = t5.*t7.*t34.*t191.*(-8.902051046907267e-23);
t2551 = t3.*t4.*t34.*t191.*9.763117151300172e-25;
t2552 = t3.*t4.*t5.*t34.*t191.*4.451025523453633e-23;
t2553 = t3.*t4.*t5.*t34.*t191.*8.902051046907267e-23;
t2554 = t7.*t19.*t34.*t191.*9.099035355097216e-23;
t2555 = t7.*t8.*t34.*t191.*9.763117151300172e-25;
t2557 = t3.*t8.*t9.*t34.*t191.*4.451025523453633e-23;
t2558 = t4.*t7.*t9.*t34.*t191.*4.451025523453633e-23;
t2559 = t7.*t34.*t191.*1.452308273641734e-23;
t2560 = t5.*t7.*t9.*t34.*t191.*1.384295679297146e-22;
t2561 = t3.*t4.*t5.*t34.*t191.*4.841027578805779e-21;
t2562 = t3.*t4.*t9.*t34.*t191.*4.841027578805779e-21;
t2565 = t7.*t9.*t34.*t191.*(-4.838467028611604e-23);
t2572 = t3.*t5.*t8.*t9.*t34.*t191.*9.099035355097216e-23;
t2573 = t4.*t5.*t7.*t9.*t34.*t191.*9.099035355097216e-23;
t2574 = t3.*t8.*t19.*t34.*t191.*1.384295679297146e-22;
t2575 = t4.*t7.*t19.*t34.*t191.*1.384295679297146e-22;
t2576 = t3.*t4.*t9.*t34.*t191.*2.419233514305802e-23;
t2577 = t3.*t4.*t9.*t34.*t191.*4.838467028611604e-23;
t2578 = t3.*t5.*t8.*t34.*t191.*2.419233514305802e-23;
t2579 = t4.*t5.*t7.*t34.*t191.*2.419233514305802e-23;
t2583 = t3.*t9.*t34.*t191.*1.746689835966788e-29;
t2584 = t5.*t7.*t34.*t191.*1.746689835966788e-29;
t2590 = t2.*t4.*t190.*2.227619671697157e-2;
t2591 = t2.*t8.*t190.*2.227619671697157e-2;
t2592 = t4.*t6.*t190.*2.227619671697157e-2;
t2593 = t6.*t8.*t190.*2.227619671697157e-2;
t2595 = t4.*t190.*5.088811214040866e-2;
t2596 = t8.*t190.*5.088811214040866e-2;
t2597 = t3.*t4.*t5.*t8.*t9.*t34.*t191.*1.384295679297146e-22;
t2602 = t2.*t4.*t190.*9.189001945180305e-2;
t2603 = t2.*t8.*t190.*9.189001945180305e-2;
t2604 = t4.*t6.*t190.*9.189001945180305e-2;
t2605 = t6.*t8.*t190.*9.189001945180305e-2;
t2609 = t3.*t8.*t34.*t191.*6.907463462641287e-23;
t2610 = t4.*t7.*t34.*t191.*6.907463462641287e-23;
t2611 = t3.*t4.*t8.*t19.*t34.*t191.*9.099035355097216e-23;
t2615 = t3.*t4.*t5.*t34.*t191.*1.746689835966788e-29;
t2617 = t7.*t9.*t34.*t191.*2.290559564076375e-29;
t2627 = t7.*t34.*t191.*2.589914296704185e-22;
t2652 = t3.*t5.*t34.*t191.*2.290559564076375e-29;
t2655 = t3.*t8.*t9.*t34.*t191.*(-1.746689835966788e-29);
t2656 = t5.*t7.*t8.*t34.*t191.*(-1.746689835966788e-29);
t2673 = t2.*t5.*t8.*t190.*(-2.227619671697157e-2);
t2675 = t2.*t8.*t9.*t190.*(-2.227619671697157e-2);
t2676 = t4.*t6.*t9.*t190.*(-2.227619671697157e-2);
t2685 = t8.*t9.*t190.*(-5.088811214040866e-2);
t2687 = t3.*t4.*t8.*t34.*t191.*3.276471201795111e-23;
t2705 = t2.*t4.*t5.*t190.*(-9.189001945180305e-2);
t2706 = t3.*t9.*t18.*t34.*t191.*3.493379671933577e-29;
t2707 = t5.*t6.*t8.*t190.*(-9.189001945180305e-2);
t2708 = t6.*t8.*t9.*t190.*(-9.189001945180305e-2);
t2716 = t3.*t4.*t9.*t34.*t191.*2.290559564076375e-29;
t2719 = t5.*t8.*t190.*(-5.088811214040866e-2);
t2749 = t3.*t5.*t8.*t34.*t191.*(-2.290559564076375e-29);
t2751 = t3.*t4.*t5.*t34.*t191.*9.343183227095153e-30;
t2752 = t3.*t4.*t9.*t34.*t191.*9.343183227095153e-30;
t2764 = t3.*t5.*t18.*t34.*t191.*4.58111912815275e-29;
t2804 = t190.*5.271069685603861e-14;
t2854 = t6.*t190.*4.472183499114333e-13;
t2939 = t2.*t190.*1.844789907123413e-12;
t3058 = t3.*t18.*t34.*t191.*8.095138029302968e-23;
t3142 = (t318.*t638)./2.0;
t3158 = t3.*t34.*t191.*(t29-t30).*(-1.232595164407831e-32);
t3191 = t34.*t191.*5.474652867008761e-18;
t3208 = t2.*t3.*t34.*t191.*2.877233365226343e-18;
t3211 = t2.*t7.*t34.*t191.*2.877233365226343e-18;
t3212 = t6.*t7.*t34.*t191.*2.877233365226343e-18;
t3218 = t25.*t34.*t191.*2.899421184450801e-17;
t3219 = t26.*t34.*t191.*2.899421184450801e-17;
t3225 = t4.*t34.*t191.*1.275307801118396e-20;
t3228 = t8.*t34.*t191.*1.275307801118396e-20;
t3230 = t25.*t34.*t191.*4.876822568618848e-17;
t3231 = t26.*t34.*t191.*4.876822568618848e-17;
t3243 = t25.*t34.*t191.*8.202809061800765e-17;
t3244 = t26.*t34.*t191.*8.202809061800765e-17;
t3251 = t2.*t7.*t34.*t191.*1.186867907736671e-17;
t3252 = t3.*t6.*t34.*t191.*1.186867907736671e-17;
t3255 = t6.*t7.*t34.*t191.*1.186867907736671e-17;
t3257 = t3.*t34.*t191.*9.827649182848514e-18;
t3258 = t7.*t34.*t191.*9.827649182848514e-18;
t3259 = t7.*t34.*t191.*4.549258542705501e-23;
t3261 = t3.*t6.*t8.*t34.*t191.*2.877233365226343e-18;
t3273 = t4.*t34.*t191.*2.004476107349692e-22;
t3274 = t4.*t34.*t191.*4.008952214699383e-22;
t3275 = t8.*t34.*t191.*4.008952214699383e-22;
t3279 = t3.*t34.*t191.*4.549258542705501e-23;
t3282 = t3.*t4.*t6.*t34.*t191.*2.877233365226343e-18;
t3286 = t2.*t7.*t8.*t34.*t191.*(-2.877233365226343e-18);
t3288 = t2.*t7.*t9.*t34.*t191.*(-2.877233365226343e-18);
t3289 = t5.*t6.*t7.*t34.*t191.*(-2.877233365226343e-18);
t3290 = t6.*t7.*t9.*t34.*t191.*(-2.877233365226343e-18);
t3294 = t2.*t3.*t4.*t34.*t191.*1.186867907736671e-17;
t3295 = t2.*t3.*t8.*t34.*t191.*1.186867907736671e-17;
t3309 = t4.*t34.*t191.*6.93158769201428e-21;
t3314 = t8.*t34.*t191.*6.93158769201428e-21;
t3317 = t3.*t34.*t191.*2.47393392290267e-21;
t3319 = t7.*t34.*t191.*2.47393392290267e-21;
t3320 = t2.*t4.*t7.*t34.*t191.*(-2.877233365226343e-18);
t3321 = t9.*t34.*t191.*7.651846806710377e-23;
t3326 = t4.*t6.*t7.*t34.*t191.*(-1.186867907736671e-17);
t3327 = t6.*t7.*t8.*t34.*t191.*(-1.186867907736671e-17);
t3328 = t6.*t7.*t9.*t34.*t191.*(-1.186867907736671e-17);
t3329 = t3.*t34.*t191.*1.509062034684317e-22;
t3330 = t7.*t34.*t191.*1.509062034684317e-22;
t3331 = t4.*t7.*t34.*t191.*(-9.827649182848514e-18);
t3333 = t3.*t4.*t34.*t191.*1.19172276776539e-22;
t3334 = t7.*t8.*t34.*t191.*(-9.827649182848514e-18);
t3335 = t7.*t9.*t34.*t191.*(-9.827649182848514e-18);
t3343 = t7.*t8.*t34.*t191.*1.19172276776539e-22;
t3363 = t3.*t34.*t191.*2.472625392454631e-23;
t3364 = t7.*t34.*t191.*2.472625392454631e-23;
t3365 = t5.*t7.*t34.*t191.*(-4.549258542705501e-23);
t3367 = t3.*t6.*t8.*t9.*t34.*t191.*(-2.877233365226343e-18);
t3368 = t7.*t8.*t34.*t191.*9.978586703210931e-25;
t3369 = t7.*t8.*t34.*t191.*9.978586703210931e-25;
t3370 = t4.*t5.*t34.*t191.*4.161153561678485e-21;
t3371 = t4.*t9.*t34.*t191.*4.161153561678485e-21;
t3372 = t5.*t8.*t34.*t191.*4.161153561678485e-21;
t3373 = t8.*t9.*t34.*t191.*4.161153561678485e-21;
t3374 = t2.*t3.*t5.*t8.*t34.*t191.*(-1.186867907736671e-17);
t3375 = t3.*t5.*t9.*t34.*t191.*9.299848787979342e-23;
t3376 = t5.*t7.*t9.*t34.*t191.*7.074233692313782e-23;
t3378 = t4.*t34.*t191.*8.391984768911171e-25;
t3379 = t4.*t34.*t191.*1.678396953782234e-24;
t3380 = t4.*t34.*t191.*1.678396953782234e-24;
t3381 = t8.*t34.*t191.*1.678396953782234e-24;
t3382 = t5.*t34.*t191.*4.158952615208568e-23;
t3389 = t3.*t19.*t34.*t191.*7.074233692313782e-23;
t3390 = t4.*t5.*t34.*t191.*3.825923403355188e-23;
t3391 = t4.*t5.*t34.*t191.*7.651846806710377e-23;
t3392 = t3.*t24.*t34.*t191.*7.074233692313782e-23;
t3393 = t5.*t8.*t34.*t191.*7.651846806710377e-23;
t3394 = t7.*t19.*t34.*t191.*4.649924393989671e-23;
t3395 = t3.*t4.*t34.*t191.*9.978586703210931e-25;
t3397 = t7.*t8.*t34.*t191.*4.989293351605466e-25;
t3400 = t4.*t5.*t9.*t34.*t191.*2.379770328738529e-22;
t3401 = t7.*t34.*t191.*7.42180176870801e-24;
t3402 = t4.*t34.*t191.*2.409335246872506e-25;
t3403 = t8.*t34.*t191.*2.409335246872506e-25;
t3409 = t3.*t4.*t5.*t34.*t191.*2.27462927135275e-23;
t3416 = t4.*t5.*t8.*t34.*t191.*1.530369361342075e-22;
t3417 = t3.*t8.*t9.*t34.*t191.*2.27462927135275e-23;
t3418 = t4.*t7.*t9.*t34.*t191.*(-4.549258542705501e-23);
t3419 = t4.*t7.*t9.*t34.*t191.*2.27462927135275e-23;
t3420 = t5.*t7.*t8.*t34.*t191.*2.27462927135275e-23;
t3426 = t3.*t4.*t34.*t191.*4.989293351605466e-25;
t3430 = t3.*t4.*t5.*t9.*t34.*t191.*1.414846738462756e-22;
C_dq = ft_4({dq1,dq2,dq3,dq4,dq5,dq6,t1003,t1004,t1006,t1008,t101,t1012,t1013,t1015,t1016,t102,t1023,t1024,t1025,t1026,t1027,t1028,t1030,t1032,t1033,t1034,t1038,t1039,t104,t1040,t1041,t1042,t1043,t1044,t1045,t1047,t1048,t1049,t1050,t1051,t1054,t1055,t1056,t1057,t1058,t1059,t106,t1061,t1062,t1063,t1064,t1065,t1066,t1068,t1069,t107,t1070,t1071,t1073,t1078,t108,t1080,t1081,t1083,t1084,t1085,t109,t1091,t1092,t1093,t1094,t1095,t1097,t1098,t1099,t110,t1100,t1101,t1102,t1105,t1106,t1108,t1109,t111,t1111,t1113,t1115,t1116,t1119,t112,t1123,t1125,t1126,t1127,t1128,t1129,t113,t1130,t1131,t1132,t1133,t1134,t1138,t1139,t114,t1140,t1141,t1144,t115,t1150,t1151,t1152,t1153,t1155,t1158,t1159,t116,t1161,t1162,t1163,t1166,t1167,t1169,t117,t1170,t1171,t1173,t1174,t1175,t1176,t1177,t1178,t1179,t118,t1180,t1181,t1182,t1183,t1185,t1186,t1187,t1188,t1189,t1190,t1191,t1192,t1193,t1195,t1196,t1197,t1198,t1199,t120,t1203,t1204,t1205,t1206,t1207,t1208,t121,t1210,t1214,t1215,t1216,t1219,t122,t1221,t1222,t1223,t1224,t1225,t1226,t1229,t123,t1230,t1232,t1233,t1236,t124,t1240,t1242,t1244,t1245,t125,t1250,t1251,t1253,t1254,t1256,t1257,t1258,t1259,t126,t1260,t1261,t1262,t1263,t1264,t1266,t1272,t1273,t1274,t1276,t1278,t1279,t128,t1280,t1282,t1284,t1285,t1286,t1287,t1288,t129,t1290,t1293,t1294,t1295,t1296,t1297,t1298,t1299,t130,t1300,t1301,t1302,t1304,t1306,t1307,t1308,t1309,t131,t1312,t1313,t1315,t1316,t1319,t132,t1320,t1321,t1322,t1323,t1324,t1325,t1326,t1328,t1329,t133,t1330,t1331,t1332,t1333,t1335,t1337,t1338,t1339,t134,t1340,t1341,t1342,t1343,t1344,t1345,t1346,t1347,t1348,t135,t1351,t1352,t1353,t1354,t1355,t1356,t1358,t136,t1360,t1362,t1364,t1365,t1366,t1367,t1368,t1369,t1370,t1371,t1372,t1373,t1374,t1375,t1377,t1378,t1379,t1380,t1382,t1383,t1384,t1385,t1386,t1387,t1388,t1389,t139,t1391,t1392,t1393,t1394,t1397,t1398,t1399,t140,t1401,t1402,t1403,t1404,t1405,t1406,t1407,t1408,t1409,t141,t1410,t1411,t1413,t1414,t1415,t1416,t1417,t1418,t1419,t142,t1421,t1423,t1424,t1426,t1427,t1428,t1429,t143,t1431,t1433,t1434,t1435,t1436,t144,t1440,t1443,t1444,t1445,t1447,t1448,t1449,t145,t1451,t1453,t1454,t1456,t1457,t1460,t1461,t1463,t1464,t1469,t147,t1470,t1471,t1472,t1473,t1475,t1476,t1478,t1479,t148,t1481,t1482,t1483,t1485,t1486,t1487,t1488,t1489,t1494,t1496,t1497,t15,t150,t1501,t1503,t1505,t151,t1513,t1514,t1515,t1517,t1518,t1519,t152,t1520,t1521,t1522,t1523,t1527,t1528,t1529,t153,t1531,t1532,t1533,t1535,t154,t1541,t1542,t1545,t1548,t1549,t155,t1550,t1555,t1556,t1558,t156,t1560,t1561,t1562,t1566,t1567,t1568,t1569,t157,t1570,t1571,t158,t1580,t1587,t1589,t1591,t1593,t1595,t1596,t1597,t1598,t1599,t16,t1605,t1606,t161,t1610,t1611,t1612,t1619,t162,t1620,t1621,t1622,t1623,t1625,t163,t1631,t1632,t1633,t1635,t1636,t1637,t1638,t1639,t1641,t1643,t1644,t1645,t165,t1650,t1651,t1652,t1653,t1657,t1658,t1659,t166,t1660,t1661,t1662,t1663,t1666,t1669,t1672,t1676,t168,t1681,t1682,t1683,t1687,t1689,t169,t1692,t1695,t1696,t1698,t17,t170,t1702,t1703,t1704,t1709,t171,t1711,t1712,t1713,t1716,t1720,t1722,t1726,t1728,t1729,t173,t1731,t1733,t1734,t1735,t1736,t1737,t1738,t1740,t1744,t1745,t1746,t1749,t175,t1752,t1755,t1756,t1757,t1758,t176,t1760,t1761,t1764,t1767,t1769,t177,t1771,t1772,t1774,t1776,t1779,t1784,t1785,t1786,t1787,t1788,t1789,t179,t1793,t1795,t1797,t1798,t1799,t18,t180,t1800,t1801,t1803,t1804,t1807,t1808,t1809,t181,t1810,t1811,t1812,t1814,t1816,t1817,t182,t1820,t1826,t1827,t1829,t183,t1830,t1831,t1832,t1833,t1834,t1835,t1836,t1838,t1847,t1849,t185,t1850,t1851,t1855,t1857,t1858,t1859,t186,t1866,t1867,t1871,t1872,t1873,t1881,t1882,t1888,t1889,t1896,t19,t190,t1903,t1907,t1908,t191,t1910,t1911,t1912,t1913,t1914,t1915,t1916,t1920,t1925,t1926,t193,t1930,t1935,t1936,t1937,t1938,t1939,t194,t1943,t1944,t1946,t195,t1950,t1955,t196,t1961,t1964,t1965,t1966,t1967,t1968,t1969,t197,t1970,t1972,t1976,t1977,t1978,t1979,t198,t1981,t1984,t1988,t1992,t1994,t1995,t1996,t1997,t1998,t1999,t2,t20,t2000,t2001,t2002,t2003,t2004,t2005,t2006,t2014,t2017,t2019,t2020,t2023,t2024,t2028,t2029,t2033,t2036,t2037,t2038,t2042,t2052,t2053,t2056,t2058,t2059,t206,t2060,t2062,t2065,t2066,t2067,t2068,t2069,t207,t2070,t2072,t2073,t2074,t2079,t2081,t2082,t2083,t2084,t2085,t2086,t2087,t2093,t2094,t2096,t2097,t2098,t21,t2100,t2103,t2104,t2105,t2106,t2108,t2109,t2110,t2111,t2113,t2114,t2115,t2116,t2117,t2118,t2121,t2122,t2126,t2128,t2129,t2130,t2131,t2132,t2133,t2136,t2142,t2144,t2148,t2149,t215,t2154,t2156,t2157,t2158,t216,t2171,t2172,t2175,t2176,t2179,t2180,t2182,t2189,t219,t2194,t2196,t22,t220,t2204,t2208,t221,t2212,t2214,t2217,t2218,t2219,t222,t2220,t2221,t2223,t2225,t2227,t2228,t2229,t223,t2236,t2239,t224,t2244,t225,t2251,t2254,t2256,t2257,t226,t2264,t2265,t2266,t2267,t2269,t227,t2270,t2274,t2276,t2277,t2279,t228,t2280,t2281,t2282,t2285,t2291,t2294,t23,t230,t2302,t2304,t2305,t2306,t231,t2316,t2317,t2318,t2321,t2322,t2323,t2324,t233,t2333,t2336,t2339,t234,t2340,t2344,t2348,t235,t2350,t2357,t2358,t2359,t236,t2361,t2362,t2363,t2364,t2365,t2366,t2369,t237,t2371,t2372,t2373,t2375,t2376,t2377,t2378,t2379,t238,t2384,t2385,t2387,t2388,t2389,t239,t2391,t2394,t24,t240,t2400,t2401,t2402,t2403,t2405,t2406,t2407,t241,t2410,t2417,t2418,t2419,t242,t2421,t2422,t2428,t2429,t243,t2430,t2431,t2434,t2435,t2437,t2438,t2439,t244,t2440,t2441,t2442,t2443,t2444,t2447,t2449,t245,t2450,t2452,t2453,t2454,t2455,t2456,t2457,t2458,t246,t2460,t2466,t2467,t2468,t247,t2470,t2472,t2474,t2477,t248,t2481,t2483,t2484,t2485,t2486,t2487,t2489,t249,t2492,t2495,t2497,t2498,t2499,t25,t2500,t2501,t2502,t2503,t2504,t2505,t2506,t2513,t2518,t2521,t2527,t253,t2533,t2535,t2536,t2537,t2538,t254,t2540,t2543,t2544,t2545,t2546,t2549,t2551,t2552,t2553,t2554,t2555,t2557,t2558,t2559,t256,t2560,t2561,t2562,t2565,t257,t2572,t2573,t2574,t2575,t2576,t2577,t2578,t2579,t258,t2583,t2584,t259,t2590,t2591,t2592,t2593,t2595,t2596,t2597,t26,t260,t2602,t2603,t2604,t2605,t2609,t261,t2610,t2611,t2615,t2617,t2627,t263,t264,t2652,t2655,t2656,t266,t2673,t2675,t2676,t2685,t2687,t269,t270,t2705,t2706,t2707,t2708,t2716,t2719,t272,t273,t274,t2749,t275,t2751,t2752,t276,t2764,t277,t278,t279,t280,t2804,t281,t284,t285,t2854,t286,t287,t288,t2886,t289,t29,t290,t291,t292,t293,t2939,t294,t296,t297,t299,t2997,t3,t30,t300,t302,t303,t304,t305,t3058,t306,t307,t308,t309,t31,t310,t311,t312,t313,t314,t3142,t315,t3158,t316,t318,t319,t3191,t32,t320,t3208,t321,t3211,t3212,t3218,t3219,t322,t3225,t3228,t3230,t3231,t324,t3243,t3244,t325,t3251,t3252,t3255,t3257,t3258,t3259,t3261,t3273,t3274,t3275,t3279,t328,t3282,t3286,t3288,t3289,t329,t3290,t3294,t3295,t33,t3309,t3314,t3317,t3319,t332,t3320,t3321,t3326,t3327,t3328,t3329,t333,t3330,t3331,t3333,t3334,t3335,t334,t3343,t336,t3363,t3364,t3365,t3367,t3368,t3369,t337,t3370,t3371,t3372,t3373,t3374,t3375,t3376,t3378,t3379,t3380,t3381,t3382,t3389,t3390,t3391,t3392,t3393,t3394,t3395,t3397,t34,t340,t3400,t3401,t3402,t3403,t3409,t341,t3416,t3417,t3418,t3419,t3420,t3426,t3430,t344,t345,t346,t347,t348,t349,t350,t352,t353,t354,t355,t356,t357,t358,t359,t360,t361,t362,t365,t366,t367,t368,t369,t371,t372,t373,t374,t375,t376,t377,t378,t379,t380,t382,t384,t386,t387,t388,t389,t391,t392,t395,t396,t398,t4,t400,t401,t402,t403,t404,t406,t409,t410,t411,t412,t413,t414,t415,t416,t417,t418,t419,t420,t421,t422,t423,t424,t425,t426,t427,t428,t429,t431,t432,t433,t434,t435,t436,t437,t438,t439,t44,t440,t441,t442,t443,t444,t445,t448,t449,t45,t450,t452,t453,t454,t457,t458,t459,t46,t460,t461,t462,t463,t464,t465,t466,t468,t469,t47,t470,t471,t472,t475,t4763,t477,t479,t480,t481,t482,t483,t484,t485,t486,t488,t489,t491,t492,t493,t494,t496,t497,t498,t499,t5,t50,t500,t501,t502,t503,t504,t505,t506,t507,t508,t509,t510,t511,t512,t513,t514,t516,t517,t518,t520,t521,t522,t523,t524,t525,t526,t527,t528,t529,t53,t530,t531,t532,t533,t534,t535,t536,t5361,t537,t538,t539,t540,t543,t544,t545,t546,t547,t548,t549,t551,t552,t553,t554,t555,t556,t557,t558,t559,t560,t561,t562,t563,t564,t567,t568,t569,t57,t570,t571,t572,t573,t574,t576,t577,t5777,t578,t579,t58,t580,t581,t582,t583,t584,t586,t587,t589,t59,t590,t591,t592,t593,t594,t595,t596,t597,t6,t60,t600,t602,t603,t604,t605,t609,t610,t611,t612,t613,t614,t615,t617,t618,t623,t625,t626,t629,t63,t633,t634,t638,t640,t643,t644,t655,t656,t660,t662,t663,t664,t665,t667,t668,t673,t674,t675,t676,t681,t682,t683,t685,t686,t687,t688,t689,t693,t694,t695,t696,t697,t698,t7,t700,t702,t703,t704,t705,t706,t71,t711,t713,t715,t716,t72,t724,t725,t727,t728,t73,t731,t733,t734,t735,t736,t74,t744,t746,t747,t748,t749,t75,t750,t751,t752,t755,t756,t757,t758,t759,t76,t762,t763,t764,t765,t766,t768,t769,t77,t772,t774,t775,t776,t780,t782,t785,t786,t788,t791,t793,t795,t8,t80,t804,t805,t806,t808,t81,t814,t815,t816,t818,t819,t82,t820,t821,t822,t825,t827,t83,t833,t834,t835,t836,t837,t838,t84,t840,t841,t842,t843,t846,t851,t855,t857,t86,t862,t864,t874,t880,t882,t884,t885,t888,t891,t892,t895,t897,t899,t9,t90,t900,t903,t904,t906,t91,t911,t921,t922,t923,t926,t927,t934,t935,t936,t937,t940,t941,t942,t946,t949,t95,t950,t956,t957,t958,t961,t962,t964,t965,t966,t968,t969,t97,t970,t971,t972,t977,t979,t982,t983,t984,t986,t987,t988,t989,t99,t993,t994,t995,t997,t999});
end
function C_dq = ft_4(ct)
dq1 = ct{1};
dq2 = ct{2};
dq3 = ct{3};
dq4 = ct{4};
dq5 = ct{5};
dq6 = ct{6};
t1003 = ct{7};
t1004 = ct{8};
t1006 = ct{9};
t1008 = ct{10};
t101 = ct{11};
t1012 = ct{12};
t1013 = ct{13};
t1015 = ct{14};
t1016 = ct{15};
t102 = ct{16};
t1023 = ct{17};
t1024 = ct{18};
t1025 = ct{19};
t1026 = ct{20};
t1027 = ct{21};
t1028 = ct{22};
t1030 = ct{23};
t1032 = ct{24};
t1033 = ct{25};
t1034 = ct{26};
t1038 = ct{27};
t1039 = ct{28};
t104 = ct{29};
t1040 = ct{30};
t1041 = ct{31};
t1042 = ct{32};
t1043 = ct{33};
t1044 = ct{34};
t1045 = ct{35};
t1047 = ct{36};
t1048 = ct{37};
t1049 = ct{38};
t1050 = ct{39};
t1051 = ct{40};
t1054 = ct{41};
t1055 = ct{42};
t1056 = ct{43};
t1057 = ct{44};
t1058 = ct{45};
t1059 = ct{46};
t106 = ct{47};
t1061 = ct{48};
t1062 = ct{49};
t1063 = ct{50};
t1064 = ct{51};
t1065 = ct{52};
t1066 = ct{53};
t1068 = ct{54};
t1069 = ct{55};
t107 = ct{56};
t1070 = ct{57};
t1071 = ct{58};
t1073 = ct{59};
t1078 = ct{60};
t108 = ct{61};
t1080 = ct{62};
t1081 = ct{63};
t1083 = ct{64};
t1084 = ct{65};
t1085 = ct{66};
t109 = ct{67};
t1091 = ct{68};
t1092 = ct{69};
t1093 = ct{70};
t1094 = ct{71};
t1095 = ct{72};
t1097 = ct{73};
t1098 = ct{74};
t1099 = ct{75};
t110 = ct{76};
t1100 = ct{77};
t1101 = ct{78};
t1102 = ct{79};
t1105 = ct{80};
t1106 = ct{81};
t1108 = ct{82};
t1109 = ct{83};
t111 = ct{84};
t1111 = ct{85};
t1113 = ct{86};
t1115 = ct{87};
t1116 = ct{88};
t1119 = ct{89};
t112 = ct{90};
t1123 = ct{91};
t1125 = ct{92};
t1126 = ct{93};
t1127 = ct{94};
t1128 = ct{95};
t1129 = ct{96};
t113 = ct{97};
t1130 = ct{98};
t1131 = ct{99};
t1132 = ct{100};
t1133 = ct{101};
t1134 = ct{102};
t1138 = ct{103};
t1139 = ct{104};
t114 = ct{105};
t1140 = ct{106};
t1141 = ct{107};
t1144 = ct{108};
t115 = ct{109};
t1150 = ct{110};
t1151 = ct{111};
t1152 = ct{112};
t1153 = ct{113};
t1155 = ct{114};
t1158 = ct{115};
t1159 = ct{116};
t116 = ct{117};
t1161 = ct{118};
t1162 = ct{119};
t1163 = ct{120};
t1166 = ct{121};
t1167 = ct{122};
t1169 = ct{123};
t117 = ct{124};
t1170 = ct{125};
t1171 = ct{126};
t1173 = ct{127};
t1174 = ct{128};
t1175 = ct{129};
t1176 = ct{130};
t1177 = ct{131};
t1178 = ct{132};
t1179 = ct{133};
t118 = ct{134};
t1180 = ct{135};
t1181 = ct{136};
t1182 = ct{137};
t1183 = ct{138};
t1185 = ct{139};
t1186 = ct{140};
t1187 = ct{141};
t1188 = ct{142};
t1189 = ct{143};
t1190 = ct{144};
t1191 = ct{145};
t1192 = ct{146};
t1193 = ct{147};
t1195 = ct{148};
t1196 = ct{149};
t1197 = ct{150};
t1198 = ct{151};
t1199 = ct{152};
t120 = ct{153};
t1203 = ct{154};
t1204 = ct{155};
t1205 = ct{156};
t1206 = ct{157};
t1207 = ct{158};
t1208 = ct{159};
t121 = ct{160};
t1210 = ct{161};
t1214 = ct{162};
t1215 = ct{163};
t1216 = ct{164};
t1219 = ct{165};
t122 = ct{166};
t1221 = ct{167};
t1222 = ct{168};
t1223 = ct{169};
t1224 = ct{170};
t1225 = ct{171};
t1226 = ct{172};
t1229 = ct{173};
t123 = ct{174};
t1230 = ct{175};
t1232 = ct{176};
t1233 = ct{177};
t1236 = ct{178};
t124 = ct{179};
t1240 = ct{180};
t1242 = ct{181};
t1244 = ct{182};
t1245 = ct{183};
t125 = ct{184};
t1250 = ct{185};
t1251 = ct{186};
t1253 = ct{187};
t1254 = ct{188};
t1256 = ct{189};
t1257 = ct{190};
t1258 = ct{191};
t1259 = ct{192};
t126 = ct{193};
t1260 = ct{194};
t1261 = ct{195};
t1262 = ct{196};
t1263 = ct{197};
t1264 = ct{198};
t1266 = ct{199};
t1272 = ct{200};
t1273 = ct{201};
t1274 = ct{202};
t1276 = ct{203};
t1278 = ct{204};
t1279 = ct{205};
t128 = ct{206};
t1280 = ct{207};
t1282 = ct{208};
t1284 = ct{209};
t1285 = ct{210};
t1286 = ct{211};
t1287 = ct{212};
t1288 = ct{213};
t129 = ct{214};
t1290 = ct{215};
t1293 = ct{216};
t1294 = ct{217};
t1295 = ct{218};
t1296 = ct{219};
t1297 = ct{220};
t1298 = ct{221};
t1299 = ct{222};
t130 = ct{223};
t1300 = ct{224};
t1301 = ct{225};
t1302 = ct{226};
t1304 = ct{227};
t1306 = ct{228};
t1307 = ct{229};
t1308 = ct{230};
t1309 = ct{231};
t131 = ct{232};
t1312 = ct{233};
t1313 = ct{234};
t1315 = ct{235};
t1316 = ct{236};
t1319 = ct{237};
t132 = ct{238};
t1320 = ct{239};
t1321 = ct{240};
t1322 = ct{241};
t1323 = ct{242};
t1324 = ct{243};
t1325 = ct{244};
t1326 = ct{245};
t1328 = ct{246};
t1329 = ct{247};
t133 = ct{248};
t1330 = ct{249};
t1331 = ct{250};
t1332 = ct{251};
t1333 = ct{252};
t1335 = ct{253};
t1337 = ct{254};
t1338 = ct{255};
t1339 = ct{256};
t134 = ct{257};
t1340 = ct{258};
t1341 = ct{259};
t1342 = ct{260};
t1343 = ct{261};
t1344 = ct{262};
t1345 = ct{263};
t1346 = ct{264};
t1347 = ct{265};
t1348 = ct{266};
t135 = ct{267};
t1351 = ct{268};
t1352 = ct{269};
t1353 = ct{270};
t1354 = ct{271};
t1355 = ct{272};
t1356 = ct{273};
t1358 = ct{274};
t136 = ct{275};
t1360 = ct{276};
t1362 = ct{277};
t1364 = ct{278};
t1365 = ct{279};
t1366 = ct{280};
t1367 = ct{281};
t1368 = ct{282};
t1369 = ct{283};
t1370 = ct{284};
t1371 = ct{285};
t1372 = ct{286};
t1373 = ct{287};
t1374 = ct{288};
t1375 = ct{289};
t1377 = ct{290};
t1378 = ct{291};
t1379 = ct{292};
t1380 = ct{293};
t1382 = ct{294};
t1383 = ct{295};
t1384 = ct{296};
t1385 = ct{297};
t1386 = ct{298};
t1387 = ct{299};
t1388 = ct{300};
t1389 = ct{301};
t139 = ct{302};
t1391 = ct{303};
t1392 = ct{304};
t1393 = ct{305};
t1394 = ct{306};
t1397 = ct{307};
t1398 = ct{308};
t1399 = ct{309};
t140 = ct{310};
t1401 = ct{311};
t1402 = ct{312};
t1403 = ct{313};
t1404 = ct{314};
t1405 = ct{315};
t1406 = ct{316};
t1407 = ct{317};
t1408 = ct{318};
t1409 = ct{319};
t141 = ct{320};
t1410 = ct{321};
t1411 = ct{322};
t1413 = ct{323};
t1414 = ct{324};
t1415 = ct{325};
t1416 = ct{326};
t1417 = ct{327};
t1418 = ct{328};
t1419 = ct{329};
t142 = ct{330};
t1421 = ct{331};
t1423 = ct{332};
t1424 = ct{333};
t1426 = ct{334};
t1427 = ct{335};
t1428 = ct{336};
t1429 = ct{337};
t143 = ct{338};
t1431 = ct{339};
t1433 = ct{340};
t1434 = ct{341};
t1435 = ct{342};
t1436 = ct{343};
t144 = ct{344};
t1440 = ct{345};
t1443 = ct{346};
t1444 = ct{347};
t1445 = ct{348};
t1447 = ct{349};
t1448 = ct{350};
t1449 = ct{351};
t145 = ct{352};
t1451 = ct{353};
t1453 = ct{354};
t1454 = ct{355};
t1456 = ct{356};
t1457 = ct{357};
t1460 = ct{358};
t1461 = ct{359};
t1463 = ct{360};
t1464 = ct{361};
t1469 = ct{362};
t147 = ct{363};
t1470 = ct{364};
t1471 = ct{365};
t1472 = ct{366};
t1473 = ct{367};
t1475 = ct{368};
t1476 = ct{369};
t1478 = ct{370};
t1479 = ct{371};
t148 = ct{372};
t1481 = ct{373};
t1482 = ct{374};
t1483 = ct{375};
t1485 = ct{376};
t1486 = ct{377};
t1487 = ct{378};
t1488 = ct{379};
t1489 = ct{380};
t1494 = ct{381};
t1496 = ct{382};
t1497 = ct{383};
t15 = ct{384};
t150 = ct{385};
t1501 = ct{386};
t1503 = ct{387};
t1505 = ct{388};
t151 = ct{389};
t1513 = ct{390};
t1514 = ct{391};
t1515 = ct{392};
t1517 = ct{393};
t1518 = ct{394};
t1519 = ct{395};
t152 = ct{396};
t1520 = ct{397};
t1521 = ct{398};
t1522 = ct{399};
t1523 = ct{400};
t1527 = ct{401};
t1528 = ct{402};
t1529 = ct{403};
t153 = ct{404};
t1531 = ct{405};
t1532 = ct{406};
t1533 = ct{407};
t1535 = ct{408};
t154 = ct{409};
t1541 = ct{410};
t1542 = ct{411};
t1545 = ct{412};
t1548 = ct{413};
t1549 = ct{414};
t155 = ct{415};
t1550 = ct{416};
t1555 = ct{417};
t1556 = ct{418};
t1558 = ct{419};
t156 = ct{420};
t1560 = ct{421};
t1561 = ct{422};
t1562 = ct{423};
t1566 = ct{424};
t1567 = ct{425};
t1568 = ct{426};
t1569 = ct{427};
t157 = ct{428};
t1570 = ct{429};
t1571 = ct{430};
t158 = ct{431};
t1580 = ct{432};
t1587 = ct{433};
t1589 = ct{434};
t1591 = ct{435};
t1593 = ct{436};
t1595 = ct{437};
t1596 = ct{438};
t1597 = ct{439};
t1598 = ct{440};
t1599 = ct{441};
t16 = ct{442};
t1605 = ct{443};
t1606 = ct{444};
t161 = ct{445};
t1610 = ct{446};
t1611 = ct{447};
t1612 = ct{448};
t1619 = ct{449};
t162 = ct{450};
t1620 = ct{451};
